simulink model "Dyn_Nonlinear_four"  (R2021a)
(part 6 of 7)

C(2,5) = 0.014*thetad1*cos(theta5)*sin(theta2) - 0.1*thetad5*cos(theta1) - 0.7*thetad4*sin(theta1) - 0.7*thetad5*sin(theta1) - 0.1*thetad4*cos(theta1) + 2.82*thetad4*cos(theta2)*sin(theta2) + 2.82*thetad5*cos(theta2)*sin(theta2) + 2.82*thetad4*cos(theta3)*sin(theta3) + 2.82*thetad5*cos(theta3)*sin(theta3) + 2.82*thetad4*cos(theta4)*sin(theta4) + 2.82*thetad5*cos(theta4)*sin(theta4) - 0.07*thetad1*sin(theta2)*sin(theta5) + 0.2*thetad4*cos(theta1)*cos(theta2)^2 + 0.2*thetad4*cos(theta1)*cos(theta3)^2 + 0.2*thetad5*cos(theta1)*cos(theta2)^2 + 0.2*thetad4*cos(theta1)*cos(theta4)^2 + 0.2*thetad5*cos(theta1)*cos(theta3)^2 + 0.2*thetad5*cos(theta1)*cos(theta4)^2 + 1.4*thetad4*cos(theta2)^2*sin(theta1) + 1.4*thetad4*cos(theta3)^2*sin(theta1) + 1.4*thetad5*cos(theta2)^2*sin(theta1) + 1.4*thetad4*cos(theta4)^2*sin(theta1) + 1.4*thetad5*cos(theta3)^2*sin(theta1) + 1.4*thetad5*cos(theta4)^2*sin(theta1) - 0.4*thetad4*cos(theta1)*cos(theta2)^2*cos(theta3)^2 - 0.4*thetad4*cos(theta1)*cos(theta2)^2*cos(theta4)^2 - 0.4*thetad5*cos(theta1)*cos(theta2)^2*cos(theta3)^2 - 0.4*thetad4*cos(theta1)*cos(theta3)^2*cos(theta4)^2 - 0.4*thetad5*cos(theta1)*cos(theta2)^2*cos(theta4)^2 - 0.4*thetad5*cos(theta1)*cos(theta3)^2*cos(theta4)^2 - 2.8*thetad4*cos(theta2)^2*cos(theta3)^2*sin(theta1) - 2.8*thetad4*cos(theta2)^2*cos(theta4)^2*sin(theta1) - 2.8*thetad5*cos(theta2)^2*cos(theta3)^2*sin(theta1) - 2.8*thetad4*cos(theta3)^2*cos(theta4)^2*sin(theta1) - 2.8*thetad5*cos(theta2)^2*cos(theta4)^2*sin(theta1) - 2.8*thetad5*cos(theta3)^2*cos(theta4)^2*sin(theta1) + 0.22*thetad1*cos(theta2)*cos(theta3)*cos(theta4) + 0.22*thetad2*cos(theta2)*cos(theta3)*cos(theta4) + 0.22*thetad3*cos(theta2)*cos(theta3)*cos(theta4) + 0.0728*thetad1*cos(theta2)*cos(theta3)*sin(theta4) + 0.0728*thetad1*cos(theta2)*cos(theta4)*sin(theta3) + 0.0728*thetad1*cos(theta3)*cos(theta4)*sin(theta2) + 0.014*thetad1*cos(theta2)*cos(theta5)*sin(theta3) + 0.014*thetad1*cos(theta3)*cos(theta5)*sin(theta2) - 0.22*thetad1*cos(theta2)*sin(theta3)*sin(theta4) - 0.22*thetad1*cos(theta3)*sin(theta2)*sin(theta4) - 0.22*thetad1*cos(theta4)*sin(theta2)*sin(theta3) - 0.07*thetad1*cos(theta2)*sin(theta3)*sin(theta5) - 0.07*thetad1*cos(theta3)*sin(theta2)*sin(theta5) - 0.22*thetad2*cos(theta2)*sin(theta3)*sin(theta4) - 0.22*thetad2*cos(theta3)*sin(theta2)*sin(theta4) - 0.22*thetad2*cos(theta4)*sin(theta2)*sin(theta3) - 0.22*thetad3*cos(theta2)*sin(theta3)*sin(theta4) - 0.22*thetad3*cos(theta3)*sin(theta2)*sin(theta4) - 0.22*thetad3*cos(theta4)*sin(theta2)*sin(theta3) - 0.0728*thetad1*sin(theta2)*sin(theta3)*sin(theta4) - 3.14*thetad4*cos(theta1)^2*cos(theta2)*sin(theta2) - 3.14*thetad5*cos(theta1)^2*cos(theta2)*sin(theta2) - 5.64*thetad4*cos(theta2)*cos(theta3)^2*sin(theta2) - 3.14*thetad4*cos(theta1)^2*cos(theta3)*sin(theta3) - 5.64*thetad4*cos(theta2)*cos(theta4)^2*sin(theta2) - 5.64*thetad4*cos(theta2)^2*cos(theta3)*sin(theta3) - 5.64*thetad5*cos(theta2)*cos(theta3)^2*sin(theta2) - 3.14*thetad5*cos(theta1)^2*cos(theta3)*sin(theta3) - 3.14*thetad4*cos(theta1)^2*cos(theta4)*sin(theta4) - 5.64*thetad5*cos(theta2)*cos(theta4)^2*sin(theta2) - 5.64*thetad5*cos(theta2)^2*cos(theta3)*sin(theta3) - 5.64*thetad4*cos(theta3)*cos(theta4)^2*sin(theta3) - 5.64*thetad4*cos(theta2)^2*cos(theta4)*sin(theta4) - 3.14*thetad5*cos(theta1)^2*cos(theta4)*sin(theta4) - 5.64*thetad4*cos(theta3)^2*cos(theta4)*sin(theta4) - 5.64*thetad5*cos(theta3)*cos(theta4)^2*sin(theta3) - 5.64*thetad5*cos(theta2)^2*cos(theta4)*sin(theta4) - 5.64*thetad5*cos(theta3)^2*cos(theta4)*sin(theta4) + 6.28*thetad4*cos(theta1)^2*cos(theta2)*cos(theta3)^2*sin(theta2) + 6.28*thetad4*cos(theta1)^2*cos(theta2)*cos(theta4)^2*sin(theta2) + 6.28*thetad4*cos(theta1)^2*cos(theta2)^2*cos(theta3)*sin(theta3) + 6.28*thetad5*cos(theta1)^2*cos(theta2)*cos(theta3)^2*sin(theta2) + 6.28*thetad5*cos(theta1)^2*cos(theta2)*cos(theta4)^2*sin(theta2) + 6.28*thetad5*cos(theta1)^2*cos(theta2)^2*cos(theta3)*sin(theta3) + 11.28*thetad4*cos(theta2)*cos(theta3)^2*cos(theta4)^2*sin(theta2) + 6.28*thetad4*cos(theta1)^2*cos(theta3)*cos(theta4)^2*sin(theta3) + 6.28*thetad4*cos(theta1)^2*cos(theta2)^2*cos(theta4)*sin(theta4) + 6.28*thetad4*cos(theta1)^2*cos(theta3)^2*cos(theta4)*sin(theta4) + 11.28*thetad4*cos(theta2)^2*cos(theta3)*cos(theta4)^2*sin(theta3) + 11.28*thetad5*cos(theta2)*cos(theta3)^2*cos(theta4)^2*sin(theta2) + 6.28*thetad5*cos(theta1)^2*cos(theta3)*cos(theta4)^2*sin(theta3) + 6.28*thetad5*cos(theta1)^2*cos(theta2)^2*cos(theta4)*sin(theta4) + 11.28*thetad4*cos(theta2)^2*cos(theta3)^2*cos(theta4)*sin(theta4) + 6.28*thetad5*cos(theta1)^2*cos(theta3)^2*cos(theta4)*sin(theta4) + 11.28*thetad5*cos(theta2)^2*cos(theta3)*cos(theta4)^2*sin(theta3) + 11.28*thetad5*cos(theta2)^2*cos(theta3)^2*cos(theta4)*sin(theta4) + 0.0098*thetad1*cos(theta2)*cos(theta3)*cos(theta4)*cos(theta5) - 0.35*thetad1*cos(theta1)*cos(theta2)*cos(theta3)*sin(theta4) - 0.35*thetad1*cos(theta1)*cos(theta2)*cos(theta4)*sin(theta3) - 0.35*thetad1*cos(theta1)*cos(theta3)*cos(theta4)*sin(theta2) - 0.35*thetad2*cos(theta1)*cos(theta2)*cos(theta3)*sin(theta4) - 0.35*thetad2*cos(theta1)*cos(theta2)*cos(theta4)*sin(theta3) - 0.35*thetad2*cos(theta1)*cos(theta3)*cos(theta4)*sin(theta2) - 0.35*thetad3*cos(theta1)*cos(theta2)*cos(theta3)*sin(theta4) - 0.35*thetad3*cos(theta1)*cos(theta2)*cos(theta4)*sin(theta3) - 0.35*thetad3*cos(theta1)*cos(theta3)*cos(theta4)*sin(theta2) - 0.049*thetad1*cos(theta2)*cos(theta3)*cos(theta4)*sin(theta5) + 0.8*thetad4*cos(theta1)*cos(theta2)^2*cos(theta3)^2*cos(theta4)^2 + 0.8*thetad5*cos(theta1)*cos(theta2)^2*cos(theta3)^2*cos(theta4)^2 - 0.88*thetad4*cos(theta1)*cos(theta2)*sin(theta1)*sin(theta2) + 0.05*thetad1*cos(theta2)*cos(theta3)*sin(theta1)*sin(theta4) + 0.05*thetad1*cos(theta2)*cos(theta4)*sin(theta1)*sin(theta3) + 0.05*thetad1*cos(theta3)*cos(theta4)*sin(theta1)*sin(theta2) - 0.88*thetad5*cos(theta1)*cos(theta2)*sin(theta1)*sin(theta2) + 0.05*thetad2*cos(theta2)*cos(theta3)*sin(theta1)*sin(theta4) + 0.05*thetad2*cos(theta2)*cos(theta4)*sin(theta1)*sin(theta3) + 0.05*thetad2*cos(theta3)*cos(theta4)*sin(theta1)*sin(theta2) - 0.88*thetad4*cos(theta1)*cos(theta3)*sin(theta1)*sin(theta3) + 0.05*thetad3*cos(theta2)*cos(theta3)*sin(theta1)*sin(theta4) + 0.05*thetad3*cos(theta2)*cos(theta4)*sin(theta1)*sin(theta3) + 0.05*thetad3*cos(theta3)*cos(theta4)*sin(theta1)*sin(theta2) - 0.88*thetad5*cos(theta1)*cos(theta3)*sin(theta1)*sin(theta3) - 0.88*thetad4*cos(theta1)*cos(theta4)*sin(theta1)*sin(theta4) - 0.0098*thetad1*cos(theta2)*cos(theta5)*sin(theta3)*sin(theta4) - 0.0098*thetad1*cos(theta3)*cos(theta5)*sin(theta2)*sin(theta4) - 0.0098*thetad1*cos(theta4)*cos(theta5)*sin(theta2)*sin(theta3) - 0.88*thetad5*cos(theta1)*cos(theta4)*sin(theta1)*sin(theta4) + 5.6*thetad4*cos(theta2)^2*cos(theta3)^2*cos(theta4)^2*sin(theta1) + 5.6*thetad5*cos(theta2)^2*cos(theta3)^2*cos(theta4)^2*sin(theta1) + 0.35*thetad1*cos(theta1)*sin(theta2)*sin(theta3)*sin(theta4) + 0.35*thetad2*cos(theta1)*sin(theta2)*sin(theta3)*sin(theta4) + 0.35*thetad3*cos(theta1)*sin(theta2)*sin(theta3)*sin(theta4) + 0.049*thetad1*cos(theta2)*sin(theta3)*sin(theta4)*sin(theta5) + 0.049*thetad1*cos(theta3)*sin(theta2)*sin(theta4)*sin(theta5) + 0.049*thetad1*cos(theta4)*sin(theta2)*sin(theta3)*sin(theta5) - 0.05*thetad1*sin(theta1)*sin(theta2)*sin(theta3)*sin(theta4) - 0.05*thetad2*sin(theta1)*sin(theta2)*sin(theta3)*sin(theta4) - 0.05*thetad3*sin(theta1)*sin(theta2)*sin(theta3)*sin(theta4) - 0.44*thetad1*cos(theta1)^2*cos(theta2)*cos(theta3)*cos(theta4) - 0.44*thetad2*cos(theta1)^2*cos(theta2)*cos(theta3)*cos(theta4) - 0.44*thetad3*cos(theta1)^2*cos(theta2)*cos(theta3)*cos(theta4) + 0.44*thetad1*cos(theta1)^2*cos(theta2)*sin(theta3)*sin(theta4) + 0.44*thetad1*cos(theta1)^2*cos(theta3)*sin(theta2)*sin(theta4) + 0.44*thetad1*cos(theta1)^2*cos(theta4)*sin(theta2)*sin(theta3) + 0.44*thetad2*cos(theta1)^2*cos(theta2)*sin(theta3)*sin(theta4) + 0.44*thetad2*cos(theta1)^2*cos(theta3)*sin(theta2)*sin(theta4) + 0.44*thetad2*cos(theta1)^2*cos(theta4)*sin(theta2)*sin(theta3) + 0.44*thetad3*cos(theta1)^2*cos(theta2)*sin(theta3)*sin(theta4) + 0.44*thetad3*cos(theta1)^2*cos(theta3)*sin(theta2)*sin(theta4) + 0.44*thetad3*cos(theta1)^2*cos(theta4)*sin(theta2)*sin(theta3) + 1.57*thetad1*cos(theta1)*cos(theta2)*cos(theta3)*cos(theta4)*sin(theta1) + 1.57*thetad2*cos(theta1)*cos(theta2)*cos(theta3)*cos(theta4)*sin(theta1) + 1.57*thetad3*cos(theta1)*cos(theta2)*cos(theta3)*cos(theta4)*sin(theta1) + 0.4*thetad4*cos(theta1)*cos(theta2)*cos(theta3)*sin(theta2)*sin(theta3) + 0.4*thetad5*cos(theta1)*cos(theta2)*cos(theta3)*sin(theta2)*sin(theta3) + 0.4*thetad4*cos(theta1)*cos(theta2)*cos(theta4)*sin(theta2)*sin(theta4) + 0.4*thetad5*cos(theta1)*cos(theta2)*cos(theta4)*sin(theta2)*sin(theta4) + 0.4*thetad4*cos(theta1)*cos(theta3)*cos(theta4)*sin(theta3)*sin(theta4) + 0.4*thetad5*cos(theta1)*cos(theta3)*cos(theta4)*sin(theta3)*sin(theta4) - 12.56*thetad4*cos(theta1)^2*cos(theta2)*cos(theta3)^2*cos(theta4)^2*sin(theta2) - 12.56*thetad4*cos(theta1)^2*cos(theta2)^2*cos(theta3)*cos(theta4)^2*sin(theta3) - 12.56*thetad5*cos(theta1)^2*cos(theta2)*cos(theta3)^2*cos(theta4)^2*sin(theta2) - 12.56*thetad4*cos(theta1)^2*cos(theta2)^2*cos(theta3)^2*cos(theta4)*sin(theta4) - 12.56*thetad5*cos(theta1)^2*cos(theta2)^2*cos(theta3)*cos(theta4)^2*sin(theta3) - 12.56*thetad5*cos(theta1)^2*cos(theta2)^2*cos(theta3)^2*cos(theta4)*sin(theta4) - 1.57*thetad1*cos(theta1)*cos(theta2)*sin(theta1)*sin(theta3)*sin(theta4) - 1.57*thetad1*cos(theta1)*cos(theta3)*sin(theta1)*sin(theta2)*sin(theta4) - 1.57*thetad1*cos(theta1)*cos(theta4)*sin(theta1)*sin(theta2)*sin(theta3) - 1.57*thetad2*cos(theta1)*cos(theta2)*sin(theta1)*sin(theta3)*sin(theta4) - 1.57*thetad2*cos(theta1)*cos(theta3)*sin(theta1)*sin(theta2)*sin(theta4) - 1.57*thetad2*cos(theta1)*cos(theta4)*sin(theta1)*sin(theta2)*sin(theta3) - 1.57*thetad3*cos(theta1)*cos(theta2)*sin(theta1)*sin(theta3)*sin(theta4) - 1.57*thetad3*cos(theta1)*cos(theta3)*sin(theta1)*sin(theta2)*sin(theta4) - 1.57*thetad3*cos(theta1)*cos(theta4)*sin(theta1)*sin(theta2)*sin(theta3) + 2.8*thetad4*cos(theta2)*cos(theta3)*sin(theta1)*sin(theta2)*sin(theta3) + 2.8*thetad5*cos(theta2)*cos(theta3)*sin(theta1)*sin(theta2)*sin(theta3) + 2.8*thetad4*cos(theta2)*cos(theta4)*sin(theta1)*sin(theta2)*sin(theta4) + 2.8*thetad5*cos(theta2)*cos(theta4)*sin(theta1)*sin(theta2)*sin(theta4) + 2.8*thetad4*cos(theta3)*cos(theta4)*sin(theta1)*sin(theta3)*sin(theta4) + 2.8*thetad5*cos(theta3)*cos(theta4)*sin(theta1)*sin(theta3)*sin(theta4) + 1.76*thetad4*cos(theta1)*cos(theta2)*cos(theta3)^2*sin(theta1)*sin(theta2) + 1.76*thetad4*cos(theta1)*cos(theta2)*cos(theta4)^2*sin(theta1)*sin(theta2) + 1.76*thetad4*cos(theta1)*cos(theta2)^2*cos(theta3)*sin(theta1)*sin(theta3) + 1.76*thetad5*cos(theta1)*cos(theta2)*cos(theta3)^2*sin(theta1)*sin(theta2) + 1.76*thetad5*cos(theta1)*cos(theta2)*cos(theta4)^2*sin(theta1)*sin(theta2) + 1.76*thetad5*cos(theta1)*cos(theta2)^2*cos(theta3)*sin(theta1)*sin(theta3) + 1.76*thetad4*cos(theta1)*cos(theta3)*cos(theta4)^2*sin(theta1)*sin(theta3) + 1.76*thetad4*cos(theta1)*cos(theta2)^2*cos(theta4)*sin(theta1)*sin(theta4) + 1.76*thetad4*cos(theta1)*cos(theta3)^2*cos(theta4)*sin(theta1)*sin(theta4) + 1.76*thetad5*cos(theta1)*cos(theta3)*cos(theta4)^2*sin(theta1)*sin(theta3) + 1.76*thetad5*cos(theta1)*cos(theta2)^2*cos(theta4)*sin(theta1)*sin(theta4) + 1.76*thetad5*cos(theta1)*cos(theta3)^2*cos(theta4)*sin(theta1)*sin(theta4) - 11.28*thetad4*cos(theta2)*cos(theta3)*cos(theta4)*sin(theta2)*sin(theta3)*sin(theta4) - 11.28*thetad5*cos(theta2)*cos(theta3)*cos(theta4)*sin(theta2)*sin(theta3)*sin(theta4) - 0.8*thetad4*cos(theta1)*cos(theta2)*cos(theta3)*cos(theta4)^2*sin(theta2)*sin(theta3) - 0.8*thetad4*cos(theta1)*cos(theta2)*cos(theta3)^2*cos(theta4)*sin(theta2)*sin(theta4) - 0.8*thetad5*cos(theta1)*cos(theta2)*cos(theta3)*cos(theta4)^2*sin(theta2)*sin(theta3) - 0.8*thetad4*cos(theta1)*cos(theta2)^2*cos(theta3)*cos(theta4)*sin(theta3)*sin(theta4) - 0.8*thetad5*cos(theta1)*cos(theta2)*cos(theta3)^2*cos(theta4)*sin(theta2)*sin(theta4) - 0.8*thetad5*cos(theta1)*cos(theta2)^2*cos(theta3)*cos(theta4)*sin(theta3)*sin(theta4) - 5.6*thetad4*cos(theta2)*cos(theta3)*cos(theta4)^2*sin(theta1)*sin(theta2)*sin(theta3) - 5.6*thetad4*cos(theta2)*cos(theta3)^2*cos(theta4)*sin(theta1)*sin(theta2)*sin(theta4) - 5.6*thetad5*cos(theta2)*cos(theta3)*cos(theta4)^2*sin(theta1)*sin(theta2)*sin(theta3) - 5.6*thetad4*cos(theta2)^2*cos(theta3)*cos(theta4)*sin(theta1)*sin(theta3)*sin(theta4) - 5.6*thetad5*cos(theta2)*cos(theta3)^2*cos(theta4)*sin(theta1)*sin(theta2)*sin(theta4) - 5.6*thetad5*cos(theta2)^2*cos(theta3)*cos(theta4)*sin(theta1)*sin(theta3)*sin(theta4) - 3.52*thetad4*cos(theta1)*cos(theta2)*cos(theta3)^2*cos(theta4)^2*sin(theta1)*sin(theta2) - 3.52*thetad4*cos(theta1)*cos(theta2)^2*cos(theta3)*cos(theta4)^2*sin(theta1)*sin(theta3) - 3.52*thetad5*cos(theta1)*cos(theta2)*cos(theta3)^2*cos(theta4)^2*sin(theta1)*sin(theta2) - 3.52*thetad4*cos(theta1)*cos(theta2)^2*cos(theta3)^2*cos(theta4)*sin(theta1)*sin(theta4) - 3.52*thetad5*cos(theta1)*cos(theta2)^2*cos(theta3)*cos(theta4)^2*sin(theta1)*sin(theta3) - 3.52*thetad5*cos(theta1)*cos(theta2)^2*cos(theta3)^2*cos(theta4)*sin(theta1)*sin(theta4) + 12.56*thetad4*cos(theta1)^2*cos(theta2)*cos(theta3)*cos(theta4)*sin(theta2)*sin(theta3)*sin(theta4) + 12.56*thetad5*cos(theta1)^2*cos(theta2)*cos(theta3)*cos(theta4)*sin(theta2)*sin(theta3)*sin(theta4) + 3.52*thetad4*cos(theta1)*cos(theta2)*cos(theta3)*cos(theta4)*sin(theta1)*sin(theta2)*sin(theta3)*sin(theta4) + 3.52*thetad5*cos(theta1)*cos(theta2)*cos(theta3)*cos(theta4)*sin(theta1)*sin(theta2)*sin(theta3)*sin(theta4) ;
C(3,1) = 0.367108*thetad1 - 0.734216*thetad1*cos(theta2)^2 - 0.734216*thetad1*cos(theta3)^2 + 0.206584*thetad1*cos(theta4)^2 + 0.4018*thetad1*cos(theta4) - 0.0196*thetad1*cos(theta5) + 0.1666*thetad1*sin(theta4) + 0.098*thetad1*sin(theta5) + 1.468432*thetad1*cos(theta2)^2*cos(theta3)^2 - 0.413168*thetad1*cos(theta2)^2*cos(theta4)^2 - 0.413168*thetad1*cos(theta3)^2*cos(theta4)^2 - 0.4875*thetad2*cos(theta2)*cos(theta3) - 0.4875*thetad3*cos(theta2)*cos(theta3) - 0.435656*thetad1*cos(theta2)*sin(theta2) - 0.435656*thetad1*cos(theta3)*sin(theta3) - 0.150528*thetad2*cos(theta2)*sin(theta3) - 0.150528*thetad2*cos(theta3)*sin(theta2) - 0.150528*thetad3*cos(theta2)*sin(theta3) - 0.150528*thetad3*cos(theta3)*sin(theta2) - 0.060312*thetad1*cos(theta4)*sin(theta4) + 0.028*thetad1*cos(theta5)*sin(theta4) + 0.4875*thetad2*sin(theta2)*sin(theta3) + 0.4875*thetad3*sin(theta2)*sin(theta3) - 0.14*thetad1*sin(theta4)*sin(theta5) + 0.3136*thetad1*cos(theta2)^2*cos(theta3) - 0.8036*thetad1*cos(theta2)^2*cos(theta4) + 0.0392*thetad1*cos(theta2)^2*cos(theta5) - 0.8036*thetad1*cos(theta3)^2*cos(theta4) + 0.0392*thetad1*cos(theta3)^2*cos(theta5) + 0.0392*thetad1*cos(theta4)^2*cos(theta5) + 0.87*thetad1*cos(theta2)^2*sin(theta3) - 0.3332*thetad1*cos(theta2)^2*sin(theta4) - 0.196*thetad1*cos(theta2)^2*sin(theta5) - 0.3332*thetad1*cos(theta3)^2*sin(theta4) - 0.196*thetad1*cos(theta3)^2*sin(theta5) - 0.196*thetad1*cos(theta4)^2*sin(theta5) + 1.6072*thetad1*cos(theta2)^2*cos(theta3)^2*cos(theta4) - 0.0784*thetad1*cos(theta2)^2*cos(theta3)^2*cos(theta5) - 0.0784*thetad1*cos(theta2)^2*cos(theta4)^2*cos(theta5) - 0.0784*thetad1*cos(theta3)^2*cos(theta4)^2*cos(theta5) + 0.6664*thetad1*cos(theta2)^2*cos(theta3)^2*sin(theta4) + 0.392*thetad1*cos(theta2)^2*cos(theta3)^2*sin(theta5) + 0.392*thetad1*cos(theta2)^2*cos(theta4)^2*sin(theta5) + 0.392*thetad1*cos(theta3)^2*cos(theta4)^2*sin(theta5) - 0.190918*thetad2*cos(theta2)*cos(theta3)*cos(theta4) - 0.07*thetad2*cos(theta2)*cos(theta3)*cos(theta5) - 0.190918*thetad3*cos(theta2)*cos(theta3)*cos(theta4) - 0.07*thetad3*cos(theta2)*cos(theta3)*cos(theta5) + 0.249082*thetad4*cos(theta2)*cos(theta3)*cos(theta4) + 0.22*thetad5*cos(theta2)*cos(theta3)*cos(theta4) + 0.87*thetad1*cos(theta2)*cos(theta3)*sin(theta2) - 0.3332*thetad1*cos(theta2)*cos(theta4)*sin(theta2) - 0.3332*thetad1*cos(theta3)*cos(theta4)*sin(theta3) + 0.373674*thetad2*cos(theta2)*cos(theta3)*sin(theta4) + 0.373674*thetad2*cos(theta2)*cos(theta4)*sin(theta3) + 0.373674*thetad2*cos(theta3)*cos(theta4)*sin(theta2) - 0.014*thetad2*cos(theta2)*cos(theta3)*sin(theta5) + 0.373674*thetad3*cos(theta2)*cos(theta3)*sin(theta4) + 0.373674*thetad3*cos(theta2)*cos(theta4)*sin(theta3) + 0.373674*thetad3*cos(theta3)*cos(theta4)*sin(theta2) - 0.014*thetad3*cos(theta2)*cos(theta3)*sin(theta5) + 0.373674*thetad4*cos(theta2)*cos(theta3)*sin(theta4) + 0.373674*thetad4*cos(theta2)*cos(theta4)*sin(theta3) + 0.373674*thetad4*cos(theta3)*cos(theta4)*sin(theta2) + 0.0728*thetad5*cos(theta2)*cos(theta3)*sin(theta4) + 0.0728*thetad5*cos(theta2)*cos(theta4)*sin(theta3) + 0.0728*thetad5*cos(theta3)*cos(theta4)*sin(theta2) + 0.014*thetad5*cos(theta2)*cos(theta5)*sin(theta3) + 0.014*thetad5*cos(theta3)*cos(theta5)*sin(theta2) + 0.826336*thetad1*cos(theta2)^2*cos(theta3)^2*cos(theta4)^2 - 0.3136*thetad1*cos(theta2)*sin(theta2)*sin(theta3) + 0.8036*thetad1*cos(theta2)*sin(theta2)*sin(theta4) + 0.8036*thetad1*cos(theta3)*sin(theta3)*sin(theta4) + 0.190918*thetad2*cos(theta2)*sin(theta3)*sin(theta4) + 0.190918*thetad2*cos(theta3)*sin(theta2)*sin(theta4) + 0.190918*thetad2*cos(theta4)*sin(theta2)*sin(theta3) + 0.07*thetad2*cos(theta5)*sin(theta2)*sin(theta3) + 0.190918*thetad3*cos(theta2)*sin(theta3)*sin(theta4) + 0.190918*thetad3*cos(theta3)*sin(theta2)*sin(theta4) + 0.190918*thetad3*cos(theta4)*sin(theta2)*sin(theta3) + 0.07*thetad3*cos(theta5)*sin(theta2)*sin(theta3) - 0.249082*thetad4*cos(theta2)*sin(theta3)*sin(theta4) - 0.249082*thetad4*cos(theta3)*sin(theta2)*sin(theta4) - 0.249082*thetad4*cos(theta4)*sin(theta2)*sin(theta3) - 0.22*thetad5*cos(theta2)*sin(theta3)*sin(theta4) - 0.22*thetad5*cos(theta3)*sin(theta2)*sin(theta4) - 0.22*thetad5*cos(theta4)*sin(theta2)*sin(theta3) - 0.07*thetad5*cos(theta2)*sin(theta3)*sin(theta5) - 0.07*thetad5*cos(theta3)*sin(theta2)*sin(theta5) - 0.373674*thetad2*sin(theta2)*sin(theta3)*sin(theta4) + 0.014*thetad2*sin(theta2)*sin(theta3)*sin(theta5) - 0.373674*thetad3*sin(theta2)*sin(theta3)*sin(theta4) + 0.014*thetad3*sin(theta2)*sin(theta3)*sin(theta5) - 0.373674*thetad4*sin(theta2)*sin(theta3)*sin(theta4) - 0.0728*thetad5*sin(theta2)*sin(theta3)*sin(theta4) + 0.4018*thetad1*cos(theta2)^2*cos(theta3)*cos(theta4) + 0.871312*thetad1*cos(theta2)*cos(theta3)^2*sin(theta2) + 0.120624*thetad1*cos(theta2)*cos(theta4)^2*sin(theta2) + 0.871312*thetad1*cos(theta2)^2*cos(theta3)*sin(theta3) - 0.1344*thetad1*cos(theta2)*cos(theta5)^2*sin(theta2) + 0.1666*thetad1*cos(theta2)^2*cos(theta3)*sin(theta4) + 0.1666*thetad1*cos(theta2)^2*cos(theta4)*sin(theta3) + 0.120624*thetad1*cos(theta3)*cos(theta4)^2*sin(theta3) + 0.120624*thetad1*cos(theta2)^2*cos(theta4)*sin(theta4) - 0.1344*thetad1*cos(theta3)*cos(theta5)^2*sin(theta3) - 0.056*thetad1*cos(theta2)^2*cos(theta5)*sin(theta4) + 0.120624*thetad1*cos(theta3)^2*cos(theta4)*sin(theta4) - 0.056*thetad1*cos(theta3)^2*cos(theta5)*sin(theta4) - 0.1344*thetad1*cos(theta4)*cos(theta5)^2*sin(theta4) - 0.4018*thetad1*cos(theta2)^2*sin(theta3)*sin(theta4) + 0.28*thetad1*cos(theta2)^2*sin(theta4)*sin(theta5) + 0.28*thetad1*cos(theta3)^2*sin(theta4)*sin(theta5) - 0.241248*thetad1*cos(theta2)*cos(theta3)^2*cos(theta4)^2*sin(theta2) + 0.2688*thetad1*cos(theta2)*cos(theta3)^2*cos(theta5)^2*sin(theta2) - 0.241248*thetad1*cos(theta2)^2*cos(theta3)*cos(theta4)^2*sin(theta3) + 0.2688*thetad1*cos(theta2)*cos(theta4)^2*cos(theta5)^2*sin(theta2) + 0.2688*thetad1*cos(theta2)^2*cos(theta3)*cos(theta5)^2*sin(theta3) - 0.241248*thetad1*cos(theta2)^2*cos(theta3)^2*cos(theta4)*sin(theta4) + 0.112*thetad1*cos(theta2)^2*cos(theta3)^2*cos(theta5)*sin(theta4) + 0.2688*thetad1*cos(theta3)*cos(theta4)^2*cos(theta5)^2*sin(theta3) + 0.2688*thetad1*cos(theta2)^2*cos(theta4)*cos(theta5)^2*sin(theta4) + 0.2688*thetad1*cos(theta3)^2*cos(theta4)*cos(theta5)^2*sin(theta4) - 0.56*thetad1*cos(theta2)^2*cos(theta3)^2*sin(theta4)*sin(theta5) + 0.0098*thetad5*cos(theta2)*cos(theta3)*cos(theta4)*cos(theta5) + 0.1666*thetad1*cos(theta2)*cos(theta3)*cos(theta4)*sin(theta2) - 0.056*thetad1*cos(theta2)*cos(theta4)*cos(theta5)*sin(theta2) - 0.7*thetad4*cos(theta1)*cos(theta2)*cos(theta3)*sin(theta4) - 0.7*thetad4*cos(theta1)*cos(theta2)*cos(theta4)*sin(theta3) - 0.7*thetad4*cos(theta1)*cos(theta3)*cos(theta4)*sin(theta2) - 0.35*thetad5*cos(theta1)*cos(theta2)*cos(theta3)*sin(theta4) - 0.35*thetad5*cos(theta1)*cos(theta2)*cos(theta4)*sin(theta3) - 0.35*thetad5*cos(theta1)*cos(theta3)*cos(theta4)*sin(theta2) - 0.056*thetad1*cos(theta3)*cos(theta4)*cos(theta5)*sin(theta3) + 0.049*thetad2*cos(theta2)*cos(theta3)*cos(theta5)*sin(theta4) + 0.049*thetad2*cos(theta2)*cos(theta4)*cos(theta5)*sin(theta3) + 0.049*thetad2*cos(theta3)*cos(theta4)*cos(theta5)*sin(theta2) + 0.049*thetad3*cos(theta2)*cos(theta3)*cos(theta5)*sin(theta4) + 0.049*thetad3*cos(theta2)*cos(theta4)*cos(theta5)*sin(theta3) + 0.049*thetad3*cos(theta3)*cos(theta4)*cos(theta5)*sin(theta2) + 0.049*thetad4*cos(theta2)*cos(theta3)*cos(theta5)*sin(theta4) + 0.049*thetad4*cos(theta2)*cos(theta4)*cos(theta5)*sin(theta3) + 0.049*thetad4*cos(theta3)*cos(theta4)*cos(theta5)*sin(theta2) - 0.049*thetad5*cos(theta2)*cos(theta3)*cos(theta4)*sin(theta5) + 0.1568*thetad1*cos(theta2)^2*cos(theta3)^2*cos(theta4)^2*cos(theta5) - 1.468432*thetad1*cos(theta2)*cos(theta3)*sin(theta2)*sin(theta3) - 0.4018*thetad1*cos(theta2)*cos(theta3)*sin(theta2)*sin(theta4) - 0.4018*thetad1*cos(theta2)*cos(theta4)*sin(theta2)*sin(theta3) + 0.413168*thetad1*cos(theta2)*cos(theta4)*sin(theta2)*sin(theta4) + 0.28*thetad1*cos(theta2)*cos(theta4)*sin(theta2)*sin(theta5) + 0.1*thetad4*cos(theta2)*cos(theta3)*sin(theta1)*sin(theta4) + 0.1*thetad4*cos(theta2)*cos(theta4)*sin(theta1)*sin(theta3) + 0.1*thetad4*cos(theta3)*cos(theta4)*sin(theta1)*sin(theta2) - 0.056*thetad1*cos(theta2)*cos(theta5)*sin(theta2)*sin(theta5) + 0.413168*thetad1*cos(theta3)*cos(theta4)*sin(theta3)*sin(theta4) + 0.05*thetad5*cos(theta2)*cos(theta3)*sin(theta1)*sin(theta4) + 0.05*thetad5*cos(theta2)*cos(theta4)*sin(theta1)*sin(theta3) + 0.05*thetad5*cos(theta3)*cos(theta4)*sin(theta1)*sin(theta2) + 0.28*thetad1*cos(theta3)*cos(theta4)*sin(theta3)*sin(theta5) + 0.0098*thetad2*cos(theta2)*cos(theta3)*sin(theta4)*sin(theta5) + 0.0098*thetad2*cos(theta2)*cos(theta4)*sin(theta3)*sin(theta5) + 0.0098*thetad2*cos(theta3)*cos(theta4)*sin(theta2)*sin(theta5) - 0.056*thetad1*cos(theta3)*cos(theta5)*sin(theta3)*sin(theta5) + 0.0098*thetad3*cos(theta2)*cos(theta3)*sin(theta4)*sin(theta5) + 0.0098*thetad3*cos(theta2)*cos(theta4)*sin(theta3)*sin(theta5) + 0.0098*thetad3*cos(theta3)*cos(theta4)*sin(theta2)*sin(theta5) + 0.0098*thetad4*cos(theta2)*cos(theta3)*sin(theta4)*sin(theta5) + 0.0098*thetad4*cos(theta2)*cos(theta4)*sin(theta3)*sin(theta5) + 0.0098*thetad4*cos(theta3)*cos(theta4)*sin(theta2)*sin(theta5) - 0.056*thetad1*cos(theta4)*cos(theta5)*sin(theta4)*sin(theta5) - 0.0098*thetad5*cos(theta2)*cos(theta5)*sin(theta3)*sin(theta4) - 0.0098*thetad5*cos(theta3)*cos(theta5)*sin(theta2)*sin(theta4) - 0.0098*thetad5*cos(theta4)*cos(theta5)*sin(theta2)*sin(theta3) - 0.784*thetad1*cos(theta2)^2*cos(theta3)^2*cos(theta4)^2*sin(theta5) - 0.1666*thetad1*cos(theta2)*sin(theta2)*sin(theta3)*sin(theta4) + 0.7*thetad4*cos(theta1)*sin(theta2)*sin(theta3)*sin(theta4) + 0.35*thetad5*cos(theta1)*sin(theta2)*sin(theta3)*sin(theta4) - 0.049*thetad2*cos(theta5)*sin(theta2)*sin(theta3)*sin(theta4) - 0.049*thetad3*cos(theta5)*sin(theta2)*sin(theta3)*sin(theta4) - 0.049*thetad4*cos(theta5)*sin(theta2)*sin(theta3)*sin(theta4) + 0.049*thetad5*cos(theta2)*sin(theta3)*sin(theta4)*sin(theta5) + 0.049*thetad5*cos(theta3)*sin(theta2)*sin(theta4)*sin(theta5) + 0.049*thetad5*cos(theta4)*sin(theta2)*sin(theta3)*sin(theta5) - 0.1*thetad4*sin(theta1)*sin(theta2)*sin(theta3)*sin(theta4) - 0.05*thetad5*sin(theta1)*sin(theta2)*sin(theta3)*sin(theta4) - 0.0098*thetad2*sin(theta2)*sin(theta3)*sin(theta4)*sin(theta5) - 0.0098*thetad3*sin(theta2)*sin(theta3)*sin(theta4)*sin(theta5) - 0.0098*thetad4*sin(theta2)*sin(theta3)*sin(theta4)*sin(theta5) - 0.88*thetad4*cos(theta1)^2*cos(theta2)*cos(theta3)*cos(theta4) - 0.44*thetad5*cos(theta1)^2*cos(theta2)*cos(theta3)*cos(theta4) - 0.028*thetad2*cos(theta2)*cos(theta3)*cos(theta4)*cos(theta5)^2 - 0.028*thetad3*cos(theta2)*cos(theta3)*cos(theta4)*cos(theta5)^2 - 0.028*thetad4*cos(theta2)*cos(theta3)*cos(theta4)*cos(theta5)^2 + 0.6664*thetad1*cos(theta2)*cos(theta3)^2*cos(theta4)*sin(theta2) + 0.6664*thetad1*cos(theta2)^2*cos(theta3)*cos(theta4)*sin(theta3) + 0.028*thetad1*cos(theta2)^2*cos(theta3)*cos(theta5)*sin(theta4) + 0.028*thetad1*cos(theta2)^2*cos(theta4)*cos(theta5)*sin(theta3) - 1.6072*thetad1*cos(theta2)*cos(theta3)^2*sin(theta2)*sin(theta4) - 1.6072*thetad1*cos(theta2)^2*cos(theta3)*sin(theta3)*sin(theta4) + 0.88*thetad4*cos(theta1)^2*cos(theta2)*sin(theta3)*sin(theta4) + 0.88*thetad4*cos(theta1)^2*cos(theta3)*sin(theta2)*sin(theta4) + 0.88*thetad4*cos(theta1)^2*cos(theta4)*sin(theta2)*sin(theta3) - 0.14*thetad1*cos(theta2)^2*cos(theta3)*sin(theta4)*sin(theta5) - 0.14*thetad1*cos(theta2)^2*cos(theta4)*sin(theta3)*sin(theta5) + 0.44*thetad5*cos(theta1)^2*cos(theta2)*sin(theta3)*sin(theta4) + 0.44*thetad5*cos(theta1)^2*cos(theta3)*sin(theta2)*sin(theta4) + 0.44*thetad5*cos(theta1)^2*cos(theta4)*sin(theta2)*sin(theta3) + 0.028*thetad2*cos(theta2)*cos(theta5)^2*sin(theta3)*sin(theta4) + 0.028*thetad2*cos(theta3)*cos(theta5)^2*sin(theta2)*sin(theta4) + 0.028*thetad2*cos(theta4)*cos(theta5)^2*sin(theta2)*sin(theta3) + 0.028*thetad3*cos(theta2)*cos(theta5)^2*sin(theta3)*sin(theta4) + 0.028*thetad3*cos(theta3)*cos(theta5)^2*sin(theta2)*sin(theta4) + 0.028*thetad3*cos(theta4)*cos(theta5)^2*sin(theta2)*sin(theta3) + 0.028*thetad4*cos(theta2)*cos(theta5)^2*sin(theta3)*sin(theta4) + 0.028*thetad4*cos(theta3)*cos(theta5)^2*sin(theta2)*sin(theta4) + 0.028*thetad4*cos(theta4)*cos(theta5)^2*sin(theta2)*sin(theta3) + 3.14*thetad4*cos(theta1)*cos(theta2)*cos(theta3)*cos(theta4)*sin(theta1) + 1.57*thetad5*cos(theta1)*cos(theta2)*cos(theta3)*cos(theta4)*sin(theta1) + 0.028*thetad1*cos(theta2)*cos(theta3)*cos(theta4)*cos(theta5)*sin(theta2) + 0.0672*thetad2*cos(theta2)*cos(theta3)*cos(theta4)*cos(theta5)*sin(theta5) + 0.0672*thetad3*cos(theta2)*cos(theta3)*cos(theta4)*cos(theta5)*sin(theta5) + 0.0672*thetad4*cos(theta2)*cos(theta3)*cos(theta4)*cos(theta5)*sin(theta5) - 1.6072*thetad1*cos(theta2)*cos(theta3)*cos(theta4)*sin(theta2)*sin(theta3) + 0.0784*thetad1*cos(theta2)*cos(theta3)*cos(theta5)*sin(theta2)*sin(theta3) - 0.14*thetad1*cos(theta2)*cos(theta3)*cos(theta4)*sin(theta2)*sin(theta5) + 0.0784*thetad1*cos(theta2)*cos(theta4)*cos(theta5)*sin(theta2)*sin(theta4) + 0.0784*thetad1*cos(theta3)*cos(theta4)*cos(theta5)*sin(theta3)*sin(theta4) - 0.5376*thetad1*cos(theta2)*cos(theta3)^2*cos(theta4)^2*cos(theta5)^2*sin(theta2) - 0.5376*thetad1*cos(theta2)^2*cos(theta3)*cos(theta4)^2*cos(theta5)^2*sin(theta3) - 0.5376*thetad1*cos(theta2)^2*cos(theta3)^2*cos(theta4)*cos(theta5)^2*sin(theta4) - 0.6664*thetad1*cos(theta2)*cos(theta3)*sin(theta2)*sin(theta3)*sin(theta4) - 3.14*thetad4*cos(theta1)*cos(theta2)*sin(theta1)*sin(theta3)*sin(theta4) - 3.14*thetad4*cos(theta1)*cos(theta3)*sin(theta1)*sin(theta2)*sin(theta4) - 3.14*thetad4*cos(theta1)*cos(theta4)*sin(theta1)*sin(theta2)*sin(theta3) - 0.392*thetad1*cos(theta2)*cos(theta3)*sin(theta2)*sin(theta3)*sin(theta5) - 1.57*thetad5*cos(theta1)*cos(theta2)*sin(theta1)*sin(theta3)*sin(theta4) - 1.57*thetad5*cos(theta1)*cos(theta3)*sin(theta1)*sin(theta2)*sin(theta4) - 1.57*thetad5*cos(theta1)*cos(theta4)*sin(theta1)*sin(theta2)*sin(theta3) - 0.028*thetad1*cos(theta2)*cos(theta5)*sin(theta2)*sin(theta3)*sin(theta4) - 0.392*thetad1*cos(theta2)*cos(theta4)*sin(theta2)*sin(theta4)*sin(theta5) - 0.392*thetad1*cos(theta3)*cos(theta4)*sin(theta3)*sin(theta4)*sin(theta5) - 0.0672*thetad2*cos(theta2)*cos(theta5)*sin(theta3)*sin(theta4)*sin(theta5) - 0.0672*thetad2*cos(theta3)*cos(theta5)*sin(theta2)*sin(theta4)*sin(theta5) - 0.0672*thetad2*cos(theta4)*cos(theta5)*sin(theta2)*sin(theta3)*sin(theta5) - 0.0672*thetad3*cos(theta2)*cos(theta5)*sin(theta3)*sin(theta4)*sin(theta5) - 0.0672*thetad3*cos(theta3)*cos(theta5)*sin(theta2)*sin(theta4)*sin(theta5) - 0.0672*thetad3*cos(theta4)*cos(theta5)*sin(theta2)*sin(theta3)*sin(theta5) - 0.0672*thetad4*cos(theta2)*cos(theta5)*sin(theta3)*sin(theta4)*sin(theta5) - 0.0672*thetad4*cos(theta3)*cos(theta5)*sin(theta2)*sin(theta4)*sin(theta5) - 0.0672*thetad4*cos(theta4)*cos(theta5)*sin(theta2)*sin(theta3)*sin(theta5) + 0.14*thetad1*cos(theta2)*sin(theta2)*sin(theta3)*sin(theta4)*sin(theta5) + 0.112*thetad1*cos(theta2)*cos(theta3)^2*cos(theta4)*cos(theta5)*sin(theta2) + 0.112*thetad1*cos(theta2)^2*cos(theta3)*cos(theta4)*cos(theta5)*sin(theta3) - 0.826336*thetad1*cos(theta2)*cos(theta3)*cos(theta4)^2*sin(theta2)*sin(theta3) - 0.826336*thetad1*cos(theta2)*cos(theta3)^2*cos(theta4)*sin(theta2)*sin(theta4) - 0.56*thetad1*cos(theta2)*cos(theta3)^2*cos(theta4)*sin(theta2)*sin(theta5) - 0.826336*thetad1*cos(theta2)^2*cos(theta3)*cos(theta4)*sin(theta3)*sin(theta4) + 0.112*thetad1*cos(theta2)*cos(theta3)^2*cos(theta5)*sin(theta2)*sin(theta5) - 0.56*thetad1*cos(theta2)^2*cos(theta3)*cos(theta4)*sin(theta3)*sin(theta5) + 0.112*thetad1*cos(theta2)*cos(theta4)^2*cos(theta5)*sin(theta2)*sin(theta5) + 0.112*thetad1*cos(theta2)^2*cos(theta3)*cos(theta5)*sin(theta3)*sin(theta5) + 0.112*thetad1*cos(theta3)*cos(theta4)^2*cos(theta5)*sin(theta3)*sin(theta5) + 0.112*thetad1*cos(theta2)^2*cos(theta4)*cos(theta5)*sin(theta4)*sin(theta5) + 0.112*thetad1*cos(theta3)^2*cos(theta4)*cos(theta5)*sin(theta4)*sin(theta5) + 0.241248*thetad1*cos(theta2)*cos(theta3)*cos(theta4)*sin(theta2)*sin(theta3)*sin(theta4) - 0.112*thetad1*cos(theta2)*cos(theta3)*cos(theta5)*sin(theta2)*sin(theta3)*sin(theta4) + 0.56*thetad1*cos(theta2)*cos(theta3)*sin(theta2)*sin(theta3)*sin(theta4)*sin(theta5) - 0.1568*thetad1*cos(theta2)*cos(theta3)*cos(theta4)^2*cos(theta5)*sin(theta2)*sin(theta3) - 0.1568*thetad1*cos(theta2)*cos(theta3)^2*cos(theta4)*cos(theta5)*sin(theta2)*sin(theta4) - 0.1568*thetad1*cos(theta2)^2*cos(theta3)*cos(theta4)*cos(theta5)*sin(theta3)*sin(theta4) + 0.784*thetad1*cos(theta2)*cos(theta3)*cos(theta4)^2*sin(theta2)*sin(theta3)*sin(theta5) + 0.784*thetad1*cos(theta2)*cos(theta3)^2*cos(theta4)*sin(theta2)*sin(theta4)*sin(theta5) + 0.784*thetad1*cos(theta2)^2*cos(theta3)*cos(theta4)*sin(theta3)*sin(theta4)*sin(theta5) - 0.224*thetad1*cos(theta2)*cos(theta3)^2*cos(theta4)^2*cos(theta5)*sin(theta2)*sin(theta5) - 0.224*thetad1*cos(theta2)^2*cos(theta3)*cos(theta4)^2*cos(theta5)*sin(theta3)*sin(theta5) - 0.224*thetad1*cos(theta2)^2*cos(theta3)^2*cos(theta4)*cos(theta5)*sin(theta4)*sin(theta5) + 0.5376*thetad1*cos(theta2)*cos(theta3)*cos(theta4)*cos(theta5)^2*sin(theta2)*sin(theta3)*sin(theta4) + 0.224*thetad1*cos(theta2)*cos(theta3)*cos(theta4)*cos(theta5)*sin(theta2)*sin(theta3)*sin(theta4)*sin(theta5) ;
C(3,2) = 0.3136*thetad2*cos(theta3) + 0.1568*thetad3*cos(theta3) + 0.87*thetad2*sin(theta3) + 0.435*thetad3*sin(theta3) - 0.4875*thetad1*cos(theta2)*cos(theta3) + 0.4018*thetad2*cos(theta3)*cos(theta4) + 0.2009*thetad3*cos(theta3)*cos(theta4) + 0.2009*thetad4*cos(theta3)*cos(theta4) - 0.150528*thetad1*cos(theta2)*sin(theta3) - 0.150528*thetad1*cos(theta3)*sin(theta2) + 0.1666*thetad2*cos(theta3)*sin(theta4) + 0.1666*thetad2*cos(theta4)*sin(theta3) + 0.0833*thetad3*cos(theta3)*sin(theta4) + 0.0833*thetad3*cos(theta4)*sin(theta3) + 0.0833*thetad4*cos(theta3)*sin(theta4) + 0.0833*thetad4*cos(theta4)*sin(theta3) + 0.4875*thetad1*sin(theta2)*sin(theta3) - 0.4018*thetad2*sin(theta3)*sin(theta4) - 0.2009*thetad3*sin(theta3)*sin(theta4) - 0.2009*thetad4*sin(theta3)*sin(theta4) - 0.190918*thetad1*cos(theta2)*cos(theta3)*cos(theta4) - 0.07*thetad1*cos(theta2)*cos(theta3)*cos(theta5) + 0.44*thetad4*cos(theta2)*cos(theta3)*cos(theta4) + 0.22*thetad5*cos(theta2)*cos(theta3)*cos(theta4) + 0.07*thetad5*cos(theta3)*cos(theta4)*cos(theta5) + 0.373674*thetad1*cos(theta2)*cos(theta3)*sin(theta4) + 0.373674*thetad1*cos(theta2)*cos(theta4)*sin(theta3) + 0.373674*thetad1*cos(theta3)*cos(theta4)*sin(theta2) - 0.014*thetad1*cos(theta2)*cos(theta3)*sin(theta5) + 0.028*thetad2*cos(theta3)*cos(theta5)*sin(theta4) + 0.028*thetad2*cos(theta4)*cos(theta5)*sin(theta3) + 0.014*thetad3*cos(theta3)*cos(theta5)*sin(theta4) + 0.014*thetad3*cos(theta4)*cos(theta5)*sin(theta3) + 0.014*thetad4*cos(theta3)*cos(theta5)*sin(theta4) + 0.014*thetad4*cos(theta4)*cos(theta5)*sin(theta3) + 0.014*thetad5*cos(theta3)*cos(theta4)*sin(theta5) + 0.190918*thetad1*cos(theta2)*sin(theta3)*sin(theta4) + 0.190918*thetad1*cos(theta3)*sin(theta2)*sin(theta4) + 0.190918*thetad1*cos(theta4)*sin(theta2)*sin(theta3) + 0.07*thetad1*cos(theta5)*sin(theta2)*sin(theta3) - 0.44*thetad4*cos(theta2)*sin(theta3)*sin(theta4) - 0.44*thetad4*cos(theta3)*sin(theta2)*sin(theta4) - 0.44*thetad4*cos(theta4)*sin(theta2)*sin(theta3) - 0.14*thetad2*cos(theta3)*sin(theta4)*sin(theta5) - 0.14*thetad2*cos(theta4)*sin(theta3)*sin(theta5) - 0.22*thetad5*cos(theta2)*sin(theta3)*sin(theta4) - 0.22*thetad5*cos(theta3)*sin(theta2)*sin(theta4) - 0.22*thetad5*cos(theta4)*sin(theta2)*sin(theta3) - 0.07*thetad3*cos(theta3)*sin(theta4)*sin(theta5) - 0.07*thetad3*cos(theta4)*sin(theta3)*sin(theta5) - 0.07*thetad4*cos(theta3)*sin(theta4)*sin(theta5) - 0.07*thetad4*cos(theta4)*sin(theta3)*sin(theta5) - 0.07*thetad5*cos(theta5)*sin(theta3)*sin(theta4) - 0.373674*thetad1*sin(theta2)*sin(theta3)*sin(theta4) + 0.014*thetad1*sin(theta2)*sin(theta3)*sin(theta5) - 0.014*thetad5*sin(theta3)*sin(theta4)*sin(theta5) - 0.7*thetad4*cos(theta1)*cos(theta2)*cos(theta3)*sin(theta4) - 0.7*thetad4*cos(theta1)*cos(theta2)*cos(theta4)*sin(theta3) - 0.7*thetad4*cos(theta1)*cos(theta3)*cos(theta4)*sin(theta2) + 0.049*thetad1*cos(theta2)*cos(theta3)*cos(theta5)*sin(theta4) + 0.049*thetad1*cos(theta2)*cos(theta4)*cos(theta5)*sin(theta3) + 0.049*thetad1*cos(theta3)*cos(theta4)*cos(theta5)*sin(theta2) - 0.35*thetad5*cos(theta1)*cos(theta2)*cos(theta3)*sin(theta4) - 0.35*thetad5*cos(theta1)*cos(theta2)*cos(theta4)*sin(theta3) - 0.35*thetad5*cos(theta1)*cos(theta3)*cos(theta4)*sin(theta2) + 0.1*thetad4*cos(theta2)*cos(theta3)*sin(theta1)*sin(theta4) + 0.1*thetad4*cos(theta2)*cos(theta4)*sin(theta1)*sin(theta3) + 0.1*thetad4*cos(theta3)*cos(theta4)*sin(theta1)*sin(theta2) + 0.0098*thetad1*cos(theta2)*cos(theta3)*sin(theta4)*sin(theta5) + 0.0098*thetad1*cos(theta2)*cos(theta4)*sin(theta3)*sin(theta5) + 0.0098*thetad1*cos(theta3)*cos(theta4)*sin(theta2)*sin(theta5) + 0.05*thetad5*cos(theta2)*cos(theta3)*sin(theta1)*sin(theta4) + 0.05*thetad5*cos(theta2)*cos(theta4)*sin(theta1)*sin(theta3) + 0.05*thetad5*cos(theta3)*cos(theta4)*sin(theta1)*sin(theta2) + 0.7*thetad4*cos(theta1)*sin(theta2)*sin(theta3)*sin(theta4) - 0.049*thetad1*cos(theta5)*sin(theta2)*sin(theta3)*sin(theta4) + 0.35*thetad5*cos(theta1)*sin(theta2)*sin(theta3)*sin(theta4) - 0.1*thetad4*sin(theta1)*sin(theta2)*sin(theta3)*sin(theta4) - 0.0098*thetad1*sin(theta2)*sin(theta3)*sin(theta4)*sin(theta5) - 0.05*thetad5*sin(theta1)*sin(theta2)*sin(theta3)*sin(theta4) - 0.88*thetad4*cos(theta1)^2*cos(theta2)*cos(theta3)*cos(theta4) - 0.028*thetad1*cos(theta2)*cos(theta3)*cos(theta4)*cos(theta5)^2 - 0.44*thetad5*cos(theta1)^2*cos(theta2)*cos(theta3)*cos(theta4) + 0.88*thetad4*cos(theta1)^2*cos(theta2)*sin(theta3)*sin(theta4) + 0.88*thetad4*cos(theta1)^2*cos(theta3)*sin(theta2)*sin(theta4) + 0.88*thetad4*cos(theta1)^2*cos(theta4)*sin(theta2)*sin(theta3) + 0.028*thetad1*cos(theta2)*cos(theta5)^2*sin(theta3)*sin(theta4) + 0.028*thetad1*cos(theta3)*cos(theta5)^2*sin(theta2)*sin(theta4) + 0.028*thetad1*cos(theta4)*cos(theta5)^2*sin(theta2)*sin(theta3) + 0.44*thetad5*cos(theta1)^2*cos(theta2)*sin(theta3)*sin(theta4) + 0.44*thetad5*cos(theta1)^2*cos(theta3)*sin(theta2)*sin(theta4) + 0.44*thetad5*cos(theta1)^2*cos(theta4)*sin(theta2)*sin(theta3) + 3.14*thetad4*cos(theta1)*cos(theta2)*cos(theta3)*cos(theta4)*sin(theta1) + 1.57*thetad5*cos(theta1)*cos(theta2)*cos(theta3)*cos(theta4)*sin(theta1) + 0.0672*thetad1*cos(theta2)*cos(theta3)*cos(theta4)*cos(theta5)*sin(theta5) - 3.14*thetad4*cos(theta1)*cos(theta2)*sin(theta1)*sin(theta3)*sin(theta4) - 3.14*thetad4*cos(theta1)*cos(theta3)*sin(theta1)*sin(theta2)*sin(theta4) - 3.14*thetad4*cos(theta1)*cos(theta4)*sin(theta1)*sin(theta2)*sin(theta3) - 1.57*thetad5*cos(theta1)*cos(theta2)*sin(theta1)*sin(theta3)*sin(theta4) - 1.57*thetad5*cos(theta1)*cos(theta3)*sin(theta1)*sin(theta2)*sin(theta4) - 1.57*thetad5*cos(theta1)*cos(theta4)*sin(theta1)*sin(theta2)*sin(theta3) - 0.0672*thetad1*cos(theta2)*cos(theta5)*sin(theta3)*sin(theta4)*sin(theta5) - 0.0672*thetad1*cos(theta3)*cos(theta5)*sin(theta2)*sin(theta4)*sin(theta5) - 0.0672*thetad1*cos(theta4)*cos(theta5)*sin(theta2)*sin(theta3)*sin(theta5) ;
C(3,3) = 0.1568*thetad2*cos(theta3) + 0.435*thetad2*sin(theta3) - 0.4875*thetad1*cos(theta2)*cos(theta3) + 0.2009*thetad2*cos(theta3)*cos(theta4) - 0.150528*thetad1*cos(theta2)*sin(theta3) - 0.150528*thetad1*cos(theta3)*sin(theta2) + 0.0833*thetad2*cos(theta3)*sin(theta4) + 0.0833*thetad2*cos(theta4)*sin(theta3) + 0.4875*thetad1*sin(theta2)*sin(theta3) - 0.2009*thetad2*sin(theta3)*sin(theta4) - 0.190918*thetad1*cos(theta2)*cos(theta3)*cos(theta4) - 0.07*thetad1*cos(theta2)*cos(theta3)*cos(theta5) + 0.44*thetad4*cos(theta2)*cos(theta3)*cos(theta4) + 0.22*thetad5*cos(theta2)*cos(theta3)*cos(theta4) + 0.373674*thetad1*cos(theta2)*cos(theta3)*sin(theta4) + 0.373674*thetad1*cos(theta2)*cos(theta4)*sin(theta3) + 0.373674*thetad1*cos(theta3)*cos(theta4)*sin(theta2) - 0.014*thetad1*cos(theta2)*cos(theta3)*sin(theta5) + 0.014*thetad2*cos(theta3)*cos(theta5)*sin(theta4) + 0.014*thetad2*cos(theta4)*cos(theta5)*sin(theta3) + 0.190918*thetad1*cos(theta2)*sin(theta3)*sin(theta4) + 0.190918*thetad1*cos(theta3)*sin(theta2)*sin(theta4) + 0.190918*thetad1*cos(theta4)*sin(theta2)*sin(theta3) + 0.07*thetad1*cos(theta5)*sin(theta2)*sin(theta3) - 0.44*thetad4*cos(theta2)*sin(theta3)*sin(theta4) - 0.44*thetad4*cos(theta3)*sin(theta2)*sin(theta4) - 0.44*thetad4*cos(theta4)*sin(theta2)*sin(theta3) - 0.07*thetad2*cos(theta3)*sin(theta4)*sin(theta5) - 0.07*thetad2*cos(theta4)*sin(theta3)*sin(theta5) - 0.22*thetad5*cos(theta2)*sin(theta3)*sin(theta4) - 0.22*thetad5*cos(theta3)*sin(theta2)*sin(theta4) - 0.22*thetad5*cos(theta4)*sin(theta2)*sin(theta3) - 0.373674*thetad1*sin(theta2)*sin(theta3)*sin(theta4) + 0.014*thetad1*sin(theta2)*sin(theta3)*sin(theta5) - 0.7*thetad4*cos(theta1)*cos(theta2)*cos(theta3)*sin(theta4) - 0.7*thetad4*cos(theta1)*cos(theta2)*cos(theta4)*sin(theta3) - 0.7*thetad4*cos(theta1)*cos(theta3)*cos(theta4)*sin(theta2) + 0.049*thetad1*cos(theta2)*cos(theta3)*cos(theta5)*sin(theta4) + 0.049*thetad1*cos(theta2)*cos(theta4)*cos(theta5)*sin(theta3) + 0.049*thetad1*cos(theta3)*cos(theta4)*cos(theta5)*sin(theta2) - 0.35*thetad5*cos(theta1)*cos(theta2)*cos(theta3)*sin(theta4) - 0.35*thetad5*cos(theta1)*cos(theta2)*cos(theta4)*sin(theta3) - 0.35*thetad5*cos(theta1)*cos(theta3)*cos(theta4)*sin(theta2) + 0.1*thetad4*cos(theta2)*cos(theta3)*sin(theta1)*sin(theta4) + 0.1*thetad4*cos(theta2)*cos(theta4)*sin(theta1)*sin(theta3) + 0.1*thetad4*cos(theta3)*cos(theta4)*sin(theta1)*sin(theta2) + 0.0098*thetad1*cos(theta2)*cos(theta3)*sin(theta4)*sin(theta5) + 0.0098*thetad1*cos(theta2)*cos(theta4)*sin(theta3)*sin(theta5) + 0.0098*thetad1*cos(theta3)*cos(theta4)*sin(theta2)*sin(theta5) + 0.05*thetad5*cos(theta2)*cos(theta3)*sin(theta1)*sin(theta4) + 0.05*thetad5*cos(theta2)*cos(theta4)*sin(theta1)*sin(theta3) + 0.05*thetad5*cos(theta3)*cos(theta4)*sin(theta1)*sin(theta2) + 0.7*thetad4*cos(theta1)*sin(theta2)*sin(theta3)*sin(theta4) - 0.049*thetad1*cos(theta5)*sin(theta2)*sin(theta3)*sin(theta4) + 0.35*thetad5*cos(theta1)*sin(theta2)*sin(theta3)*sin(theta4) - 0.1*thetad4*sin(theta1)*sin(theta2)*sin(theta3)*sin(theta4) - 0.0098*thetad1*sin(theta2)*sin(theta3)*sin(theta4)*sin(theta5) - 0.05*thetad5*sin(theta1)*sin(theta2)*sin(theta3)*sin(theta4) - 0.88*thetad4*cos(theta1)^2*cos(theta2)*cos(theta3)*cos(theta4) - 0.028*thetad1*cos(theta2)*cos(theta3)*cos(theta4)*cos(theta5)^2 - 0.44*thetad5*cos(theta1)^2*cos(theta2)*cos(theta3)*cos(theta4) + 0.88*thetad4*cos(theta1)^2*cos(theta2)*sin(theta3)*sin(theta4) + 0.88*thetad4*cos(theta1)^2*cos(theta3)*sin(theta2)*sin(theta4) + 0.88*thetad4*cos(theta1)^2*cos(theta4)*sin(theta2)*sin(theta3) + 0.028*thetad1*cos(theta2)*cos(theta5)^2*sin(theta3)*sin(theta4) + 0.028*thetad1*cos(theta3)*cos(theta5)^2*sin(theta2)*sin(theta4) + 0.028*thetad1*cos(theta4)*cos(theta5)^2*sin(theta2)*sin(theta3) + 0.44*thetad5*cos(theta1)^2*cos(theta2)*sin(theta3)*sin(theta4) + 0.44*thetad5*cos(theta1)^2*cos(theta3)*sin(theta2)*sin(theta4) + 0.44*thetad5*cos(theta1)^2*cos(theta4)*sin(theta2)*sin(theta3) + 3.14*thetad4*cos(theta1)*cos(theta2)*cos(theta3)*cos(theta4)*sin(theta1) + 1.57*thetad5*cos(theta1)*cos(theta2)*cos(theta3)*cos(theta4)*sin(theta1) + 0.0672*thetad1*cos(theta2)*cos(theta3)*cos(theta4)*cos(theta5)*sin(theta5) - 3.14*thetad4*cos(theta1)*cos(theta2)*sin(theta1)*sin(theta3)*sin(theta4) - 3.14*thetad4*cos(theta1)*cos(theta3)*sin(theta1)*sin(theta2)*sin(theta4) - 3.14*thetad4*cos(theta1)*cos(theta4)*sin(theta1)*sin(theta2)*sin(theta3) - 1.57*thetad5*cos(theta1)*cos(theta2)*sin(theta1)*sin(theta3)*sin(theta4) - 1.57*thetad5*cos(theta1)*cos(theta3)*sin(theta1)*sin(theta2)*sin(theta4) - 1.57*thetad5*cos(theta1)*cos(theta4)*sin(theta1)*sin(theta2)*sin(theta3) - 0.0672*thetad1*cos(theta2)*cos(theta5)*sin(theta3)*sin(theta4)*sin(theta5) - 0.0672*thetad1*cos(theta3)*cos(theta5)*sin(theta2)*sin(theta4)*sin(theta5) - 0.0672*thetad1*cos(theta4)*cos(theta5)*sin(theta2)*sin(theta3)*sin(theta5) ;
C(3,4) = 0.2009*thetad2*cos(theta3)*cos(theta4) - 0.1*thetad5*cos(theta1) - 1.4*thetad4*sin(theta1) - 0.7*thetad5*sin(theta1) - 0.2*thetad4*cos(theta1) + 5.64*thetad4*cos(theta2)*sin(theta2) + 0.0833*thetad2*cos(theta3)*sin(theta4) + 0.0833*thetad2*cos(theta4)*sin(theta3) + 2.82*thetad5*cos(theta2)*sin(theta2) + 5.64*thetad4*cos(theta3)*sin(theta3) + 2.82*thetad5*cos(theta3)*sin(theta3) + 5.64*thetad4*cos(theta4)*sin(theta4) + 2.82*thetad5*cos(theta4)*sin(theta4) - 0.2009*thetad2*sin(theta3)*sin(theta4) + 0.4*thetad4*cos(theta1)*cos(theta2)^2 + 0.4*thetad4*cos(theta1)*cos(theta3)^2 + 0.2*thetad5*cos(theta1)*cos(theta2)^2 + 0.4*thetad4*cos(theta1)*cos(theta4)^2 + 0.2*thetad5*cos(theta1)*cos(theta3)^2 + 0.2*thetad5*cos(theta1)*cos(theta4)^2 + 2.8*thetad4*cos(theta2)^2*sin(theta1) + 2.8*thetad4*cos(theta3)^2*sin(theta1) + 1.4*thetad5*cos(theta2)^2*sin(theta1) + 2.8*thetad4*cos(theta4)^2*sin(theta1) + 1.4*thetad5*cos(theta3)^2*sin(theta1) + 1.4*thetad5*cos(theta4)^2*sin(theta1) - 0.8*thetad4*cos(theta1)*cos(theta2)^2*cos(theta3)^2 - 0.8*thetad4*cos(theta1)*cos(theta2)^2*cos(theta4)^2 - 0.4*thetad5*cos(theta1)*cos(theta2)^2*cos(theta3)^2 - 0.8*thetad4*cos(theta1)*cos(theta3)^2*cos(theta4)^2 - 0.4*thetad5*cos(theta1)*cos(theta2)^2*cos(theta4)^2 - 0.4*thetad5*cos(theta1)*cos(theta3)^2*cos(theta4)^2 - 5.6*thetad4*cos(theta2)^2*cos(theta3)^2*sin(theta1) - 5.6*thetad4*cos(theta2)^2*cos(theta4)^2*sin(theta1) - 2.8*thetad5*cos(theta2)^2*cos(theta3)^2*sin(theta1) - 5.6*thetad4*cos(theta3)^2*cos(theta4)^2*sin(theta1) - 2.8*thetad5*cos(theta2)^2*cos(theta4)^2*sin(theta1) - 2.8*thetad5*cos(theta3)^2*cos(theta4)^2*sin(theta1) + 0.249082*thetad1*cos(theta2)*cos(theta3)*cos(theta4) + 0.44*thetad2*cos(theta2)*cos(theta3)*cos(theta4) + 0.44*thetad3*cos(theta2)*cos(theta3)*cos(theta4) + 0.373674*thetad1*cos(theta2)*cos(theta3)*sin(theta4) + 0.373674*thetad1*cos(theta2)*cos(theta4)*sin(theta3) + 0.373674*thetad1*cos(theta3)*cos(theta4)*sin(theta2) + 0.014*thetad2*cos(theta3)*cos(theta5)*sin(theta4) + 0.014*thetad2*cos(theta4)*cos(theta5)*sin(theta3) - 0.249082*thetad1*cos(theta2)*sin(theta3)*sin(theta4) - 0.249082*thetad1*cos(theta3)*sin(theta2)*sin(theta4) - 0.249082*thetad1*cos(theta4)*sin(theta2)*sin(theta3) - 0.44*thetad2*cos(theta2)*sin(theta3)*sin(theta4) - 0.44*thetad2*cos(theta3)*sin(theta2)*sin(theta4) - 0.44*thetad2*cos(theta4)*sin(theta2)*sin(theta3) - 0.44*thetad3*cos(theta2)*sin(theta3)*sin(theta4) - 0.44*thetad3*cos(theta3)*sin(theta2)*sin(theta4) - 0.44*thetad3*cos(theta4)*sin(theta2)*sin(theta3) - 0.07*thetad2*cos(theta3)*sin(theta4)*sin(theta5) - 0.07*thetad2*cos(theta4)*sin(theta3)*sin(theta5) - 0.373674*thetad1*sin(theta2)*sin(theta3)*sin(theta4) - 6.28*thetad4*cos(theta1)^2*cos(theta2)*sin(theta2) - 3.14*thetad5*cos(theta1)^2*cos(theta2)*sin(theta2) - 11.28*thetad4*cos(theta2)*cos(theta3)^2*sin(theta2) - 6.28*thetad4*cos(theta1)^2*cos(theta3)*sin(theta3) - 11.28*thetad4*cos(theta2)*cos(theta4)^2*sin(theta2) - 11.28*thetad4*cos(theta2)^2*cos(theta3)*sin(theta3) - 5.64*thetad5*cos(theta2)*cos(theta3)^2*sin(theta2) - 3.14*thetad5*cos(theta1)^2*cos(theta3)*sin(theta3) - 6.28*thetad4*cos(theta1)^2*cos(theta4)*sin(theta4) - 5.64*thetad5*cos(theta2)*cos(theta4)^2*sin(theta2) - 5.64*thetad5*cos(theta2)^2*cos(theta3)*sin(theta3) - 11.28*thetad4*cos(theta3)*cos(theta4)^2*sin(theta3) - 11.28*thetad4*cos(theta2)^2*cos(theta4)*sin(theta4) - 3.14*thetad5*cos(theta1)^2*cos(theta4)*sin(theta4) - 11.28*thetad4*cos(theta3)^2*cos(theta4)*sin(theta4) - 5.64*thetad5*cos(theta3)*cos(theta4)^2*sin(theta3) - 5.64*thetad5*cos(theta2)^2*cos(theta4)*sin(theta4) - 5.64*thetad5*cos(theta3)^2*cos(theta4)*sin(theta4) + 12.56*thetad4*cos(theta1)^2*cos(theta2)*cos(theta3)^2*sin(theta2) + 12.56*thetad4*cos(theta1)^2*cos(theta2)*cos(theta4)^2*sin(theta2) + 12.56*thetad4*cos(theta1)^2*cos(theta2)^2*cos(theta3)*sin(theta3) + 6.28*thetad5*cos(theta1)^2*cos(theta2)*cos(theta3)^2*sin(theta2) + 6.28*thetad5*cos(theta1)^2*cos(theta2)*cos(theta4)^2*sin(theta2) + 6.28*thetad5*cos(theta1)^2*cos(theta2)^2*cos(theta3)*sin(theta3) + 22.56*thetad4*cos(theta2)*cos(theta3)^2*cos(theta4)^2*sin(theta2) + 12.56*thetad4*cos(theta1)^2*cos(theta3)*cos(theta4)^2*sin(theta3) + 12.56*thetad4*cos(theta1)^2*cos(theta2)^2*cos(theta4)*sin(theta4) + 12.56*thetad4*cos(theta1)^2*cos(theta3)^2*cos(theta4)*sin(theta4) + 22.56*thetad4*cos(theta2)^2*cos(theta3)*cos(theta4)^2*sin(theta3) + 11.28*thetad5*cos(theta2)*cos(theta3)^2*cos(theta4)^2*sin(theta2) + 6.28*thetad5*cos(theta1)^2*cos(theta3)*cos(theta4)^2*sin(theta3) + 6.28*thetad5*cos(theta1)^2*cos(theta2)^2*cos(theta4)*sin(theta4) + 22.56*thetad4*cos(theta2)^2*cos(theta3)^2*cos(theta4)*sin(theta4) + 6.28*thetad5*cos(theta1)^2*cos(theta3)^2*cos(theta4)*sin(theta4) + 11.28*thetad5*cos(theta2)^2*cos(theta3)*cos(theta4)^2*sin(theta3) + 11.28*thetad5*cos(theta2)^2*cos(theta3)^2*cos(theta4)*sin(theta4) - 0.7*thetad1*cos(theta1)*cos(theta2)*cos(theta3)*sin(theta4) - 0.7*thetad1*cos(theta1)*cos(theta2)*cos(theta4)*sin(theta3) - 0.7*thetad1*cos(theta1)*cos(theta3)*cos(theta4)*sin(theta2) - 0.7*thetad2*cos(theta1)*cos(theta2)*cos(theta3)*sin(theta4) - 0.7*thetad2*cos(theta1)*cos(theta2)*cos(theta4)*sin(theta3) - 0.7*thetad2*cos(theta1)*cos(theta3)*cos(theta4)*sin(theta2) - 0.7*thetad3*cos(theta1)*cos(theta2)*cos(theta3)*sin(theta4) - 0.7*thetad3*cos(theta1)*cos(theta2)*cos(theta4)*sin(theta3) - 0.7*thetad3*cos(theta1)*cos(theta3)*cos(theta4)*sin(theta2) + 0.049*thetad1*cos(theta2)*cos(theta3)*cos(theta5)*sin(theta4) + 0.049*thetad1*cos(theta2)*cos(theta4)*cos(theta5)*sin(theta3) + 0.049*thetad1*cos(theta3)*cos(theta4)*cos(theta5)*sin(theta2) + 1.6*thetad4*cos(theta1)*cos(theta2)^2*cos(theta3)^2*cos(theta4)^2 + 0.8*thetad5*cos(theta1)*cos(theta2)^2*cos(theta3)^2*cos(theta4)^2 - 1.76*thetad4*cos(theta1)*cos(theta2)*sin(theta1)*sin(theta2) + 0.1*thetad1*cos(theta2)*cos(theta3)*sin(theta1)*sin(theta4) + 0.1*thetad1*cos(theta2)*cos(theta4)*sin(theta1)*sin(theta3) + 0.1*thetad1*cos(theta3)*cos(theta4)*sin(theta1)*sin(theta2) - 0.88*thetad5*cos(theta1)*cos(theta2)*sin(theta1)*sin(theta2) + 0.1*thetad2*cos(theta2)*cos(theta3)*sin(theta1)*sin(theta4) + 0.1*thetad2*cos(theta2)*cos(theta4)*sin(theta1)*sin(theta3) + 0.1*thetad2*cos(theta3)*cos(theta4)*sin(theta1)*sin(theta2) - 1.76*thetad4*cos(theta1)*cos(theta3)*sin(theta1)*sin(theta3) + 0.1*thetad3*cos(theta2)*cos(theta3)*sin(theta1)*sin(theta4) + 0.1*thetad3*cos(theta2)*cos(theta4)*sin(theta1)*sin(theta3) + 0.1*thetad3*cos(theta3)*cos(theta4)*sin(theta1)*sin(theta2) - 0.88*thetad5*cos(theta1)*cos(theta3)*sin(theta1)*sin(theta3) - 1.76*thetad4*cos(theta1)*cos(theta4)*sin(theta1)*sin(theta4) + 0.0098*thetad1*cos(theta2)*cos(theta3)*sin(theta4)*sin(theta5) + 0.0098*thetad1*cos(theta2)*cos(theta4)*sin(theta3)*sin(theta5) + 0.0098*thetad1*cos(theta3)*cos(theta4)*sin(theta2)*sin(theta5) - 0.88*thetad5*cos(theta1)*cos(theta4)*sin(theta1)*sin(theta4) + 11.2*thetad4*cos(theta2)^2*cos(theta3)^2*cos(theta4)^2*sin(theta1) + 5.6*thetad5*cos(theta2)^2*cos(theta3)^2*cos(theta4)^2*sin(theta1) + 0.7*thetad1*cos(theta1)*sin(theta2)*sin(theta3)*sin(theta4) + 0.7*thetad2*cos(theta1)*sin(theta2)*sin(theta3)*sin(theta4) + 0.7*thetad3*cos(theta1)*sin(theta2)*sin(theta3)*sin(theta4) - 0.049*thetad1*cos(theta5)*sin(theta2)*sin(theta3)*sin(theta4) - 0.1*thetad1*sin(theta1)*sin(theta2)*sin(theta3)*sin(theta4) - 0.1*thetad2*sin(theta1)*sin(theta2)*sin(theta3)*sin(theta4) - 0.1*thetad3*sin(theta1)*sin(theta2)*sin(theta3)*sin(theta4) - 0.0098*thetad1*sin(theta2)*sin(theta3)*sin(theta4)*sin(theta5) - 0.88*thetad1*cos(theta1)^2*cos(theta2)*cos(theta3)*cos(theta4) - 0.88*thetad2*cos(theta1)^2*cos(theta2)*cos(theta3)*cos(theta4) - 0.88*thetad3*cos(theta1)^2*cos(theta2)*cos(theta3)*cos(theta4) - 0.028*thetad1*cos(theta2)*cos(theta3)*cos(theta4)*cos(theta5)^2 + 0.88*thetad1*cos(theta1)^2*cos(theta2)*sin(theta3)*sin(theta4) + 0.88*thetad1*cos(theta1)^2*cos(theta3)*sin(theta2)*sin(theta4) + 0.88*thetad1*cos(theta1)^2*cos(theta4)*sin(theta2)*sin(theta3) + 0.88*thetad2*cos(theta1)^2*cos(theta2)*sin(theta3)*sin(theta4) + 0.88*thetad2*cos(theta1)^2*cos(theta3)*sin(theta2)*sin(theta4) + 0.88*thetad2*cos(theta1)^2*cos(theta4)*sin(theta2)*sin(theta3) + 0.88*thetad3*cos(theta1)^2*cos(theta2)*sin(theta3)*sin(theta4) + 0.88*thetad3*cos(theta1)^2*cos(theta3)*sin(theta2)*sin(theta4) + 0.88*thetad3*cos(theta1)^2*cos(theta4)*sin(theta2)*sin(theta3) + 0.028*thetad1*cos(theta2)*cos(theta5)^2*sin(theta3)*sin(theta4) + 0.028*thetad1*cos(theta3)*cos(theta5)^2*sin(theta2)*sin(theta4) + 0.028*thetad1*cos(theta4)*cos(theta5)^2*sin(theta2)*sin(theta3) + 3.14*thetad1*cos(theta1)*cos(theta2)*cos(theta3)*cos(theta4)*sin(theta1) + 3.14*thetad2*cos(theta1)*cos(theta2)*cos(theta3)*cos(theta4)*sin(theta1) + 3.14*thetad3*cos(theta1)*cos(theta2)*cos(theta3)*cos(theta4)*sin(theta1) + 0.0672*thetad1*cos(theta2)*cos(theta3)*cos(theta4)*cos(theta5)*sin(theta5) + 0.8*thetad4*cos(theta1)*cos(theta2)*cos(theta3)*sin(theta2)*sin(theta3) + 0.4*thetad5*cos(theta1)*cos(theta2)*cos(theta3)*sin(theta2)*sin(theta3) + 0.8*thetad4*cos(theta1)*cos(theta2)*cos(theta4)*sin(theta2)*sin(theta4) + 0.4*thetad5*cos(theta1)*cos(theta2)*cos(theta4)*sin(theta2)*sin(theta4) + 0.8*thetad4*cos(theta1)*cos(theta3)*cos(theta4)*sin(theta3)*sin(theta4) + 0.4*thetad5*cos(theta1)*cos(theta3)*cos(theta4)*sin(theta3)*sin(theta4) - 25.12*thetad4*cos(theta1)^2*cos(theta2)*cos(theta3)^2*cos(theta4)^2*sin(theta2) - 25.12*thetad4*cos(theta1)^2*cos(theta2)^2*cos(theta3)*cos(theta4)^2*sin(theta3) - 12.56*thetad5*cos(theta1)^2*cos(theta2)*cos(theta3)^2*cos(theta4)^2*sin(theta2) - 25.12*thetad4*cos(theta1)^2*cos(theta2)^2*cos(theta3)^2*cos(theta4)*sin(theta4) - 12.56*thetad5*cos(theta1)^2*cos(theta2)^2*cos(theta3)*cos(theta4)^2*sin(theta3) - 12.56*thetad5*cos(theta1)^2*cos(theta2)^2*cos(theta3)^2*cos(theta4)*sin(theta4) - 3.14*thetad1*cos(theta1)*cos(theta2)*sin(theta1)*sin(theta3)*sin(theta4) - 3.14*thetad1*cos(theta1)*cos(theta3)*sin(theta1)*sin(theta2)*sin(theta4) - 3.14*thetad1*cos(theta1)*cos(theta4)*sin(theta1)*sin(theta2)*sin(theta3) - 3.14*thetad2*cos(theta1)*cos(theta2)*sin(theta1)*sin(theta3)*sin(theta4) - 3.14*thetad2*cos(theta1)*cos(theta3)*sin(theta1)*sin(theta2)*sin(theta4) - 3.14*thetad2*cos(theta1)*cos(theta4)*sin(theta1)*sin(theta2)*sin(theta3) - 3.14*thetad3*cos(theta1)*cos(theta2)*sin(theta1)*sin(theta3)*sin(theta4) - 3.14*thetad3*cos(theta1)*cos(theta3)*sin(theta1)*sin(theta2)*sin(theta4) - 3.14*thetad3*cos(theta1)*cos(theta4)*sin(theta1)*sin(theta2)*sin(theta3) + 5.6*thetad4*cos(theta2)*cos(theta3)*sin(theta1)*sin(theta2)*sin(theta3) + 2.8*thetad5*cos(theta2)*cos(theta3)*sin(theta1)*sin(theta2)*sin(theta3) + 5.6*thetad4*cos(theta2)*cos(theta4)*sin(theta1)*sin(theta2)*sin(theta4) + 2.8*thetad5*cos(theta2)*cos(theta4)*sin(theta1)*sin(theta2)*sin(theta4) + 5.6*thetad4*cos(theta3)*cos(theta4)*sin(theta1)*sin(theta3)*sin(theta4) - 0.0672*thetad1*cos(theta2)*cos(theta5)*sin(theta3)*sin(theta4)*sin(theta5) - 0.0672*thetad1*cos(theta3)*cos(theta5)*sin(theta2)*sin(theta4)*sin(theta5) - 0.0672*thetad1*cos(theta4)*cos(theta5)*sin(theta2)*sin(theta3)*sin(theta5) + 2.8*thetad5*cos(theta3)*cos(theta4)*sin(theta1)*sin(theta3)*sin(theta4) + 3.52*thetad4*cos(theta1)*cos(theta2)*cos(theta3)^2*sin(theta1)*sin(theta2) + 3.52*thetad4*cos(theta1)*cos(theta2)*cos(theta4)^2*sin(theta1)*sin(theta2) + 3.52*thetad4*cos(theta1)*cos(theta2)^2*cos(theta3)*sin(theta1)*sin(theta3) + 1.76*thetad5*cos(theta1)*cos(theta2)*cos(theta3)^2*sin(theta1)*sin(theta2) + 1.76*thetad5*cos(theta1)*cos(theta2)*cos(theta4)^2*sin(theta1)*sin(theta2) + 1.76*thetad5*cos(theta1)*cos(theta2)^2*cos(theta3)*sin(theta1)*sin(theta3) + 3.52*thetad4*cos(theta1)*cos(theta3)*cos(theta4)^2*sin(theta1)*sin(theta3) + 3.52*thetad4*cos(theta1)*cos(theta2)^2*cos(theta4)*sin(theta1)*sin(theta4) + 3.52*thetad4*cos(theta1)*cos(theta3)^2*cos(theta4)*sin(theta1)*sin(theta4) + 1.76*thetad5*cos(theta1)*cos(theta3)*cos(theta4)^2*sin(theta1)*sin(theta3) + 1.76*thetad5*cos(theta1)*cos(theta2)^2*cos(theta4)*sin(theta1)*sin(theta4) + 1.76*thetad5*cos(theta1)*cos(theta3)^2*cos(theta4)*sin(theta1)*sin(theta4) - 22.56*thetad4*cos(theta2)*cos(theta3)*cos(theta4)*sin(theta2)*sin(theta3)*sin(theta4) - 11.28*thetad5*cos(theta2)*cos(theta3)*cos(theta4)*sin(theta2)*sin(theta3)*sin(theta4) - 1.6*thetad4*cos(theta1)*cos(theta2)*cos(theta3)*cos(theta4)^2*sin(theta2)*sin(theta3) - 1.6*thetad4*cos(theta1)*cos(theta2)*cos(theta3)^2*cos(theta4)*sin(theta2)*sin(theta4) - 0.8*thetad5*cos(theta1)*cos(theta2)*cos(theta3)*cos(theta4)^2*sin(theta2)*sin(theta3) - 1.6*thetad4*cos(theta1)*cos(theta2)^2*cos(theta3)*cos(theta4)*sin(theta3)*sin(theta4) - 0.8*thetad5*cos(theta1)*cos(theta2)*cos(theta3)^2*cos(theta4)*sin(theta2)*sin(theta4) - 0.8*thetad5*cos(theta1)*cos(theta2)^2*cos(theta3)*cos(theta4)*sin(theta3)*sin(theta4) - 11.2*thetad4*cos(theta2)*cos(theta3)*cos(theta4)^2*sin(theta1)*sin(theta2)*sin(theta3) - 11.2*thetad4*cos(theta2)*cos(theta3)^2*cos(theta4)*sin(theta1)*sin(theta2)*sin(theta4) - 5.6*thetad5*cos(theta2)*cos(theta3)*cos(theta4)^2*sin(theta1)*sin(theta2)*sin(theta3) - 11.2*thetad4*cos(theta2)^2*cos(theta3)*cos(theta4)*sin(theta1)*sin(theta3)*sin(theta4) - 5.6*thetad5*cos(theta2)*cos(theta3)^2*cos(theta4)*sin(theta1)*sin(theta2)*sin(theta4) - 5.6*thetad5*cos(theta2)^2*cos(theta3)*cos(theta4)*sin(theta1)*sin(theta3)*sin(theta4) - 7.04*thetad4*cos(theta1)*cos(theta2)*cos(theta3)^2*cos(theta4)^2*sin(theta1)*sin(theta2) - 7.04*thetad4*cos(theta1)*cos(theta2)^2*cos(theta3)*cos(theta4)^2*sin(theta1)*sin(theta3) - 3.52*thetad5*cos(theta1)*cos(theta2)*cos(theta3)^2*cos(theta4)^2*sin(theta1)*sin(theta2) - 7.04*thetad4*cos(theta1)*cos(theta2)^2*cos(theta3)^2*cos(theta4)*sin(theta1)*sin(theta4) - 3.52*thetad5*cos(theta1)*cos(theta2)^2*cos(theta3)*cos(theta4)^2*sin(theta1)*sin(theta3) - 3.52*thetad5*cos(theta1)*cos(theta2)^2*cos(theta3)^2*cos(theta4)*sin(theta1)*sin(theta4) + 25.12*thetad4*cos(theta1)^2*cos(theta2)*cos(theta3)*cos(theta4)*sin(theta2)*sin(theta3)*sin(theta4) + 12.56*thetad5*cos(theta1)^2*cos(theta2)*cos(theta3)*cos(theta4)*sin(theta2)*sin(theta3)*sin(theta4) + 7.04*thetad4*cos(theta1)*cos(theta2)*cos(theta3)*cos(theta4)*sin(theta1)*sin(theta2)*sin(theta3)*sin(theta4) + 3.52*thetad5*cos(theta1)*cos(theta2)*cos(theta3)*cos(theta4)*sin(theta1)*sin(theta2)*sin(theta3)*sin(theta4) ;
C(3,5) = 2.82*thetad4*cos(theta2)*sin(theta2) - 0.1*thetad5*cos(theta1) - 0.7*thetad4*sin(theta1) - 0.7*thetad5*sin(theta1) - 0.1*thetad4*cos(theta1) + 2.82*thetad5*cos(theta2)*sin(theta2) + 2.82*thetad4*cos(theta3)*sin(theta3) + 2.82*thetad5*cos(theta3)*sin(theta3) + 2.82*thetad4*cos(theta4)*sin(theta4) + 2.82*thetad5*cos(theta4)*sin(theta4) + 0.2*thetad4*cos(theta1)*cos(theta2)^2 + 0.2*thetad4*cos(theta1)*cos(theta3)^2 + 0.2*thetad5*cos(theta1)*cos(theta2)^2 + 0.2*thetad4*cos(theta1)*cos(theta4)^2 + 0.2*thetad5*cos(theta1)*cos(theta3)^2 + 0.2*thetad5*cos(theta1)*cos(theta4)^2 + 1.4*thetad4*cos(theta2)^2*sin(theta1) + 1.4*thetad4*cos(theta3)^2*sin(theta1) + 1.4*thetad5*cos(theta2)^2*sin(theta1) + 1.4*thetad4*cos(theta4)^2*sin(theta1) + 1.4*thetad5*cos(theta3)^2*sin(theta1) + 1.4*thetad5*cos(theta4)^2*sin(theta1) - 0.4*thetad4*cos(theta1)*cos(theta2)^2*cos(theta3)^2 - 0.4*thetad4*cos(theta1)*cos(theta2)^2*cos(theta4)^2 - 0.4*thetad5*cos(theta1)*cos(theta2)^2*cos(theta3)^2 - 0.4*thetad4*cos(theta1)*cos(theta3)^2*cos(theta4)^2 - 0.4*thetad5*cos(theta1)*cos(theta2)^2*cos(theta4)^2 - 0.4*thetad5*cos(theta1)*cos(theta3)^2*cos(theta4)^2 - 2.8*thetad4*cos(theta2)^2*cos(theta3)^2*sin(theta1) - 2.8*thetad4*cos(theta2)^2*cos(theta4)^2*sin(theta1) - 2.8*thetad5*cos(theta2)^2*cos(theta3)^2*sin(theta1) - 2.8*thetad4*cos(theta3)^2*cos(theta4)^2*sin(theta1) - 2.8*thetad5*cos(theta2)^2*cos(theta4)^2*sin(theta1) - 2.8*thetad5*cos(theta3)^2*cos(theta4)^2*sin(theta1) + 0.22*thetad1*cos(theta2)*cos(theta3)*cos(theta4) + 0.22*thetad2*cos(theta2)*cos(theta3)*cos(theta4) + 0.22*thetad3*cos(theta2)*cos(theta3)*cos(theta4) + 0.07*thetad2*cos(theta3)*cos(theta4)*cos(theta5) + 0.0728*thetad1*cos(theta2)*cos(theta3)*sin(theta4) + 0.0728*thetad1*cos(theta2)*cos(theta4)*sin(theta3) + 0.0728*thetad1*cos(theta3)*cos(theta4)*sin(theta2) + 0.014*thetad1*cos(theta2)*cos(theta5)*sin(theta3) + 0.014*thetad1*cos(theta3)*cos(theta5)*sin(theta2) + 0.014*thetad2*cos(theta3)*cos(theta4)*sin(theta5) - 0.22*thetad1*cos(theta2)*sin(theta3)*sin(theta4) - 0.22*thetad1*cos(theta3)*sin(theta2)*sin(theta4) - 0.22*thetad1*cos(theta4)*sin(theta2)*sin(theta3) - 0.07*thetad1*cos(theta2)*sin(theta3)*sin(theta5) - 0.07*thetad1*cos(theta3)*sin(theta2)*sin(theta5) - 0.22*thetad2*cos(theta2)*sin(theta3)*sin(theta4) - 0.22*thetad2*cos(theta3)*sin(theta2)*sin(theta4) - 0.22*thetad2*cos(theta4)*sin(theta2)*sin(theta3) - 0.22*thetad3*cos(theta2)*sin(theta3)*sin(theta4) - 0.22*thetad3*cos(theta3)*sin(theta2)*sin(theta4) - 0.22*thetad3*cos(theta4)*sin(theta2)*sin(theta3) - 0.07*thetad2*cos(theta5)*sin(theta3)*sin(theta4) - 0.0728*thetad1*sin(theta2)*sin(theta3)*sin(theta4) - 0.014*thetad2*sin(theta3)*sin(theta4)*sin(theta5) - 3.14*thetad4*cos(theta1)^2*cos(theta2)*sin(theta2) - 3.14*thetad5*cos(theta1)^2*cos(theta2)*sin(theta2) - 5.64*thetad4*cos(theta2)*cos(theta3)^2*sin(theta2) - 3.14*thetad4*cos(theta1)^2*cos(theta3)*sin(theta3) - 5.64*thetad4*cos(theta2)*cos(theta4)^2*sin(theta2) - 5.64*thetad4*cos(theta2)^2*cos(theta3)*sin(theta3) - 5.64*thetad5*cos(theta2)*cos(theta3)^2*sin(theta2) - 3.14*thetad5*cos(theta1)^2*cos(theta3)*sin(theta3) - 3.14*thetad4*cos(theta1)^2*cos(theta4)*sin(theta4) - 5.64*thetad5*cos(theta2)*cos(theta4)^2*sin(theta2) - 5.64*thetad5*cos(theta2)^2*cos(theta3)*sin(theta3) - 5.64*thetad4*cos(theta3)*cos(theta4)^2*sin(theta3) - 5.64*thetad4*cos(theta2)^2*cos(theta4)*sin(theta4) - 3.14*thetad5*cos(theta1)^2*cos(theta4)*sin(theta4) - 5.64*thetad4*cos(theta3)^2*cos(theta4)*sin(theta4) - 5.64*thetad5*cos(theta3)*cos(theta4)^2*sin(theta3) - 5.64*thetad5*cos(theta2)^2*cos(theta4)*sin(theta4) - 5.64*thetad5*cos(theta3)^2*cos(theta4)*sin(theta4) + 6.28*thetad4*cos(theta1)^2*cos(theta2)*cos(theta3)^2*sin(theta2) + 6.28*thetad4*cos(theta1)^2*cos(theta2)*cos(theta4)^2*sin(theta2) + 6.28*thetad4*cos(theta1)^2*cos(theta2)^2*cos(theta3)*sin(theta3) + 6.28*thetad5*cos(theta1)^2*cos(theta2)*cos(theta3)^2*sin(theta2) + 6.28*thetad5*cos(theta1)^2*cos(theta2)*cos(theta4)^2*sin(theta2) + 6.28*thetad5*cos(theta1)^2*cos(theta2)^2*cos(theta3)*sin(theta3) + 11.28*thetad4*cos(theta2)*cos(theta3)^2*cos(theta4)^2*sin(theta2) + 6.28*thetad4*cos(theta1)^2*cos(theta3)*cos(theta4)^2*sin(theta3) + 6.28*thetad4*cos(theta1)^2*cos(theta2)^2*cos(theta4)*sin(theta4) + 6.28*thetad4*cos(theta1)^2*cos(theta3)^2*cos(theta4)*sin(theta4) + 11.28*thetad4*cos(theta2)^2*cos(theta3)*cos(theta4)^2*sin(theta3) + 11.28*thetad5*cos(theta2)*cos(theta3)^2*cos(theta4)^2*sin(theta2) + 6.28*thetad5*cos(theta1)^2*cos(theta3)*cos(theta4)^2*sin(theta3) + 6.28*thetad5*cos(theta1)^2*cos(theta2)^2*cos(theta4)*sin(theta4) + 11.28*thetad4*cos(theta2)^2*cos(theta3)^2*cos(theta4)*sin(theta4) + 6.28*thetad5*cos(theta1)^2*cos(theta3)^2*cos(theta4)*sin(theta4) + 11.28*thetad5*cos(theta2)^2*cos(theta3)*cos(theta4)^2*sin(theta3) + 11.28*thetad5*cos(theta2)^2*cos(theta3)^2*cos(theta4)*sin(theta4) + 0.0098*thetad1*cos(theta2)*cos(theta3)*cos(theta4)*cos(theta5) - 0.35*thetad1*cos(theta1)*cos(theta2)*cos(theta3)*sin(theta4) - 0.35*thetad1*cos(theta1)*cos(theta2)*cos(theta4)*sin(theta3) - 0.35*thetad1*cos(theta1)*cos(theta3)*cos(theta4)*sin(theta2) - 0.35*thetad2*cos(theta1)*cos(theta2)*cos(theta3)*sin(theta4) - 0.35*thetad2*cos(theta1)*cos(theta2)*cos(theta4)*sin(theta3) - 0.35*thetad2*cos(theta1)*cos(theta3)*cos(theta4)*sin(theta2) - 0.35*thetad3*cos(theta1)*cos(theta2)*cos(theta3)*sin(theta4) - 0.35*thetad3*cos(theta1)*cos(theta2)*cos(theta4)*sin(theta3) - 0.35*thetad3*cos(theta1)*cos(theta3)*cos(theta4)*sin(theta2) - 0.049*thetad1*cos(theta2)*cos(theta3)*cos(theta4)*sin(theta5) + 0.8*thetad4*cos(theta1)*cos(theta2)^2*cos(theta3)^2*cos(theta4)^2 + 0.8*thetad5*cos(theta1)*cos(theta2)^2*cos(theta3)^2*cos(theta4)^2 - 0.88*thetad4*cos(theta1)*cos(theta2)*sin(theta1)*sin(theta2) + 0.05*thetad1*cos(theta2)*cos(theta3)*sin(theta1)*sin(theta4) + 0.05*thetad1*cos(theta2)*cos(theta4)*sin(theta1)*sin(theta3) + 0.05*thetad1*cos(theta3)*cos(theta4)*sin(theta1)*sin(theta2) - 0.88*thetad5*cos(theta1)*cos(theta2)*sin(theta1)*sin(theta2) + 0.05*thetad2*cos(theta2)*cos(theta3)*sin(theta1)*sin(theta4) + 0.05*thetad2*cos(theta2)*cos(theta4)*sin(theta1)*sin(theta3) + 0.05*thetad2*cos(theta3)*cos(theta4)*sin(theta1)*sin(theta2) - 0.88*thetad4*cos(theta1)*cos(theta3)*sin(theta1)*sin(theta3) + 0.05*thetad3*cos(theta2)*cos(theta3)*sin(theta1)*sin(theta4) + 0.05*thetad3*cos(theta2)*cos(theta4)*sin(theta1)*sin(theta3) + 0.05*thetad3*cos(theta3)*cos(theta4)*sin(theta1)*sin(theta2) - 0.88*thetad5*cos(theta1)*cos(theta3)*sin(theta1)*sin(theta3) - 0.88*thetad4*cos(theta1)*cos(theta4)*sin(theta1)*sin(theta4) - 0.0098*thetad1*cos(theta2)*cos(theta5)*sin(theta3)*sin(theta4) - 0.0098*thetad1*cos(theta3)*cos(theta5)*sin(theta2)*sin(theta4) - 0.0098*thetad1*cos(theta4)*cos(theta5)*sin(theta2)*sin(theta3) - 0.88*thetad5*cos(theta1)*cos(theta4)*sin(theta1)*sin(theta4) + 5.6*thetad4*cos(theta2)^2*cos(theta3)^2*cos(theta4)^2*sin(theta1) + 5.6*thetad5*cos(theta2)^2*cos(theta3)^2*cos(theta4)^2*sin(theta1) + 0.35*thetad1*cos(theta1)*sin(theta2)*sin(theta3)*sin(theta4) + 0.35*thetad2*cos(theta1)*sin(theta2)*sin(theta3)*sin(theta4) + 0.35*thetad3*cos(theta1)*sin(theta2)*sin(theta3)*sin(theta4) + 0.049*thetad1*cos(theta2)*sin(theta3)*sin(theta4)*sin(theta5) + 0.049*thetad1*cos(theta3)*sin(theta2)*sin(theta4)*sin(theta5) + 0.049*thetad1*cos(theta4)*sin(theta2)*sin(theta3)*sin(theta5) - 0.05*thetad1*sin(theta1)*sin(theta2)*sin(theta3)*sin(theta4) - 0.05*thetad2*sin(theta1)*sin(theta2)*sin(theta3)*sin(theta4) - 0.05*thetad3*sin(theta1)*sin(theta2)*sin(theta3)*sin(theta4) - 0.44*thetad1*cos(theta1)^2*cos(theta2)*cos(theta3)*cos(theta4) - 0.44*thetad2*cos(theta1)^2*cos(theta2)*cos(theta3)*cos(theta4) - 0.44*thetad3*cos(theta1)^2*cos(theta2)*cos(theta3)*cos(theta4) + 0.44*thetad1*cos(theta1)^2*cos(theta2)*sin(theta3)*sin(theta4) + 0.44*thetad1*cos(theta1)^2*cos(theta3)*sin(theta2)*sin(theta4) + 0.44*thetad1*cos(theta1)^2*cos(theta4)*sin(theta2)*sin(theta3) + 0.44*thetad2*cos(theta1)^2*cos(theta2)*sin(theta3)*sin(theta4) + 0.44*thetad2*cos(theta1)^2*cos(theta3)*sin(theta2)*sin(theta4) + 0.44*thetad2*cos(theta1)^2*cos(theta4)*sin(theta2)*sin(theta3) + 0.44*thetad3*cos(theta1)^2*cos(theta2)*sin(theta3)*sin(theta4) + 0.44*thetad3*cos(theta1)^2*cos(theta3)*sin(theta2)*sin(theta4) + 0.44*thetad3*cos(theta1)^2*cos(theta4)*sin(theta2)*sin(theta3) + 1.57*thetad1*cos(theta1)*cos(theta2)*cos(theta3)*cos(theta4)*sin(theta1) + 1.57*thetad2*cos(theta1)*cos(theta2)*cos(theta3)*cos(theta4)*sin(theta1) + 1.57*thetad3*cos(theta1)*cos(theta2)*cos(theta3)*cos(theta4)*sin(theta1) + 0.4*thetad4*cos(theta1)*cos(theta2)*cos(theta3)*sin(theta2)*sin(theta3) + 0.4*thetad5*cos(theta1)*cos(theta2)*cos(theta3)*sin(theta2)*sin(theta3) + 0.4*thetad4*cos(theta1)*cos(theta2)*cos(theta4)*sin(theta2)*sin(theta4) + 0.4*thetad5*cos(theta1)*cos(theta2)*cos(theta4)*sin(theta2)*sin(theta4) + 0.4*thetad4*cos(theta1)*cos(theta3)*cos(theta4)*sin(theta3)*sin(theta4) + 0.4*thetad5*cos(theta1)*cos(theta3)*cos(theta4)*sin(theta3)*sin(theta4) - 12.56*thetad4*cos(theta1)^2*cos(theta2)*cos(theta3)^2*cos(theta4)^2*sin(theta2) - 12.56*thetad4*cos(theta1)^2*cos(theta2)^2*cos(theta3)*cos(theta4)^2*sin(theta3) - 12.56*thetad5*cos(theta1)^2*cos(theta2)*cos(theta3)^2*cos(theta4)^2*sin(theta2) - 12.56*thetad4*cos(theta1)^2*cos(theta2)^2*cos(theta3)^2*cos(theta4)*sin(theta4) - 12.56*thetad5*cos(theta1)^2*cos(theta2)^2*cos(theta3)*cos(theta4)^2*sin(theta3) - 12.56*thetad5*cos(theta1)^2*cos(theta2)^2*cos(theta3)^2*cos(theta4)*sin(theta4) - 1.57*thetad1*cos(theta1)*cos(theta2)*sin(theta1)*sin(theta3)*sin(theta4) - 1.57*thetad1*cos(theta1)*cos(theta3)*sin(theta1)*sin(theta2)*sin(theta4) - 1.57*thetad1*cos(theta1)*cos(theta4)*sin(theta1)*sin(theta2)*sin(theta3) - 1.57*thetad2*cos(theta1)*cos(theta2)*sin(theta1)*sin(theta3)*sin(theta4) - 1.57*thetad2*cos(theta1)*cos(theta3)*sin(theta1)*sin(theta2)*sin(theta4) - 1.57*thetad2*cos(theta1)*cos(theta4)*sin(theta1)*sin(theta2)*sin(theta3) - 1.57*thetad3*cos(theta1)*cos(theta2)*sin(theta1)*sin(theta3)*sin(theta4) - 1.57*thetad3*cos(theta1)*cos(theta3)*sin(theta1)*sin(theta2)*sin(theta4) - 1.57*thetad3*cos(theta1)*cos(theta4)*sin(theta1)*sin(theta2)*sin(theta3) + 2.8*thetad4*cos(theta2)*cos(theta3)*sin(theta1)*sin(theta2)*sin(theta3) + 2.8*thetad5*cos(theta2)*cos(theta3)*sin(theta1)*sin(theta2)*sin(theta3) + 2.8*thetad4*cos(theta2)*cos(theta4)*sin(theta1)*sin(theta2)*sin(theta4) + 2.8*thetad5*cos(theta2)*cos(theta4)*sin(theta1)*sin(theta2)*sin(theta4) + 2.8*thetad4*cos(theta3)*cos(theta4)*sin(theta1)*sin(theta3)*sin(theta4) + 2.8*thetad5*cos(theta3)*cos(theta4)*sin(theta1)*sin(theta3)*sin(theta4) + 1.76*thetad4*cos(theta1)*cos(theta2)*cos(theta3)^2*sin(theta1)*sin(theta2) + 1.76*thetad4*cos(theta1)*cos(theta2)*cos(theta4)^2*sin(theta1)*sin(theta2) + 1.76*thetad4*cos(theta1)*cos(theta2)^2*cos(theta3)*sin(theta1)*sin(theta3) + 1.76*thetad5*cos(theta1)*cos(theta2)*cos(theta3)^2*sin(theta1)*sin(theta2) + 1.76*thetad5*cos(theta1)*cos(theta2)*cos(theta4)^2*sin(theta1)*sin(theta2) + 1.76*thetad5*cos(theta1)*cos(theta2)^2*cos(theta3)*sin(theta1)*sin(theta3) + 1.76*thetad4*cos(theta1)*cos(theta3)*cos(theta4)^2*sin(theta1)*sin(theta3) + 1.76*thetad4*cos(theta1)*cos(theta2)^2*cos(theta4)*sin(theta1)*sin(theta4) + 1.76*thetad4*cos(theta1)*cos(theta3)^2*cos(theta4)*sin(theta1)*sin(theta4) + 1.76*thetad5*cos(theta1)*cos(theta3)*cos(theta4)^2*sin(theta1)*sin(theta3) + 1.76*thetad5*cos(theta1)*cos(theta2)^2*cos(theta4)*sin(theta1)*sin(theta4) + 1.76*thetad5*cos(theta1)*cos(theta3)^2*cos(theta4)*sin(theta1)*sin(theta4) - 11.28*thetad4*cos(theta2)*cos(theta3)*cos(theta4)*sin(theta2)*sin(theta3)*sin(theta4) - 11.28*thetad5*cos(theta2)*cos(theta3)*cos(theta4)*sin(theta2)*sin(theta3)*sin(theta4) - 0.8*thetad4*cos(theta1)*cos(theta2)*cos(theta3)*cos(theta4)^2*sin(theta2)*sin(theta3) - 0.8*thetad4*cos(theta1)*cos(theta2)*cos(theta3)^2*cos(theta4)*sin(theta2)*sin(theta4) - 0.8*thetad5*cos(theta1)*cos(theta2)*cos(theta3)*cos(theta4)^2*sin(theta2)*sin(theta3) - 0.8*thetad4*cos(theta1)*cos(theta2)^2*cos(theta3)*cos(theta4)*sin(theta3)*sin(theta4) - 0.8*thetad5*cos(theta1)*cos(theta2)*cos(theta3)^2*cos(theta4)*sin(theta2)*sin(theta4) - 0.8*thetad5*cos(theta1)*cos(theta2)^2*cos(theta3)*cos(theta4)*sin(theta3)*sin(theta4) - 5.6*thetad4*cos(theta2)*cos(theta3)*cos(theta4)^2*sin(theta1)*sin(theta2)*sin(theta3) - 5.6*thetad4*cos(theta2)*cos(theta3)^2*cos(theta4)*sin(theta1)*sin(theta2)*sin(theta4) - 5.6*thetad5*cos(theta2)*cos(theta3)*cos(theta4)^2*sin(theta1)*sin(theta2)*sin(theta3) - 5.6*thetad4*cos(theta2)^2*cos(theta3)*cos(theta4)*sin(theta1)*sin(theta3)*sin(theta4) - 5.6*thetad5*cos(theta2)*cos(theta3)^2*cos(theta4)*sin(theta1)*sin(theta2)*sin(theta4) - 5.6*thetad5*cos(theta2)^2*cos(theta3)*cos(theta4)*sin(theta1)*sin(theta3)*sin(theta4) - 3.52*thetad4*cos(theta1)*cos(theta2)*cos(theta3)^2*cos(theta4)^2*sin(theta1)*sin(theta2) - 3.52*thetad4*cos(theta1)*cos(theta2)^2*cos(theta3)*cos(theta4)^2*sin(theta1)*sin(theta3) - 3.52*thetad5*cos(theta1)*cos(theta2)*cos(theta3)^2*cos(theta4)^2*sin(theta1)*sin(theta2) - 3.52*thetad4*cos(theta1)*cos(theta2)^2*cos(theta3)^2*cos(theta4)*sin(theta1)*sin(theta4) - 3.52*thetad5*cos(theta1)*cos(theta2)^2*cos(theta3)*cos(theta4)^2*sin(theta1)*sin(theta3) - 3.52*thetad5*cos(theta1)*cos(theta2)^2*cos(theta3)^2*cos(theta4)*sin(theta1)*sin(theta4) + 12.56*thetad4*cos(theta1)^2*cos(theta2)*cos(theta3)*cos(theta4)*sin(theta2)*sin(theta3)*sin(theta4) + 12.56*thetad5*cos(theta1)^2*cos(theta2)*cos(theta3)*cos(theta4)*sin(theta2)*sin(theta3)*sin(theta4) + 3.52*thetad4*cos(theta1)*cos(theta2)*cos(theta3)*cos(theta4)*sin(theta1)*sin(theta2)*sin(theta3)*sin(theta4) + 3.52*thetad5*cos(theta1)*cos(theta2)*cos(theta3)*cos(theta4)*sin(theta1)*sin(theta2)*sin(theta3)*sin(theta4) ;
C(4,1) = 0.206584*thetad1*cos(theta2)^2 - 0.103292*thetad1 + 0.206584*thetad1*cos(theta3)^2 + 0.206584*thetad1*cos(theta4)^2 + 0.4018*thetad1*cos(theta4) - 0.0196*thetad1*cos(theta5) + 0.1666*thetad1*sin(theta4) + 0.098*thetad1*sin(theta5) - 0.413168*thetad1*cos(theta2)^2*cos(theta3)^2 - 0.413168*thetad1*cos(theta2)^2*cos(theta4)^2 - 0.413168*thetad1*cos(theta3)^2*cos(theta4)^2 - 0.060312*thetad1*cos(theta2)*sin(theta2) - 0.060312*thetad1*cos(theta3)*sin(theta3) - 0.060312*thetad1*cos(theta4)*sin(theta4) + 0.028*thetad1*cos(theta5)*sin(theta4) - 0.14*thetad1*sin(theta4)*sin(theta5) - 0.4018*thetad1*cos(theta2)^2*cos(theta4) + 0.0392*thetad1*cos(theta2)^2*cos(theta5) - 0.4018*thetad1*cos(theta3)^2*cos(theta4) + 0.0392*thetad1*cos(theta3)^2*cos(theta5) + 0.0392*thetad1*cos(theta4)^2*cos(theta5) - 0.1666*thetad1*cos(theta2)^2*sin(theta4) - 0.196*thetad1*cos(theta2)^2*sin(theta5) - 0.1666*thetad1*cos(theta3)^2*sin(theta4) - 0.196*thetad1*cos(theta3)^2*sin(theta5) - 0.196*thetad1*cos(theta4)^2*sin(theta5) + 0.8036*thetad1*cos(theta2)^2*cos(theta3)^2*cos(theta4) - 0.0784*thetad1*cos(theta2)^2*cos(theta3)^2*cos(theta5) - 0.0784*thetad1*cos(theta2)^2*cos(theta4)^2*cos(theta5) - 0.0784*thetad1*cos(theta3)^2*cos(theta4)^2*cos(theta5) + 0.3332*thetad1*cos(theta2)^2*cos(theta3)^2*sin(theta4) + 0.392*thetad1*cos(theta2)^2*cos(theta3)^2*sin(theta5) + 0.392*thetad1*cos(theta2)^2*cos(theta4)^2*sin(theta5) + 0.392*thetad1*cos(theta3)^2*cos(theta4)^2*sin(theta5) - 0.190918*thetad2*cos(theta2)*cos(theta3)*cos(theta4) - 0.190918*thetad3*cos(theta2)*cos(theta3)*cos(theta4) + 0.249082*thetad4*cos(theta2)*cos(theta3)*cos(theta4) + 0.22*thetad5*cos(theta2)*cos(theta3)*cos(theta4) - 0.1666*thetad1*cos(theta2)*cos(theta4)*sin(theta2) - 0.1666*thetad1*cos(theta3)*cos(theta4)*sin(theta3) + 0.373674*thetad2*cos(theta2)*cos(theta3)*sin(theta4) + 0.373674*thetad2*cos(theta2)*cos(theta4)*sin(theta3) + 0.373674*thetad2*cos(theta3)*cos(theta4)*sin(theta2) + 0.373674*thetad3*cos(theta2)*cos(theta3)*sin(theta4) + 0.373674*thetad3*cos(theta2)*cos(theta4)*sin(theta3) + 0.373674*thetad3*cos(theta3)*cos(theta4)*sin(theta2) + 0.373674*thetad4*cos(theta2)*cos(theta3)*sin(theta4) + 0.373674*thetad4*cos(theta2)*cos(theta4)*sin(theta3) + 0.373674*thetad4*cos(theta3)*cos(theta4)*sin(theta2) + 0.0728*thetad5*cos(theta2)*cos(theta3)*sin(theta4) + 0.0728*thetad5*cos(theta2)*cos(theta4)*sin(theta3) + 0.0728*thetad5*cos(theta3)*cos(theta4)*sin(theta2) + 0.826336*thetad1*cos(theta2)^2*cos(theta3)^2*cos(theta4)^2 + 0.4018*thetad1*cos(theta2)*sin(theta2)*sin(theta4) + 0.4018*thetad1*cos(theta3)*sin(theta3)*sin(theta4) + 0.190918*thetad2*cos(theta2)*sin(theta3)*sin(theta4) + 0.190918*thetad2*cos(theta3)*sin(theta2)*sin(theta4) + 0.190918*thetad2*cos(theta4)*sin(theta2)*sin(theta3) + 0.190918*thetad3*cos(theta2)*sin(theta3)*sin(theta4) + 0.190918*thetad3*cos(theta3)*sin(theta2)*sin(theta4) + 0.190918*thetad3*cos(theta4)*sin(theta2)*sin(theta3) - 0.249082*thetad4*cos(theta2)*sin(theta3)*sin(theta4) - 0.249082*thetad4*cos(theta3)*sin(theta2)*sin(theta4) - 0.249082*thetad4*cos(theta4)*sin(theta2)*sin(theta3) - 0.22*thetad5*cos(theta2)*sin(theta3)*sin(theta4) - 0.22*thetad5*cos(theta3)*sin(theta2)*sin(theta4) - 0.22*thetad5*cos(theta4)*sin(theta2)*sin(theta3) - 0.373674*thetad2*sin(theta2)*sin(theta3)*sin(theta4) - 0.373674*thetad3*sin(theta2)*sin(theta3)*sin(theta4) - 0.373674*thetad4*sin(theta2)*sin(theta3)*sin(theta4) - 0.0728*thetad5*sin(theta2)*sin(theta3)*sin(theta4) + 0.4018*thetad1*cos(theta2)^2*cos(theta3)*cos(theta4) + 0.120624*thetad1*cos(theta2)*cos(theta3)^2*sin(theta2) + 0.120624*thetad1*cos(theta2)*cos(theta4)^2*sin(theta2) + 0.120624*thetad1*cos(theta2)^2*cos(theta3)*sin(theta3) - 0.1344*thetad1*cos(theta2)*cos(theta5)^2*sin(theta2) + 0.1666*thetad1*cos(theta2)^2*cos(theta3)*sin(theta4) + 0.1666*thetad1*cos(theta2)^2*cos(theta4)*sin(theta3) + 0.120624*thetad1*cos(theta3)*cos(theta4)^2*sin(theta3) + 0.120624*thetad1*cos(theta2)^2*cos(theta4)*sin(theta4) - 0.1344*thetad1*cos(theta3)*cos(theta5)^2*sin(theta3) - 0.028*thetad1*cos(theta2)^2*cos(theta5)*sin(theta4) + 0.120624*thetad1*cos(theta3)^2*cos(theta4)*sin(theta4) - 0.028*thetad1*cos(theta3)^2*cos(theta5)*sin(theta4) - 0.1344*thetad1*cos(theta4)*cos(theta5)^2*sin(theta4) - 0.4018*thetad1*cos(theta2)^2*sin(theta3)*sin(theta4) + 0.14*thetad1*cos(theta2)^2*sin(theta4)*sin(theta5) + 0.14*thetad1*cos(theta3)^2*sin(theta4)*sin(theta5) - 0.241248*thetad1*cos(theta2)*cos(theta3)^2*cos(theta4)^2*sin(theta2) + 0.2688*thetad1*cos(theta2)*cos(theta3)^2*cos(theta5)^2*sin(theta2) - 0.241248*thetad1*cos(theta2)^2*cos(theta3)*cos(theta4)^2*sin(theta3) + 0.2688*thetad1*cos(theta2)*cos(theta4)^2*cos(theta5)^2*sin(theta2) + 0.2688*thetad1*cos(theta2)^2*cos(theta3)*cos(theta5)^2*sin(theta3) - 0.241248*thetad1*cos(theta2)^2*cos(theta3)^2*cos(theta4)*sin(theta4) + 0.056*thetad1*cos(theta2)^2*cos(theta3)^2*cos(theta5)*sin(theta4) + 0.2688*thetad1*cos(theta3)*cos(theta4)^2*cos(theta5)^2*sin(theta3) + 0.2688*thetad1*cos(theta2)^2*cos(theta4)*cos(theta5)^2*sin(theta4) + 0.2688*thetad1*cos(theta3)^2*cos(theta4)*cos(theta5)^2*sin(theta4) - 0.28*thetad1*cos(theta2)^2*cos(theta3)^2*sin(theta4)*sin(theta5) + 0.0098*thetad5*cos(theta2)*cos(theta3)*cos(theta4)*cos(theta5) + 0.1666*thetad1*cos(theta2)*cos(theta3)*cos(theta4)*sin(theta2) - 0.028*thetad1*cos(theta2)*cos(theta4)*cos(theta5)*sin(theta2) - 0.7*thetad4*cos(theta1)*cos(theta2)*cos(theta3)*sin(theta4) - 0.7*thetad4*cos(theta1)*cos(theta2)*cos(theta4)*sin(theta3) - 0.7*thetad4*cos(theta1)*cos(theta3)*cos(theta4)*sin(theta2) - 0.35*thetad5*cos(theta1)*cos(theta2)*cos(theta3)*sin(theta4) - 0.35*thetad5*cos(theta1)*cos(theta2)*cos(theta4)*sin(theta3) - 0.35*thetad5*cos(theta1)*cos(theta3)*cos(theta4)*sin(theta2) - 0.028*thetad1*cos(theta3)*cos(theta4)*cos(theta5)*sin(theta3) + 0.049*thetad2*cos(theta2)*cos(theta3)*cos(theta5)*sin(theta4) + 0.049*thetad2*cos(theta2)*cos(theta4)*cos(theta5)*sin(theta3) + 0.049*thetad2*cos(theta3)*cos(theta4)*cos(theta5)*sin(theta2) + 0.049*thetad3*cos(theta2)*cos(theta3)*cos(theta5)*sin(theta4) + 0.049*thetad3*cos(theta2)*cos(theta4)*cos(theta5)*sin(theta3) + 0.049*thetad3*cos(theta3)*cos(theta4)*cos(theta5)*sin(theta2) + 0.049*thetad4*cos(theta2)*cos(theta3)*cos(theta5)*sin(theta4) + 0.049*thetad4*cos(theta2)*cos(theta4)*cos(theta5)*sin(theta3) + 0.049*thetad4*cos(theta3)*cos(theta4)*cos(theta5)*sin(theta2) - 0.049*thetad5*cos(theta2)*cos(theta3)*cos(theta4)*sin(theta5) + 0.1568*thetad1*cos(theta2)^2*cos(theta3)^2*cos(theta4)^2*cos(theta5) + 0.413168*thetad1*cos(theta2)*cos(theta3)*sin(theta2)*sin(theta3) - 0.4018*thetad1*cos(theta2)*cos(theta3)*sin(theta2)*sin(theta4) - 0.4018*thetad1*cos(theta2)*cos(theta4)*sin(theta2)*sin(theta3) + 0.413168*thetad1*cos(theta2)*cos(theta4)*sin(theta2)*sin(theta4) + 0.14*thetad1*cos(theta2)*cos(theta4)*sin(theta2)*sin(theta5) + 0.1*thetad4*cos(theta2)*cos(theta3)*sin(theta1)*sin(theta4) + 0.1*thetad4*cos(theta2)*cos(theta4)*sin(theta1)*sin(theta3) + 0.1*thetad4*cos(theta3)*cos(theta4)*sin(theta1)*sin(theta2) - 0.056*thetad1*cos(theta2)*cos(theta5)*sin(theta2)*sin(theta5) + 0.413168*thetad1*cos(theta3)*cos(theta4)*sin(theta3)*sin(theta4) + 0.05*thetad5*cos(theta2)*cos(theta3)*sin(theta1)*sin(theta4) + 0.05*thetad5*cos(theta2)*cos(theta4)*sin(theta1)*sin(theta3) + 0.05*thetad5*cos(theta3)*cos(theta4)*sin(theta1)*sin(theta2) + 0.14*thetad1*cos(theta3)*cos(theta4)*sin(theta3)*sin(theta5) + 0.0098*thetad2*cos(theta2)*cos(theta3)*sin(theta4)*sin(theta5) + 0.0098*thetad2*cos(theta2)*cos(theta4)*sin(theta3)*sin(theta5) + 0.0098*thetad2*cos(theta3)*cos(theta4)*sin(theta2)*sin(theta5) - 0.056*thetad1*cos(theta3)*cos(theta5)*sin(theta3)*sin(theta5) + 0.0098*thetad3*cos(theta2)*cos(theta3)*sin(theta4)*sin(theta5) + 0.0098*thetad3*cos(theta2)*cos(theta4)*sin(theta3)*sin(theta5) + 0.0098*thetad3*cos(theta3)*cos(theta4)*sin(theta2)*sin(theta5) + 0.0098*thetad4*cos(theta2)*cos(theta3)*sin(theta4)*sin(theta5) + 0.0098*thetad4*cos(theta2)*cos(theta4)*sin(theta3)*sin(theta5) + 0.0098*thetad4*cos(theta3)*cos(theta4)*sin(theta2)*sin(theta5) - 0.056*thetad1*cos(theta4)*cos(theta5)*sin(theta4)*sin(theta5) - 0.0098*thetad5*cos(theta2)*cos(theta5)*sin(theta3)*sin(theta4) - 0.0098*thetad5*cos(theta3)*cos(theta5)*sin(theta2)*sin(theta4) - 0.0098*thetad5*cos(theta4)*cos(theta5)*sin(theta2)*sin(theta3) - 0.784*thetad1*cos(theta2)^2*cos(theta3)^2*cos(theta4)^2*sin(theta5) - 0.1666*thetad1*cos(theta2)*sin(theta2)*sin(theta3)*sin(theta4) + 0.7*thetad4*cos(theta1)*sin(theta2)*sin(theta3)*sin(theta4) + 0.35*thetad5*cos(theta1)*sin(theta2)*sin(theta3)*sin(theta4) - 0.049*thetad2*cos(theta5)*sin(theta2)*sin(theta3)*sin(theta4) - 0.049*thetad3*cos(theta5)*sin(theta2)*sin(theta3)*sin(theta4) - 0.049*thetad4*cos(theta5)*sin(theta2)*sin(theta3)*sin(theta4) + 0.049*thetad5*cos(theta2)*sin(theta3)*sin(theta4)*sin(theta5) + 0.049*thetad5*cos(theta3)*sin(theta2)*sin(theta4)*sin(theta5) + 0.049*thetad5*cos(theta4)*sin(theta2)*sin(theta3)*sin(theta5) - 0.1*thetad4*sin(theta1)*sin(theta2)*sin(theta3)*sin(theta4) - 0.05*thetad5*sin(theta1)*sin(theta2)*sin(theta3)*sin(theta4) - 0.0098*thetad2*sin(theta2)*sin(theta3)*sin(theta4)*sin(theta5) - 0.0098*thetad3*sin(theta2)*sin(theta3)*sin(theta4)*sin(theta5) - 0.0098*thetad4*sin(theta2)*sin(theta3)*sin(theta4)*sin(theta5) - 0.88*thetad4*cos(theta1)^2*cos(theta2)*cos(theta3)*cos(theta4) - 0.44*thetad5*cos(theta1)^2*cos(theta2)*cos(theta3)*cos(theta4) - 0.028*thetad2*cos(theta2)*cos(theta3)*cos(theta4)*cos(theta5)^2 - 0.028*thetad3*cos(theta2)*cos(theta3)*cos(theta4)*cos(theta5)^2 - 0.028*thetad4*cos(theta2)*cos(theta3)*cos(theta4)*cos(theta5)^2 + 0.3332*thetad1*cos(theta2)*cos(theta3)^2*cos(theta4)*sin(theta2) + 0.3332*thetad1*cos(theta2)^2*cos(theta3)*cos(theta4)*sin(theta3) + 0.028*thetad1*cos(theta2)^2*cos(theta3)*cos(theta5)*sin(theta4) + 0.028*thetad1*cos(theta2)^2*cos(theta4)*cos(theta5)*sin(theta3) - 0.8036*thetad1*cos(theta2)*cos(theta3)^2*sin(theta2)*sin(theta4) - 0.8036*thetad1*cos(theta2)^2*cos(theta3)*sin(theta3)*sin(theta4) + 0.88*thetad4*cos(theta1)^2*cos(theta2)*sin(theta3)*sin(theta4) + 0.88*thetad4*cos(theta1)^2*cos(theta3)*sin(theta2)*sin(theta4) + 0.88*thetad4*cos(theta1)^2*cos(theta4)*sin(theta2)*sin(theta3) - 0.14*thetad1*cos(theta2)^2*cos(theta3)*sin(theta4)*sin(theta5) - 0.14*thetad1*cos(theta2)^2*cos(theta4)*sin(theta3)*sin(theta5) + 0.44*thetad5*cos(theta1)^2*cos(theta2)*sin(theta3)*sin(theta4) + 0.44*thetad5*cos(theta1)^2*cos(theta3)*sin(theta2)*sin(theta4) + 0.44*thetad5*cos(theta1)^2*cos(theta4)*sin(theta2)*sin(theta3) + 0.028*thetad2*cos(theta2)*cos(theta5)^2*sin(theta3)*sin(theta4) + 0.028*thetad2*cos(theta3)*cos(theta5)^2*sin(theta2)*sin(theta4) + 0.028*thetad2*cos(theta4)*cos(theta5)^2*sin(theta2)*sin(theta3) + 0.028*thetad3*cos(theta2)*cos(theta5)^2*sin(theta3)*sin(theta4) + 0.028*thetad3*cos(theta3)*cos(theta5)^2*sin(theta2)*sin(theta4) + 0.028*thetad3*cos(theta4)*cos(theta5)^2*sin(theta2)*sin(theta3) + 0.028*thetad4*cos(theta2)*cos(theta5)^2*sin(theta3)*sin(theta4) + 0.028*thetad4*cos(theta3)*cos(theta5)^2*sin(theta2)*sin(theta4) + 0.028*thetad4*cos(theta4)*cos(theta5)^2*sin(theta2)*sin(theta3) + 3.14*thetad4*cos(theta1)*cos(theta2)*cos(theta3)*cos(theta4)*sin(theta1) + 1.57*thetad5*cos(theta1)*cos(theta2)*cos(theta3)*cos(theta4)*sin(theta1) + 0.028*thetad1*cos(theta2)*cos(theta3)*cos(theta4)*cos(theta5)*sin(theta2) + 0.0672*thetad2*cos(theta2)*cos(theta3)*cos(theta4)*cos(theta5)*sin(theta5) + 0.0672*thetad3*cos(theta2)*cos(theta3)*cos(theta4)*cos(theta5)*sin(theta5) + 0.0672*thetad4*cos(theta2)*cos(theta3)*cos(theta4)*cos(theta5)*sin(theta5) - 0.8036*thetad1*cos(theta2)*cos(theta3)*cos(theta4)*sin(theta2)*sin(theta3) + 0.0784*thetad1*cos(theta2)*cos(theta3)*cos(theta5)*sin(theta2)*sin(theta3) - 0.14*thetad1*cos(theta2)*cos(theta3)*cos(theta4)*sin(theta2)*sin(theta5) + 0.0784*thetad1*cos(theta2)*cos(theta4)*cos(theta5)*sin(theta2)*sin(theta4) + 0.0784*thetad1*cos(theta3)*cos(theta4)*cos(theta5)*sin(theta3)*sin(theta4) - 0.5376*thetad1*cos(theta2)*cos(theta3)^2*cos(theta4)^2*cos(theta5)^2*sin(theta2) - 0.5376*thetad1*cos(theta2)^2*cos(theta3)*cos(theta4)^2*cos(theta5)^2*sin(theta3) - 0.5376*thetad1*cos(theta2)^2*cos(theta3)^2*cos(theta4)*cos(theta5)^2*sin(theta4) - 0.3332*thetad1*cos(theta2)*cos(theta3)*sin(theta2)*sin(theta3)*sin(theta4) - 3.14*thetad4*cos(theta1)*cos(theta2)*sin(theta1)*sin(theta3)*sin(theta4) - 3.14*thetad4*cos(theta1)*cos(theta3)*sin(theta1)*sin(theta2)*sin(theta4) - 3.14*thetad4*cos(theta1)*cos(theta4)*sin(theta1)*sin(theta2)*sin(theta3) - 0.392*thetad1*cos(theta2)*cos(theta3)*sin(theta2)*sin(theta3)*sin(theta5) - 1.57*thetad5*cos(theta1)*cos(theta2)*sin(theta1)*sin(theta3)*sin(theta4) - 1.57*thetad5*cos(theta1)*cos(theta3)*sin(theta1)*sin(theta2)*sin(theta4) - 1.57*thetad5*cos(theta1)*cos(theta4)*sin(theta1)*sin(theta2)*sin(theta3) - 0.028*thetad1*cos(theta2)*cos(theta5)*sin(theta2)*sin(theta3)*sin(theta4) - 0.392*thetad1*cos(theta2)*cos(theta4)*sin(theta2)*sin(theta4)*sin(theta5) - 0.392*thetad1*cos(theta3)*cos(theta4)*sin(theta3)*sin(theta4)*sin(theta5) - 0.0672*thetad2*cos(theta2)*cos(theta5)*sin(theta3)*sin(theta4)*sin(theta5) - 0.0672*thetad2*cos(theta3)*cos(theta5)*sin(theta2)*sin(theta4)*sin(theta5) - 0.0672*thetad2*cos(theta4)*cos(theta5)*sin(theta2)*sin(theta3)*sin(theta5) - 0.0672*thetad3*cos(theta2)*cos(theta5)*sin(theta3)*sin(theta4)*sin(theta5) - 0.0672*thetad3*cos(theta3)*cos(theta5)*sin(theta2)*sin(theta4)*sin(theta5) - 0.0672*thetad3*cos(theta4)*cos(theta5)*sin(theta2)*sin(theta3)*sin(theta5) - 0.0672*thetad4*cos(theta2)*cos(theta5)*sin(theta3)*sin(theta4)*sin(theta5) - 0.0672*thetad4*cos(theta3)*cos(theta5)*sin(theta2)*sin(theta4)*sin(theta5) - 0.0672*thetad4*cos(theta4)*cos(theta5)*sin(theta2)*sin(theta3)*sin(theta5) + 0.14*thetad1*cos(theta2)*sin(theta2)*sin(theta3)*sin(theta4)*sin(theta5) + 0.056*thetad1*cos(theta2)*cos(theta3)^2*cos(theta4)*cos(theta5)*sin(theta2) + 0.056*thetad1*cos(theta2)^2*cos(theta3)*cos(theta4)*cos(theta5)*sin(theta3) - 0.826336*thetad1*cos(theta2)*cos(theta3)*cos(theta4)^2*sin(theta2)*sin(theta3) - 0.826336*thetad1*cos(theta2)*cos(theta3)^2*cos(theta4)*sin(theta2)*sin(theta4) - 0.28*thetad1*cos(theta2)*cos(theta3)^2*cos(theta4)*sin(theta2)*sin(theta5) - 0.826336*thetad1*cos(theta2)^2*cos(theta3)*cos(theta4)*sin(theta3)*sin(theta4) + 0.112*thetad1*cos(theta2)*cos(theta3)^2*cos(theta5)*sin(theta2)*sin(theta5) - 0.28*thetad1*cos(theta2)^2*cos(theta3)*cos(theta4)*sin(theta3)*sin(theta5) + 0.112*thetad1*cos(theta2)*cos(theta4)^2*cos(theta5)*sin(theta2)*sin(theta5) + 0.112*thetad1*cos(theta2)^2*cos(theta3)*cos(theta5)*sin(theta3)*sin(theta5) + 0.112*thetad1*cos(theta3)*cos(theta4)^2*cos(theta5)*sin(theta3)*sin(theta5) + 0.112*thetad1*cos(theta2)^2*cos(theta4)*cos(theta5)*sin(theta4)*sin(theta5) + 0.112*thetad1*cos(theta3)^2*cos(theta4)*cos(theta5)*sin(theta4)*sin(theta5) + 0.241248*thetad1*cos(theta2)*cos(theta3)*cos(theta4)*sin(theta2)*sin(theta3)*sin(theta4) - 0.056*thetad1*cos(theta2)*cos(theta3)*cos(theta5)*sin(theta2)*sin(theta3)*sin(theta4) + 0.28*thetad1*cos(theta2)*cos(theta3)*sin(theta2)*sin(theta3)*sin(theta4)*sin(theta5) - 0.1568*thetad1*cos(theta2)*cos(theta3)*cos(theta4)^2*cos(theta5)*sin(theta2)*sin(theta3) - 0.1568*thetad1*cos(theta2)*cos(theta3)^2*cos(theta4)*cos(theta5)*sin(theta2)*sin(theta4) - 0.1568*thetad1*cos(theta2)^2*cos(theta3)*cos(theta4)*cos(theta5)*sin(theta3)*sin(theta4) + 0.784*thetad1*cos(theta2)*cos(theta3)*cos(theta4)^2*sin(theta2)*sin(theta3)*sin(theta5) + 0.784*thetad1*cos(theta2)*cos(theta3)^2*cos(theta4)*sin(theta2)*sin(theta4)*sin(theta5) + 0.784*thetad1*cos(theta2)^2*cos(theta3)*cos(theta4)*sin(theta3)*sin(theta4)*sin(theta5) - 0.224*thetad1*cos(theta2)*cos(theta3)^2*cos(theta4)^2*cos(theta5)*sin(theta2)*sin(theta5) - 0.224*thetad1*cos(theta2)^2*cos(theta3)*cos(theta4)^2*cos(theta5)*sin(theta3)*sin(theta5) - 0.224*thetad1*cos(theta2)^2*cos(theta3)^2*cos(theta4)*cos(theta5)*sin(theta4)*sin(theta5) + 0.5376*thetad1*cos(theta2)*cos(theta3)*cos(theta4)*cos(theta5)^2*sin(theta2)*sin(theta3)*sin(theta4) + 0.224*thetad1*cos(theta2)*cos(theta3)*cos(theta4)*cos(theta5)*sin(theta2)*sin(theta3)*sin(theta4)*sin(theta5) ;
C(4,2) = 0.4018*thetad2*cos(theta4) + 0.4018*thetad3*cos(theta4) + 0.2009*thetad4*cos(theta4) + 0.1666*thetad2*sin(theta4) + 0.1666*thetad3*sin(theta4) + 0.0833*thetad4*sin(theta4) + 0.4018*thetad2*cos(theta3)*cos(theta4) + 0.2009*thetad3*cos(theta3)*cos(theta4) + 0.2009*thetad4*cos(theta3)*cos(theta4) + 0.07*thetad5*cos(theta4)*cos(theta5) + 0.1666*thetad2*cos(theta3)*sin(theta4) + 0.1666*thetad2*cos(theta4)*sin(theta3) + 0.0833*thetad3*cos(theta3)*sin(theta4) + 0.0833*thetad3*cos(theta4)*sin(theta3) + 0.028*thetad2*cos(theta5)*sin(theta4) + 0.0833*thetad4*cos(theta3)*sin(theta4) + 0.0833*thetad4*cos(theta4)*sin(theta3) + 0.028*thetad3*cos(theta5)*sin(theta4) + 0.014*thetad4*cos(theta5)*sin(theta4) + 0.014*thetad5*cos(theta4)*sin(theta5) - 0.4018*thetad2*sin(theta3)*sin(theta4) - 0.2009*thetad3*sin(theta3)*sin(theta4) - 0.14*thetad2*sin(theta4)*sin(theta5) - 0.2009*thetad4*sin(theta3)*sin(theta4) - 0.14*thetad3*sin(theta4)*sin(theta5) - 0.07*thetad4*sin(theta4)*sin(theta5) - 0.190918*thetad1*cos(theta2)*cos(theta3)*cos(theta4) + 0.44*thetad4*cos(theta2)*cos(theta3)*cos(theta4) + 0.22*thetad5*cos(theta2)*cos(theta3)*cos(theta4) + 0.07*thetad5*cos(theta3)*cos(theta4)*cos(theta5) + 0.373674*thetad1*cos(theta2)*cos(theta3)*sin(theta4) + 0.373674*thetad1*cos(theta2)*cos(theta4)*sin(theta3) + 0.373674*thetad1*cos(theta3)*cos(theta4)*sin(theta2) + 0.028*thetad2*cos(theta3)*cos(theta5)*sin(theta4) + 0.028*thetad2*cos(theta4)*cos(theta5)*sin(theta3) + 0.014*thetad3*cos(theta3)*cos(theta5)*sin(theta4) + 0.014*thetad3*cos(theta4)*cos(theta5)*sin(theta3) + 0.014*thetad4*cos(theta3)*cos(theta5)*sin(theta4) + 0.014*thetad4*cos(theta4)*cos(theta5)*sin(theta3) + 0.014*thetad5*cos(theta3)*cos(theta4)*sin(theta5) + 0.190918*thetad1*cos(theta2)*sin(theta3)*sin(theta4) + 0.190918*thetad1*cos(theta3)*sin(theta2)*sin(theta4) + 0.190918*thetad1*cos(theta4)*sin(theta2)*sin(theta3) - 0.44*thetad4*cos(theta2)*sin(theta3)*sin(theta4) - 0.44*thetad4*cos(theta3)*sin(theta2)*sin(theta4) - 0.44*thetad4*cos(theta4)*sin(theta2)*sin(theta3) - 0.14*thetad2*cos(theta3)*sin(theta4)*sin(theta5) - 0.14*thetad2*cos(theta4)*sin(theta3)*sin(theta5) - 0.22*thetad5*cos(theta2)*sin(theta3)*sin(theta4) - 0.22*thetad5*cos(theta3)*sin(theta2)*sin(theta4) - 0.22*thetad5*cos(theta4)*sin(theta2)*sin(theta3) - 0.07*thetad3*cos(theta3)*sin(theta4)*sin(theta5) - 0.07*thetad3*cos(theta4)*sin(theta3)*sin(theta5) - 0.07*thetad4*cos(theta3)*sin(theta4)*sin(theta5) - 0.07*thetad4*cos(theta4)*sin(theta3)*sin(theta5) - 0.07*thetad5*cos(theta5)*sin(theta3)*sin(theta4) - 0.373674*thetad1*sin(theta2)*sin(theta3)*sin(theta4) - 0.014*thetad5*sin(theta3)*sin(theta4)*sin(theta5) - 0.7*thetad4*cos(theta1)*cos(theta2)*cos(theta3)*sin(theta4) - 0.7*thetad4*cos(theta1)*cos(theta2)*cos(theta4)*sin(theta3) - 0.7*thetad4*cos(theta1)*cos(theta3)*cos(theta4)*sin(theta2) + 0.049*thetad1*cos(theta2)*cos(theta3)*cos(theta5)*sin(theta4) + 0.049*thetad1*cos(theta2)*cos(theta4)*cos(theta5)*sin(theta3) + 0.049*thetad1*cos(theta3)*cos(theta4)*cos(theta5)*sin(theta2) - 0.35*thetad5*cos(theta1)*cos(theta2)*cos(theta3)*sin(theta4) - 0.35*thetad5*cos(theta1)*cos(theta2)*cos(theta4)*sin(theta3) - 0.35*thetad5*cos(theta1)*cos(theta3)*cos(theta4)*sin(theta2) + 0.1*thetad4*cos(theta2)*cos(theta3)*sin(theta1)*sin(theta4) + 0.1*thetad4*cos(theta2)*cos(theta4)*sin(theta1)*sin(theta3) + 0.1*thetad4*cos(theta3)*cos(theta4)*sin(theta1)*sin(theta2) + 0.0098*thetad1*cos(theta2)*cos(theta3)*sin(theta4)*sin(theta5) + 0.0098*thetad1*cos(theta2)*cos(theta4)*sin(theta3)*sin(theta5) + 0.0098*thetad1*cos(theta3)*cos(theta4)*sin(theta2)*sin(theta5) + 0.05*thetad5*cos(theta2)*cos(theta3)*sin(theta1)*sin(theta4) + 0.05*thetad5*cos(theta2)*cos(theta4)*sin(theta1)*sin(theta3) + 0.05*thetad5*cos(theta3)*cos(theta4)*sin(theta1)*sin(theta2) + 0.7*thetad4*cos(theta1)*sin(theta2)*sin(theta3)*sin(theta4) - 0.049*thetad1*cos(theta5)*sin(theta2)*sin(theta3)*sin(theta4) + 0.35*thetad5*cos(theta1)*sin(theta2)*sin(theta3)*sin(theta4) - 0.1*thetad4*sin(theta1)*sin(theta2)*sin(theta3)*sin(theta4) - 0.0098*thetad1*sin(theta2)*sin(theta3)*sin(theta4)*sin(theta5) - 0.05*thetad5*sin(theta1)*sin(theta2)*sin(theta3)*sin(theta4) - 0.88*thetad4*cos(theta1)^2*cos(theta2)*cos(theta3)*cos(theta4) - 0.028*thetad1*cos(theta2)*cos(theta3)*cos(theta4)*cos(theta5)^2 - 0.44*thetad5*cos(theta1)^2*cos(theta2)*cos(theta3)*cos(theta4) + 0.88*thetad4*cos(theta1)^2*cos(theta2)*sin(theta3)*sin(theta4) + 0.88*thetad4*cos(theta1)^2*cos(theta3)*sin(theta2)*sin(theta4) + 0.88*thetad4*cos(theta1)^2*cos(theta4)*sin(theta2)*sin(theta3) + 0.028*thetad1*cos(theta2)*cos(theta5)^2*sin(theta3)*sin(theta4) + 0.028*thetad1*cos(theta3)*cos(theta5)^2*sin(theta2)*sin(theta4) + 0.028*thetad1*cos(theta4)*cos(theta5)^2*sin(theta2)*sin(theta3) + 0.44*thetad5*cos(theta1)^2*cos(theta2)*sin(theta3)*sin(theta4) + 0.44*thetad5*cos(theta1)^2*cos(theta3)*sin(theta2)*sin(theta4) + 0.44*thetad5*cos(theta1)^2*cos(theta4)*sin(theta2)*sin(theta3) + 3.14*thetad4*cos(theta1)*cos(theta2)*cos(theta3)*cos(theta4)*sin(theta1) + 1.57*thetad5*cos(theta1)*cos(theta2)*cos(theta3)*cos(theta4)*sin(theta1) + 0.0672*thetad1*cos(theta2)*cos(theta3)*cos(theta4)*cos(theta5)*sin(theta5) - 3.14*thetad4*cos(theta1)*cos(theta2)*sin(theta1)*sin(theta3)*sin(theta4) - 3.14*thetad4*cos(theta1)*cos(theta3)*sin(theta1)*sin(theta2)*sin(theta4) - 3.14*thetad4*cos(theta1)*cos(theta4)*sin(theta1)*sin(theta2)*sin(theta3) - 1.57*thetad5*cos(theta1)*cos(theta2)*sin(theta1)*sin(theta3)*sin(theta4) - 1.57*thetad5*cos(theta1)*cos(theta3)*sin(theta1)*sin(theta2)*sin(theta4) - 1.57*thetad5*cos(theta1)*cos(theta4)*sin(theta1)*sin(theta2)*sin(theta3) - 0.0672*thetad1*cos(theta2)*cos(theta5)*sin(theta3)*sin(theta4)*sin(theta5) - 0.0672*thetad1*cos(theta3)*cos(theta5)*sin(theta2)*sin(theta4)*sin(theta5) - 0.0672*thetad1*cos(theta4)*cos(theta5)*sin(theta2)*sin(theta3)*sin(theta5) ;
C(4,3) = 0.4018*thetad2*cos(theta4) + 0.4018*thetad3*cos(theta4) + 0.2009*thetad4*cos(theta4) + 0.1666*thetad2*sin(theta4) + 0.1666*thetad3*sin(theta4) + 0.0833*thetad4*sin(theta4) + 0.2009*thetad2*cos(theta3)*cos(theta4) + 0.07*thetad5*cos(theta4)*cos(theta5) + 0.0833*thetad2*cos(theta3)*sin(theta4) + 0.0833*thetad2*cos(theta4)*sin(theta3) + 0.028*thetad2*cos(theta5)*sin(theta4) + 0.028*thetad3*cos(theta5)*sin(theta4) + 0.014*thetad4*cos(theta5)*sin(theta4) + 0.014*thetad5*cos(theta4)*sin(theta5) - 0.2009*thetad2*sin(theta3)*sin(theta4) - 0.14*thetad2*sin(theta4)*sin(theta5) - 0.14*thetad3*sin(theta4)*sin(theta5) - 0.07*thetad4*sin(theta4)*sin(theta5) - 0.190918*thetad1*cos(theta2)*cos(theta3)*cos(theta4) + 0.44*thetad4*cos(theta2)*cos(theta3)*cos(theta4) + 0.22*thetad5*cos(theta2)*cos(theta3)*cos(theta4) + 0.373674*thetad1*cos(theta2)*cos(theta3)*sin(theta4) + 0.373674*thetad1*cos(theta2)*cos(theta4)*sin(theta3) + 0.373674*thetad1*cos(theta3)*cos(theta4)*sin(theta2) + 0.014*thetad2*cos(theta3)*cos(theta5)*sin(theta4) + 0.014*thetad2*cos(theta4)*cos(theta5)*sin(theta3) + 0.190918*thetad1*cos(theta2)*sin(theta3)*sin(theta4) + 0.190918*thetad1*cos(theta3)*sin(theta2)*sin(theta4) + 0.190918*thetad1*cos(theta4)*sin(theta2)*sin(theta3) - 0.44*thetad4*cos(theta2)*sin(theta3)*sin(theta4) - 0.44*thetad4*cos(theta3)*sin(theta2)*sin(theta4) - 0.44*thetad4*cos(theta4)*sin(theta2)*sin(theta3) - 0.07*thetad2*cos(theta3)*sin(theta4)*sin(theta5) - 0.07*thetad2*cos(theta4)*sin(theta3)*sin(theta5) - 0.22*thetad5*cos(theta2)*sin(theta3)*sin(theta4) - 0.22*thetad5*cos(theta3)*sin(theta2)*sin(theta4) - 0.22*thetad5*cos(theta4)*sin(theta2)*sin(theta3) - 0.373674*thetad1*sin(theta2)*sin(theta3)*sin(theta4) - 0.7*thetad4*cos(theta1)*cos(theta2)*cos(theta3)*sin(theta4) - 0.7*thetad4*cos(theta1)*cos(theta2)*cos(theta4)*sin(theta3) - 0.7*thetad4*cos(theta1)*cos(theta3)*cos(theta4)*sin(theta2) + 0.049*thetad1*cos(theta2)*cos(theta3)*cos(theta5)*sin(theta4) + 0.049*thetad1*cos(theta2)*cos(theta4)*cos(theta5)*sin(theta3) + 0.049*thetad1*cos(theta3)*cos(theta4)*cos(theta5)*sin(theta2) - 0.35*thetad5*cos(theta1)*cos(theta2)*cos(theta3)*sin(theta4) - 0.35*thetad5*cos(theta1)*cos(theta2)*cos(theta4)*sin(theta3) - 0.35*thetad5*cos(theta1)*cos(theta3)*cos(theta4)*sin(theta2) + 0.1*thetad4*cos(theta2)*cos(theta3)*sin(theta1)*sin(theta4) + 0.1*thetad4*cos(theta2)*cos(theta4)*sin(theta1)*sin(theta3) + 0.1*thetad4*cos(theta3)*cos(theta4)*sin(theta1)*sin(theta2) + 0.0098*thetad1*cos(theta2)*cos(theta3)*sin(theta4)*sin(theta5) + 0.0098*thetad1*cos(theta2)*cos(theta4)*sin(theta3)*sin(theta5) + 0.0098*thetad1*cos(theta3)*cos(theta4)*sin(theta2)*sin(theta5) + 0.05*thetad5*cos(theta2)*cos(theta3)*sin(theta1)*sin(theta4) + 0.05*thetad5*cos(theta2)*cos(theta4)*sin(theta1)*sin(theta3) + 0.05*thetad5*cos(theta3)*cos(theta4)*sin(theta1)*sin(theta2) + 0.7*thetad4*cos(theta1)*sin(theta2)*sin(theta3)*sin(theta4) - 0.049*thetad1*cos(theta5)*sin(theta2)*sin(theta3)*sin(theta4) + 0.35*thetad5*cos(theta1)*sin(theta2)*sin(theta3)*sin(theta4) - 0.1*thetad4*sin(theta1)*sin(theta2)*sin(theta3)*sin(theta4) - 0.0098*thetad1*sin(theta2)*sin(theta3)*sin(theta4)*sin(theta5) - 0.05*thetad5*sin(theta1)*sin(theta2)*sin(theta3)*sin(theta4) - 0.88*thetad4*cos(theta1)^2*cos(theta2)*cos(theta3)*cos(theta4) - 0.028*thetad1*cos(theta2)*cos(theta3)*cos(theta4)*cos(theta5)^2 - 0.44*thetad5*cos(theta1)^2*cos(theta2)*cos(theta3)*cos(theta4) + 0.88*thetad4*cos(theta1)^2*cos(theta2)*sin(theta3)*sin(theta4) + 0.88*thetad4*cos(theta1)^2*cos(theta3)*sin(theta2)*sin(theta4) + 0.88*thetad4*cos(theta1)^2*cos(theta4)*sin(theta2)*sin(theta3) + 0.028*thetad1*cos(theta2)*cos(theta5)^2*sin(theta3)*sin(theta4) + 0.028*thetad1*cos(theta3)*cos(theta5)^2*sin(theta2)*sin(theta4) + 0.028*thetad1*cos(theta4)*cos(theta5)^2*sin(theta2)*sin(theta3) + 0.44*thetad5*cos(theta1)^2*cos(theta2)*sin(theta3)*sin(theta4) + 0.44*thetad5*cos(theta1)^2*cos(theta3)*sin(theta2)*sin(theta4) + 0.44*thetad5*cos(theta1)^2*cos(theta4)*sin(theta2)*sin(theta3) + 3.14*thetad4*cos(theta1)*cos(theta2)*cos(theta3)*cos(theta4)*sin(theta1) + 1.57*thetad5*cos(theta1)*cos(theta2)*cos(theta3)*cos(theta4)*sin(theta1) + 0.0672*thetad1*cos(theta2)*cos(theta3)*cos(theta4)*cos(theta5)*sin(theta5) - 3.14*thetad4*cos(theta1)*cos(theta2)*sin(theta1)*sin(theta3)*sin(theta4) - 3.14*thetad4*cos(theta1)*cos(theta3)*sin(theta1)*sin(theta2)*sin(theta4) - 3.14*thetad4*cos(theta1)*cos(theta4)*sin(theta1)*sin(theta2)*sin(theta3) - 1.57*thetad5*cos(theta1)*cos(theta2)*sin(theta1)*sin(theta3)*sin(theta4) - 1.57*thetad5*cos(theta1)*cos(theta3)*sin(theta1)*sin(theta2)*sin(theta4) - 1.57*thetad5*cos(theta1)*cos(theta4)*sin(theta1)*sin(theta2)*sin(theta3) - 0.0672*thetad1*cos(theta2)*cos(theta5)*sin(theta3)*sin(theta4)*sin(theta5) - 0.0672*thetad1*cos(theta3)*cos(theta5)*sin(theta2)*sin(theta4)*sin(theta5) - 0.0672*thetad1*cos(theta4)*cos(theta5)*sin(theta2)*sin(theta3)*sin(theta5) ;
C(4,4) = 0.2009*thetad2*cos(theta4) - 0.2*thetad4*cos(theta1) - 0.1*thetad5*cos(theta1) + 0.2009*thetad3*cos(theta4) - 1.4*thetad4*sin(theta1) + 0.0833*thetad2*sin(theta4) - 0.7*thetad5*sin(theta1) + 0.0833*thetad3*sin(theta4) + 0.2009*thetad2*cos(theta3)*cos(theta4) + 5.64*thetad4*cos(theta2)*sin(theta2) + 0.0833*thetad2*cos(theta3)*sin(theta4) + 0.0833*thetad2*cos(theta4)*sin(theta3) + 2.82*thetad5*cos(theta2)*sin(theta2) + 5.64*thetad4*cos(theta3)*sin(theta3) + 0.014*thetad2*cos(theta5)*sin(theta4) + 2.82*thetad5*cos(theta3)*sin(theta3) + 0.014*thetad3*cos(theta5)*sin(theta4) + 5.64*thetad4*cos(theta4)*sin(theta4) + 2.82*thetad5*cos(theta4)*sin(theta4) - 0.2009*thetad2*sin(theta3)*sin(theta4) - 0.07*thetad2*sin(theta4)*sin(theta5) - 0.07*thetad3*sin(theta4)*sin(theta5) + 0.4*thetad4*cos(theta1)*cos(theta2)^2 + 0.4*thetad4*cos(theta1)*cos(theta3)^2 + 0.2*thetad5*cos(theta1)*cos(theta2)^2 + 0.4*thetad4*cos(theta1)*cos(theta4)^2 + 0.2*thetad5*cos(theta1)*cos(theta3)^2 + 0.2*thetad5*cos(theta1)*cos(theta4)^2 + 2.8*thetad4*cos(theta2)^2*sin(theta1) + 2.8*thetad4*cos(theta3)^2*sin(theta1) + 1.4*thetad5*cos(theta2)^2*sin(theta1) + 2.8*thetad4*cos(theta4)^2*sin(theta1) + 1.4*thetad5*cos(theta3)^2*sin(theta1) + 1.4*thetad5*cos(theta4)^2*sin(theta1) - 0.8*thetad4*cos(theta1)*cos(theta2)^2*cos(theta3)^2 - 0.8*thetad4*cos(theta1)*cos(theta2)^2*cos(theta4)^2 - 0.4*thetad5*cos(theta1)*cos(theta2)^2*cos(theta3)^2 - 0.8*thetad4*cos(theta1)*cos(theta3)^2*cos(theta4)^2 - 0.4*thetad5*cos(theta1)*cos(theta2)^2*cos(theta4)^2 - 0.4*thetad5*cos(theta1)*cos(theta3)^2*cos(theta4)^2 - 5.6*thetad4*cos(theta2)^2*cos(theta3)^2*sin(theta1) - 5.6*thetad4*cos(theta2)^2*cos(theta4)^2*sin(theta1) - 2.8*thetad5*cos(theta2)^2*cos(theta3)^2*sin(theta1) - 5.6*thetad4*cos(theta3)^2*cos(theta4)^2*sin(theta1) - 2.8*thetad5*cos(theta2)^2*cos(theta4)^2*sin(theta1) - 2.8*thetad5*cos(theta3)^2*cos(theta4)^2*sin(theta1) + 0.249082*thetad1*cos(theta2)*cos(theta3)*cos(theta4) + 0.44*thetad2*cos(theta2)*cos(theta3)*cos(theta4) + 0.44*thetad3*cos(theta2)*cos(theta3)*cos(theta4) + 0.373674*thetad1*cos(theta2)*cos(theta3)*sin(theta4) + 0.373674*thetad1*cos(theta2)*cos(theta4)*sin(theta3) + 0.373674*thetad1*cos(theta3)*cos(theta4)*sin(theta2) + 0.014*thetad2*cos(theta3)*cos(theta5)*sin(theta4) + 0.014*thetad2*cos(theta4)*cos(theta5)*sin(theta3) - 0.249082*thetad1*cos(theta2)*sin(theta3)*sin(theta4) - 0.249082*thetad1*cos(theta3)*sin(theta2)*sin(theta4) - 0.249082*thetad1*cos(theta4)*sin(theta2)*sin(theta3) - 0.44*thetad2*cos(theta2)*sin(theta3)*sin(theta4) - 0.44*thetad2*cos(theta3)*sin(theta2)*sin(theta4) - 0.44*thetad2*cos(theta4)*sin(theta2)*sin(theta3) - 0.44*thetad3*cos(theta2)*sin(theta3)*sin(theta4) - 0.44*thetad3*cos(theta3)*sin(theta2)*sin(theta4) - 0.44*thetad3*cos(theta4)*sin(theta2)*sin(theta3) - 0.07*thetad2*cos(theta3)*sin(theta4)*sin(theta5) - 0.07*thetad2*cos(theta4)*sin(theta3)*sin(theta5) - 0.373674*thetad1*sin(theta2)*sin(theta3)*sin(theta4) - 6.28*thetad4*cos(theta1)^2*cos(theta2)*sin(theta2) - 3.14*thetad5*cos(theta1)^2*cos(theta2)*sin(theta2) - 11.28*thetad4*cos(theta2)*cos(theta3)^2*sin(theta2) - 6.28*thetad4*cos(theta1)^2*cos(theta3)*sin(theta3) - 11.28*thetad4*cos(theta2)*cos(theta4)^2*sin(theta2) - 11.28*thetad4*cos(theta2)^2*cos(theta3)*sin(theta3) - 5.64*thetad5*cos(theta2)*cos(theta3)^2*sin(theta2) - 3.14*thetad5*cos(theta1)^2*cos(theta3)*sin(theta3) - 6.28*thetad4*cos(theta1)^2*cos(theta4)*sin(theta4) - 5.64*thetad5*cos(theta2)*cos(theta4)^2*sin(theta2) - 5.64*thetad5*cos(theta2)^2*cos(theta3)*sin(theta3) - 11.28*thetad4*cos(theta3)*cos(theta4)^2*sin(theta3) - 11.28*thetad4*cos(theta2)^2*cos(theta4)*sin(theta4) - 3.14*thetad5*cos(theta1)^2*cos(theta4)*sin(theta4) - 11.28*thetad4*cos(theta3)^2*cos(theta4)*sin(theta4) - 5.64*thetad5*cos(theta3)*cos(theta4)^2*sin(theta3) - 5.64*thetad5*cos(theta2)^2*cos(theta4)*sin(theta4) - 5.64*thetad5*cos(theta3)^2*cos(theta4)*sin(theta4) + 12.56*thetad4*cos(theta1)^2*cos(theta2)*cos(theta3)^2*sin(theta2) + 12.56*thetad4*cos(theta1)^2*cos(theta2)*cos(theta4)^2*sin(theta2) + 12.56*thetad4*cos(theta1)^2*cos(theta2)^2*cos(theta3)*sin(theta3) + 6.28*thetad5*cos(theta1)^2*cos(theta2)*cos(theta3)^2*sin(theta2) + 6.28*thetad5*cos(theta1)^2*cos(theta2)*cos(theta4)^2*sin(theta2) + 6.28*thetad5*cos(theta1)^2*cos(theta2)^2*cos(theta3)*sin(theta3) + 22.56*thetad4*cos(theta2)*cos(theta3)^2*cos(theta4)^2*sin(theta2) + 12.56*thetad4*cos(theta1)^2*cos(theta3)*cos(theta4)^2*sin(theta3) + 12.56*thetad4*cos(theta1)^2*cos(theta2)^2*cos(theta4)*sin(theta4) + 12.56*thetad4*cos(theta1)^2*cos(theta3)^2*cos(theta4)*sin(theta4) + 22.56*thetad4*cos(theta2)^2*cos(theta3)*cos(theta4)^2*sin(theta3) + 11.28*thetad5*cos(theta2)*cos(theta3)^2*cos(theta4)^2*sin(theta2) + 6.28*thetad5*cos(theta1)^2*cos(theta3)*cos(theta4)^2*sin(theta3) + 6.28*thetad5*cos(theta1)^2*cos(theta2)^2*cos(theta4)*sin(theta4) + 22.56*thetad4*cos(theta2)^2*cos(theta3)^2*cos(theta4)*sin(theta4) + 6.28*thetad5*cos(theta1)^2*cos(theta3)^2*cos(theta4)*sin(theta4) + 11.28*thetad5*cos(theta2)^2*cos(theta3)*cos(theta4)^2*sin(theta3) + 11.28*thetad5*cos(theta2)^2*cos(theta3)^2*cos(theta4)*sin(theta4) - 0.7*thetad1*cos(theta1)*cos(theta2)*cos(theta3)*sin(theta4) - 0.7*thetad1*cos(theta1)*cos(theta2)*cos(theta4)*sin(theta3) - 0.7*thetad1*cos(theta1)*cos(theta3)*cos(theta4)*sin(theta2) - 0.7*thetad2*cos(theta1)*cos(theta2)*cos(theta3)*sin(theta4) - 0.7*thetad2*cos(theta1)*cos(theta2)*cos(theta4)*sin(theta3) - 0.7*thetad2*cos(theta1)*cos(theta3)*cos(theta4)*sin(theta2) - 0.7*thetad3*cos(theta1)*cos(theta2)*cos(theta3)*sin(theta4) - 0.7*thetad3*cos(theta1)*cos(theta2)*cos(theta4)*sin(theta3) - 0.7*thetad3*cos(theta1)*cos(theta3)*cos(theta4)*sin(theta2) + 0.049*thetad1*cos(theta2)*cos(theta3)*cos(theta5)*sin(theta4) + 0.049*thetad1*cos(theta2)*cos(theta4)*cos(theta5)*sin(theta3) + 0.049*thetad1*cos(theta3)*cos(theta4)*cos(theta5)*sin(theta2) + 1.6*thetad4*cos(theta1)*cos(theta2)^2*cos(theta3)^2*cos(theta4)^2 + 0.8*thetad5*cos(theta1)*cos(theta2)^2*cos(theta3)^2*cos(theta4)^2 - 1.76*thetad4*cos(theta1)*cos(theta2)*sin(theta1)*sin(theta2) + 0.1*thetad1*cos(theta2)*cos(theta3)*sin(theta1)*sin(theta4) + 0.1*thetad1*cos(theta2)*cos(theta4)*sin(theta1)*sin(theta3) + 0.1*thetad1*cos(theta3)*cos(theta4)*sin(theta1)*sin(theta2) - 0.88*thetad5*cos(theta1)*cos(theta2)*sin(theta1)*sin(theta2) + 0.1*thetad2*cos(theta2)*cos(theta3)*sin(theta1)*sin(theta4) + 0.1*thetad2*cos(theta2)*cos(theta4)*sin(theta1)*sin(theta3) + 0.1*thetad2*cos(theta3)*cos(theta4)*sin(theta1)*sin(theta2) - 1.76*thetad4*cos(theta1)*cos(theta3)*sin(theta1)*sin(theta3) + 0.1*thetad3*cos(theta2)*cos(theta3)*sin(theta1)*sin(theta4) + 0.1*thetad3*cos(theta2)*cos(theta4)*sin(theta1)*sin(theta3) + 0.1*thetad3*cos(theta3)*cos(theta4)*sin(theta1)*sin(theta2) - 0.88*thetad5*cos(theta1)*cos(theta3)*sin(theta1)*sin(theta3) - 1.76*thetad4*cos(theta1)*cos(theta4)*sin(theta1)*sin(theta4) + 0.0098*thetad1*cos(theta2)*cos(theta3)*sin(theta4)*sin(theta5) + 0.0098*thetad1*cos(theta2)*cos(theta4)*sin(theta3)*sin(theta5) + 0.0098*thetad1*cos(theta3)*cos(theta4)*sin(theta2)*sin(theta5) - 0.88*thetad5*cos(theta1)*cos(theta4)*sin(theta1)*sin(theta4) + 11.2*thetad4*cos(theta2)^2*cos(theta3)^2*cos(theta4)^2*sin(theta1) + 5.6*thetad5*cos(theta2)^2*cos(theta3)^2*cos(theta4)^2*sin(theta1) + 0.7*thetad1*cos(theta1)*sin(theta2)*sin(theta3)*sin(theta4) + 0.7*thetad2*cos(theta1)*sin(theta2)*sin(theta3)*sin(theta4) + 0.7*thetad3*cos(theta1)*sin(theta2)*sin(theta3)*sin(theta4) - 0.049*thetad1*cos(theta5)*sin(theta2)*sin(theta3)*sin(theta4) - 0.1*thetad1*sin(theta1)*sin(theta2)*sin(theta3)*sin(theta4) - 0.1*thetad2*sin(theta1)*sin(theta2)*sin(theta3)*sin(theta4) - 0.1*thetad3*sin(theta1)*sin(theta2)*sin(theta3)*sin(theta4) - 0.0098*thetad1*sin(theta2)*sin(theta3)*sin(theta4)*sin(theta5) - 0.88*thetad1*cos(theta1)^2*cos(theta2)*cos(theta3)*cos(theta4) - 0.88*thetad2*cos(theta1)^2*cos(theta2)*cos(theta3)*cos(theta4) - 0.88*thetad3*cos(theta1)^2*cos(theta2)*cos(theta3)*cos(theta4) - 0.028*thetad1*cos(theta2)*cos(theta3)*cos(theta4)*cos(theta5)^2 + 0.88*thetad1*cos(theta1)^2*cos(theta2)*sin(theta3)*sin(theta4) + 0.88*thetad1*cos(theta1)^2*cos(theta3)*sin(theta2)*sin(theta4) + 0.88*thetad1*cos(theta1)^2*cos(theta4)*sin(theta2)*sin(theta3) + 0.88*thetad2*cos(theta1)^2*cos(theta2)*sin(theta3)*sin(theta4) + 0.88*thetad2*cos(theta1)^2*cos(theta3)*sin(theta2)*sin(theta4) + 0.88*thetad2*cos(theta1)^2*cos(theta4)*sin(theta2)*sin(theta3) + 0.88*thetad3*cos(theta1)^2*cos(theta2)*sin(theta3)*sin(theta4) + 0.88*thetad3*cos(theta1)^2*cos(theta3)*sin(theta2)*sin(theta4) + 0.88*thetad3*cos(theta1)^2*cos(theta4)*sin(theta2)*sin(theta3) + 0.028*thetad1*cos(theta2)*cos(theta5)^2*sin(theta3)*sin(theta4) + 0.028*thetad1*cos(theta3)*cos(theta5)^2*sin(theta2)*sin(theta4) + 0.028*thetad1*cos(theta4)*cos(theta5)^2*sin(theta2)*sin(theta3) + 3.14*thetad1*cos(theta1)*cos(theta2)*cos(theta3)*cos(theta4)*sin(theta1) + 3.14*thetad2*cos(theta1)*cos(theta2)*cos(theta3)*cos(theta4)*sin(theta1) + 3.14*thetad3*cos(theta1)*cos(theta2)*cos(theta3)*cos(theta4)*sin(theta1) + 0.0672*thetad1*cos(theta2)*cos(theta3)*cos(theta4)*cos(theta5)*sin(theta5) + 0.8*thetad4*cos(theta1)*cos(theta2)*cos(theta3)*sin(theta2)*sin(theta3) + 0.4*thetad5*cos(theta1)*cos(theta2)*cos(theta3)*sin(theta2)*sin(theta3) + 0.8*thetad4*cos(theta1)*cos(theta2)*cos(theta4)*sin(theta2)*sin(theta4) + 0.4*thetad5*cos(theta1)*cos(theta2)*cos(theta4)*sin(theta2)*sin(theta4) + 0.8*thetad4*cos(theta1)*cos(theta3)*cos(theta4)*sin(theta3)*sin(theta4) + 0.4*thetad5*cos(theta1)*cos(theta3)*cos(theta4)*sin(theta3)*sin(theta4) - 25.12*thetad4*cos(theta1)^2*cos(theta2)*cos(theta3)^2*cos(theta4)^2*sin(theta2) - 25.12*thetad4*cos(theta1)^2*cos(theta2)^2*cos(theta3)*cos(theta4)^2*sin(theta3) - 12.56*thetad5*cos(theta1)^2*cos(theta2)*cos(theta3)^2*cos(theta4)^2*sin(theta2) - 25.12*thetad4*cos(theta1)^2*cos(theta2)^2*cos(theta3)^2*cos(theta4)*sin(theta4) - 12.56*thetad5*cos(theta1)^2*cos(theta2)^2*cos(theta3)*cos(theta4)^2*sin(theta3) - 12.56*thetad5*cos(theta1)^2*cos(theta2)^2*cos(theta3)^2*cos(theta4)*sin(theta4) - 3.14*thetad1*cos(theta1)*cos(theta2)*sin(theta1)*sin(theta3)*sin(theta4) - 3.14*thetad1*cos(theta1)*cos(theta3)*sin(theta1)*sin(theta2)*sin(theta4) - 3.14*thetad1*cos(theta1)*cos(theta4)*sin(theta1)*sin(theta2)*sin(theta3) - 3.14*thetad2*cos(theta1)*cos(theta2)*sin(theta1)*sin(theta3)*sin(theta4) - 3.14*thetad2*cos(theta1)*cos(theta3)*sin(theta1)*sin(theta2)*sin(theta4) - 3.14*thetad2*cos(theta1)*cos(theta4)*sin(theta1)*sin(theta2)*sin(theta3) - 3.14*thetad3*cos(theta1)*cos(theta2)*sin(theta1)*sin(theta3)*sin(theta4) - 3.14*thetad3*cos(theta1)*cos(theta3)*sin(theta1)*sin(theta2)*sin(theta4) - 3.14*thetad3*cos(theta1)*cos(theta4)*sin(theta1)*sin(theta2)*sin(theta3) + 5.6*thetad4*cos(theta2)*cos(theta3)*sin(theta1)*sin(theta2)*sin(theta3) + 2.8*thetad5*cos(theta2)*cos(theta3)*sin(theta1)*sin(theta2)*sin(theta3) + 5.6*thetad4*cos(theta2)*cos(theta4)*sin(theta1)*sin(theta2)*sin(theta4) + 2.8*thetad5*cos(theta2)*cos(theta4)*sin(theta1)*sin(theta2)*sin(theta4) + 5.6*thetad4*cos(theta3)*cos(theta4)*sin(theta1)*sin(theta3)*sin(theta4) - 0.0672*thetad1*cos(theta2)*cos(theta5)*sin(theta3)*sin(theta4)*sin(theta5) - 0.0672*thetad1*cos(theta3)*cos(theta5)*sin(theta2)*sin(theta4)*sin(theta5) - 0.0672*thetad1*cos(theta4)*cos(theta5)*sin(theta2)*sin(theta3)*sin(theta5) + 2.8*thetad5*cos(theta3)*cos(theta4)*sin(theta1)*sin(theta3)*sin(theta4) + 3.52*thetad4*cos(theta1)*cos(theta2)*cos(theta3)^2*sin(theta1)*sin(theta2) + 3.52*thetad4*cos(theta1)*cos(theta2)*cos(theta4)^2*sin(theta1)*sin(theta2) + 3.52*thetad4*cos(theta1)*cos(theta2)^2*cos(theta3)*sin(theta1)*sin(theta3) + 1.76*thetad5*cos(theta1)*cos(theta2)*cos(theta3)^2*sin(theta1)*sin(theta2) + 1.76*thetad5*cos(theta1)*cos(theta2)*cos(theta4)^2*sin(theta1)*sin(theta2) + 1.76*thetad5*cos(theta1)*cos(theta2)^2*cos(theta3)*sin(theta1)*sin(theta3) + 3.52*thetad4*cos(theta1)*cos(theta3)*cos(theta4)^2*sin(theta1)*sin(theta3) + 3.52*thetad4*cos(theta1)*cos(theta2)^2*cos(theta4)*sin(theta1)*sin(theta4) + 3.52*thetad4*cos(theta1)*cos(theta3)^2*cos(theta4)*sin(theta1)*sin(theta4) + 1.76*thetad5*cos(theta1)*cos(theta3)*cos(theta4)^2*sin(theta1)*sin(theta3) + 1.76*thetad5*cos(theta1)*cos(theta2)^2*cos(theta4)*sin(theta1)*sin(theta4) + 1.76*thetad5*cos(theta1)*cos(theta3)^2*cos(theta4)*sin(theta1)*sin(theta4) - 22.56*thetad4*cos(theta2)*cos(theta3)*cos(theta4)*sin(theta2)*sin(theta3)*sin(theta4) - 11.28*thetad5*cos(theta2)*cos(theta3)*cos(theta4)*sin(theta2)*sin(theta3)*sin(theta4) - 1.6*thetad4*cos(theta1)*cos(theta2)*cos(theta3)*cos(theta4)^2*sin(theta2)*sin(theta3) - 1.6*thetad4*cos(theta1)*cos(theta2)*cos(theta3)^2*cos(theta4)*sin(theta2)*sin(theta4) - 0.8*thetad5*cos(theta1)*cos(theta2)*cos(theta3)*cos(theta4)^2*sin(theta2)*sin(theta3) - 1.6*thetad4*cos(theta1)*cos(theta2)^2*cos(theta3)*cos(theta4)*sin(theta3)*sin(theta4) - 0.8*thetad5*cos(theta1)*cos(theta2)*cos(theta3)^2*cos(theta4)*sin(theta2)*sin(theta4) - 0.8*thetad5*cos(theta1)*cos(theta2)^2*cos(theta3)*cos(theta4)*sin(theta3)*sin(theta4) - 11.2*thetad4*cos(theta2)*cos(theta3)*cos(theta4)^2*sin(theta1)*sin(theta2)*sin(theta3) - 11.2*thetad4*cos(theta2)*cos(theta3)^2*cos(theta4)*sin(theta1)*sin(theta2)*sin(theta4) - 5.6*thetad5*cos(theta2)*cos(theta3)*cos(theta4)^2*sin(theta1)*sin(theta2)*sin(theta3) - 11.2*thetad4*cos(theta2)^2*cos(theta3)*cos(theta4)*sin(theta1)*sin(theta3)*sin(theta4) - 5.6*thetad5*cos(theta2)*cos(theta3)^2*cos(theta4)*sin(theta1)*sin(theta2)*sin(theta4) - 5.6*thetad5*cos(theta2)^2*cos(theta3)*cos(theta4)*sin(theta1)*sin(theta3)*sin(theta4) - 7.04*thetad4*cos(theta1)*cos(theta2)*cos(theta3)^2*cos(theta4)^2*sin(theta1)*sin(theta2) - 7.04*thetad4*cos(theta1)*cos(theta2)^2*cos(theta3)*cos(theta4)^2*sin(theta1)*sin(theta3) - 3.52*thetad5*cos(theta1)*cos(theta2)*cos(theta3)^2*cos(theta4)^2*sin(theta1)*sin(theta2) - 7.04*thetad4*cos(theta1)*cos(theta2)^2*cos(theta3)^2*cos(theta4)*sin(theta1)*sin(theta4) - 3.52*thetad5*cos(theta1)*cos(theta2)^2*cos(theta3)*cos(theta4)^2*sin(theta1)*sin(theta3) - 3.52*thetad5*cos(theta1)*cos(theta2)^2*cos(theta3)^2*cos(theta4)*sin(theta1)*sin(theta4) + 25.12*thetad4*cos(theta1)^2*cos(theta2)*cos(theta3)*cos(theta4)*sin(theta2)*sin(theta3)*sin(theta4) + 12.56*thetad5*cos(theta1)^2*cos(theta2)*cos(theta3)*cos(theta4)*sin(theta2)*sin(theta3)*sin(theta4) + 7.04*thetad4*cos(theta1)*cos(theta2)*cos(theta3)*cos(theta4)*sin(theta1)*sin(theta2)*sin(theta3)*sin(theta4) + 3.52*thetad5*cos(theta1)*cos(theta2)*cos(theta3)*cos(theta4)*sin(theta1)*sin(theta2)*sin(theta3)*sin(theta4) ;
C(4,5) = 0.07*thetad2*cos(theta4)*cos(theta5) - 0.1*thetad5*cos(theta1) - 0.7*thetad4*sin(theta1) - 0.7*thetad5*sin(theta1) - 0.1*thetad4*cos(theta1) + 0.07*thetad3*cos(theta4)*cos(theta5) + 2.82*thetad4*cos(theta2)*sin(theta2) + 2.82*thetad5*cos(theta2)*sin(theta2) + 2.82*thetad4*cos(theta3)*sin(theta3) + 0.014*thetad2*cos(theta4)*sin(theta5) + 2.82*thetad5*cos(theta3)*sin(theta3) + 0.014*thetad3*cos(theta4)*sin(theta5) + 2.82*thetad4*cos(theta4)*sin(theta4) + 2.82*thetad5*cos(theta4)*sin(theta4) + 0.2*thetad4*cos(theta1)*cos(theta2)^2 + 0.2*thetad4*cos(theta1)*cos(theta3)^2 + 0.2*thetad5*cos(theta1)*cos(theta2)^2 + 0.2*thetad4*cos(theta1)*cos(theta4)^2 + 0.2*thetad5*cos(theta1)*cos(theta3)^2 + 0.2*thetad5*cos(theta1)*cos(theta4)^2 + 1.4*thetad4*cos(theta2)^2*sin(theta1) + 1.4*thetad4*cos(theta3)^2*sin(theta1) + 1.4*thetad5*cos(theta2)^2*sin(theta1) + 1.4*thetad4*cos(theta4)^2*sin(theta1) + 1.4*thetad5*cos(theta3)^2*sin(theta1) + 1.4*thetad5*cos(theta4)^2*sin(theta1) - 0.4*thetad4*cos(theta1)*cos(theta2)^2*cos(theta3)^2 - 0.4*thetad4*cos(theta1)*cos(theta2)^2*cos(theta4)^2 - 0.4*thetad5*cos(theta1)*cos(theta2)^2*cos(theta3)^2 - 0.4*thetad4*cos(theta1)*cos(theta3)^2*cos(theta4)^2 - 0.4*thetad5*cos(theta1)*cos(theta2)^2*cos(theta4)^2 - 0.4*thetad5*cos(theta1)*cos(theta3)^2*cos(theta4)^2 - 2.8*thetad4*cos(theta2)^2*cos(theta3)^2*sin(theta1) - 2.8*thetad4*cos(theta2)^2*cos(theta4)^2*sin(theta1) - 2.8*thetad5*cos(theta2)^2*cos(theta3)^2*sin(theta1) - 2.8*thetad4*cos(theta3)^2*cos(theta4)^2*sin(theta1) - 2.8*thetad5*cos(theta2)^2*cos(theta4)^2*sin(theta1) - 2.8*thetad5*cos(theta3)^2*cos(theta4)^2*sin(theta1) + 0.22*thetad1*cos(theta2)*cos(theta3)*cos(theta4) + 0.22*thetad2*cos(theta2)*cos(theta3)*cos(theta4) + 0.22*thetad3*cos(theta2)*cos(theta3)*cos(theta4) + 0.07*thetad2*cos(theta3)*cos(theta4)*cos(theta5) + 0.0728*thetad1*cos(theta2)*cos(theta3)*sin(theta4) + 0.0728*thetad1*cos(theta2)*cos(theta4)*sin(theta3) + 0.0728*thetad1*cos(theta3)*cos(theta4)*sin(theta2) + 0.014*thetad2*cos(theta3)*cos(theta4)*sin(theta5) - 0.22*thetad1*cos(theta2)*sin(theta3)*sin(theta4) - 0.22*thetad1*cos(theta3)*sin(theta2)*sin(theta4) - 0.22*thetad1*cos(theta4)*sin(theta2)*sin(theta3) - 0.22*thetad2*cos(theta2)*sin(theta3)*sin(theta4) - 0.22*thetad2*cos(theta3)*sin(theta2)*sin(theta4) - 0.22*thetad2*cos(theta4)*sin(theta2)*sin(theta3) - 0.22*thetad3*cos(theta2)*sin(theta3)*sin(theta4) - 0.22*thetad3*cos(theta3)*sin(theta2)*sin(theta4) - 0.22*thetad3*cos(theta4)*sin(theta2)*sin(theta3) - 0.07*thetad2*cos(theta5)*sin(theta3)*sin(theta4) - 0.0728*thetad1*sin(theta2)*sin(theta3)*sin(theta4) - 0.014*thetad2*sin(theta3)*sin(theta4)*sin(theta5) - 3.14*thetad4*cos(theta1)^2*cos(theta2)*sin(theta2) - 3.14*thetad5*cos(theta1)^2*cos(theta2)*sin(theta2) - 5.64*thetad4*cos(theta2)*cos(theta3)^2*sin(theta2) - 3.14*thetad4*cos(theta1)^2*cos(theta3)*sin(theta3) - 5.64*thetad4*cos(theta2)*cos(theta4)^2*sin(theta2) - 5.64*thetad4*cos(theta2)^2*cos(theta3)*sin(theta3) - 5.64*thetad5*cos(theta2)*cos(theta3)^2*sin(theta2) - 3.14*thetad5*cos(theta1)^2*cos(theta3)*sin(theta3) - 3.14*thetad4*cos(theta1)^2*cos(theta4)*sin(theta4) - 5.64*thetad5*cos(theta2)*cos(theta4)^2*sin(theta2) - 5.64*thetad5*cos(theta2)^2*cos(theta3)*sin(theta3) - 5.64*thetad4*cos(theta3)*cos(theta4)^2*sin(theta3) - 5.64*thetad4*cos(theta2)^2*cos(theta4)*sin(theta4) - 3.14*thetad5*cos(theta1)^2*cos(theta4)*sin(theta4) - 5.64*thetad4*cos(theta3)^2*cos(theta4)*sin(theta4) - 5.64*thetad5*cos(theta3)*cos(theta4)^2*sin(theta3) - 5.64*thetad5*cos(theta2)^2*cos(theta4)*sin(theta4) - 5.64*thetad5*cos(theta3)^2*cos(theta4)*sin(theta4) + 6.28*thetad4*cos(theta1)^2*cos(theta2)*cos(theta3)^2*sin(theta2) + 6.28*thetad4*cos(theta1)^2*cos(theta2)*cos(theta4)^2*sin(theta2) + 6.28*thetad4*cos(theta1)^2*cos(theta2)^2*cos(theta3)*sin(theta3) + 6.28*thetad5*cos(theta1)^2*cos(theta2)*cos(theta3)^2*sin(theta2) + 6.28*thetad5*cos(theta1)^2*cos(theta2)*cos(theta4)^2*sin(theta2) + 6.28*thetad5*cos(theta1)^2*cos(theta2)^2*cos(theta3)*sin(theta3) + 11.28*thetad4*cos(theta2)*cos(theta3)^2*cos(theta4)^2*sin(theta2) + 6.28*thetad4*cos(theta1)^2*cos(theta3)*cos(theta4)^2*sin(theta3) + 6.28*thetad4*cos(theta1)^2*cos(theta2)^2*cos(theta4)*sin(theta4) + 6.28*thetad4*cos(theta1)^2*cos(theta3)^2*cos(theta4)*sin(theta4) + 11.28*thetad4*cos(theta2)^2*cos(theta3)*cos(theta4)^2*sin(theta3) + 11.28*thetad5*cos(theta2)*cos(theta3)^2*cos(theta4)^2*sin(theta2) + 6.28*thetad5*cos(theta1)^2*cos(theta3)*cos(theta4)^2*sin(theta3) + 6.28*thetad5*cos(theta1)^2*cos(theta2)^2*cos(theta4)*sin(theta4) + 11.28*thetad4*cos(theta2)^2*cos(theta3)^2*cos(theta4)*sin(theta4) + 6.28*thetad5*cos(theta1)^2*cos(theta3)^2*cos(theta4)*sin(theta4) + 11.28*thetad5*cos(theta2)^2*cos(theta3)*cos(theta4)^2*sin(theta3) + 11.28*thetad5*cos(theta2)^2*cos(theta3)^2*cos(theta4)*sin(theta4) + 0.0098*thetad1*cos(theta2)*cos(theta3)*cos(theta4)*cos(theta5) - 0.35*thetad1*cos(theta1)*cos(theta2)*cos(theta3)*sin(theta4) - 0.35*thetad1*cos(theta1)*cos(theta2)*cos(theta4)*sin(theta3) - 0.35*thetad1*cos(theta1)*cos(theta3)*cos(theta4)*sin(theta2) - 0.35*thetad2*cos(theta1)*cos(theta2)*cos(theta3)*sin(theta4) - 0.35*thetad2*cos(theta1)*cos(theta2)*cos(theta4)*sin(theta3) - 0.35*thetad2*cos(theta1)*cos(theta3)*cos(theta4)*sin(theta2) - 0.35*thetad3*cos(theta1)*cos(theta2)*cos(theta3)*sin(theta4) - 0.35*thetad3*cos(theta1)*cos(theta2)*cos(theta4)*sin(theta3) - 0.35*thetad3*cos(theta1)*cos(theta3)*cos(theta4)*sin(theta2) - 0.049*thetad1*cos(theta2)*cos(theta3)*cos(theta4)*sin(theta5) + 0.8*thetad4*cos(theta1)*cos(theta2)^2*cos(theta3)^2*cos(theta4)^2 + 0.8*thetad5*cos(theta1)*cos(theta2)^2*cos(theta3)^2*cos(theta4)^2 - 0.88*thetad4*cos(theta1)*cos(theta2)*sin(theta1)*sin(theta2) + 0.05*thetad1*cos(theta2)*cos(theta3)*sin(theta1)*sin(theta4) + 0.05*thetad1*cos(theta2)*cos(theta4)*sin(theta1)*sin(theta3) + 0.05*thetad1*cos(theta3)*cos(theta4)*sin(theta1)*sin(theta2) - 0.88*thetad5*cos(theta1)*cos(theta2)*sin(theta1)*sin(theta2) + 0.05*thetad2*cos(theta2)*cos(theta3)*sin(theta1)*sin(theta4) + 0.05*thetad2*cos(theta2)*cos(theta4)*sin(theta1)*sin(theta3) + 0.05*thetad2*cos(theta3)*cos(theta4)*sin(theta1)*sin(theta2) - 0.88*thetad4*cos(theta1)*cos(theta3)*sin(theta1)*sin(theta3) + 0.05*thetad3*cos(theta2)*cos(theta3)*sin(theta1)*sin(theta4) + 0.05*thetad3*cos(theta2)*cos(theta4)*sin(theta1)*sin(theta3) + 0.05*thetad3*cos(theta3)*cos(theta4)*sin(theta1)*sin(theta2) - 0.88*thetad5*cos(theta1)*cos(theta3)*sin(theta1)*sin(theta3) - 0.88*thetad4*cos(theta1)*cos(theta4)*sin(theta1)*sin(theta4) - 0.0098*thetad1*cos(theta2)*cos(theta5)*sin(theta3)*sin(theta4) - 0.0098*thetad1*cos(theta3)*cos(theta5)*sin(theta2)*sin(theta4) - 0.0098*thetad1*cos(theta4)*cos(theta5)*sin(theta2)*sin(theta3) - 0.88*thetad5*cos(theta1)*cos(theta4)*sin(theta1)*sin(theta4) + 5.6*thetad4*cos(theta2)^2*cos(theta3)^2*cos(theta4)^2*sin(theta1) + 5.6*thetad5*cos(theta2)^2*cos(theta3)^2*cos(theta4)^2*sin(theta1) + 0.35*thetad1*cos(theta1)*sin(theta2)*sin(theta3)*sin(theta4) + 0.35*thetad2*cos(theta1)*sin(theta2)*sin(theta3)*sin(theta4) + 0.35*thetad3*cos(theta1)*sin(theta2)*sin(theta3)*sin(theta4) + 0.049*thetad1*cos(theta2)*sin(theta3)*sin(theta4)*sin(theta5) + 0.049*thetad1*cos(theta3)*sin(theta2)*sin(theta4)*sin(theta5) + 0.049*thetad1*cos(theta4)*sin(theta2)*sin(theta3)*sin(theta5) - 0.05*thetad1*sin(theta1)*sin(theta2)*sin(theta3)*sin(theta4) - 0.05*thetad2*sin(theta1)*sin(theta2)*sin(theta3)*sin(theta4) - 0.05*thetad3*sin(theta1)*sin(theta2)*sin(theta3)*sin(theta4) - 0.44*thetad1*cos(theta1)^2*cos(theta2)*cos(theta3)*cos(theta4) - 0.44*thetad2*cos(theta1)^2*cos(theta2)*cos(theta3)*cos(theta4) - 0.44*thetad3*cos(theta1)^2*cos(theta2)*cos(theta3)*cos(theta4) + 0.44*thetad1*cos(theta1)^2*cos(theta2)*sin(theta3)*sin(theta4) + 0.44*thetad1*cos(theta1)^2*cos(theta3)*sin(theta2)*sin(theta4) + 0.44*thetad1*cos(theta1)^2*cos(theta4)*sin(theta2)*sin(theta3) + 0.44*thetad2*cos(theta1)^2*cos(theta2)*sin(theta3)*sin(theta4) + 0.44*thetad2*cos(theta1)^2*cos(theta3)*sin(theta2)*sin(theta4) + 0.44*thetad2*cos(theta1)^2*cos(theta4)*sin(theta2)*sin(theta3) + 0.44*thetad3*cos(theta1)^2*cos(theta2)*sin(theta3)*sin(theta4) + 0.44*thetad3*cos(theta1)^2*cos(theta3)*sin(theta2)*sin(theta4) + 0.44*thetad3*cos(theta1)^2*cos(theta4)*sin(theta2)*sin(theta3) + 1.57*thetad1*cos(theta1)*cos(theta2)*cos(theta3)*cos(theta4)*sin(theta1) + 1.57*thetad2*cos(theta1)*cos(theta2)*cos(theta3)*cos(theta4)*sin(theta1) + 1.57*thetad3*cos(theta1)*cos(theta2)*cos(theta3)*cos(theta4)*sin(theta1) + 0.4*thetad4*cos(theta1)*cos(theta2)*cos(theta3)*sin(theta2)*sin(theta3) + 0.4*thetad5*cos(theta1)*cos(theta2)*cos(theta3)*sin(theta2)*sin(theta3) + 0.4*thetad4*cos(theta1)*cos(theta2)*cos(theta4)*sin(theta2)*sin(theta4) + 0.4*thetad5*cos(theta1)*cos(theta2)*cos(theta4)*sin(theta2)*sin(theta4) + 0.4*thetad4*cos(theta1)*cos(theta3)*cos(theta4)*sin(theta3)*sin(theta4) + 0.4*thetad5*cos(theta1)*cos(theta3)*cos(theta4)*sin(theta3)*sin(theta4) - 12.56*thetad4*cos(theta1)^2*cos(theta2)*cos(theta3)^2*cos(theta4)^2*sin(theta2) - 12.56*thetad4*cos(theta1)^2*cos(theta2)^2*cos(theta3)*cos(theta4)^2*sin(theta3) - 12.56*thetad5*cos(theta1)^2*cos(theta2)*cos(theta3)^2*cos(theta4)^2*sin(theta2) - 12.56*thetad4*cos(theta1)^2*cos(theta2)^2*cos(theta3)^2*cos(theta4)*sin(theta4) - 12.56*thetad5*cos(theta1)^2*cos(theta2)^2*cos(theta3)*cos(theta4)^2*sin(theta3) - 12.56*thetad5*cos(theta1)^2*cos(theta2)^2*cos(theta3)^2*cos(theta4)*sin(theta4) - 1.57*thetad1*cos(theta1)*cos(theta2)*sin(theta1)*sin(theta3)*sin(theta4) - 1.57*thetad1*cos(theta1)*cos(theta3)*sin(theta1)*sin(theta2)*sin(theta4) - 1.57*thetad1*cos(theta1)*cos(theta4)*sin(theta1)*sin(theta2)*sin(theta3) - 1.57*thetad2*cos(theta1)*cos(theta2)*sin(theta1)*sin(theta3)*sin(theta4) - 1.57*thetad2*cos(theta1)*cos(theta3)*sin(theta1)*sin(theta2)*sin(theta4) - 1.57*thetad2*cos(theta1)*cos(theta4)*sin(theta1)*sin(theta2)*sin(theta3) - 1.57*thetad3*cos(theta1)*cos(theta2)*sin(theta1)*sin(theta3)*sin(theta4) - 1.57*thetad3*cos(theta1)*cos(theta3)*sin(theta1)*sin(theta2)*sin(theta4) - 1.57*thetad3*cos(theta1)*cos(theta4)*sin(theta1)*sin(theta2)*sin(theta3) + 2.8*thetad4*cos(theta2)*cos(theta3)*sin(theta1)*sin(theta2)*sin(theta3) + 2.8*thetad5*cos(theta2)*cos(theta3)*sin(theta1)*sin(theta2)*sin(theta3) + 2.8*thetad4*cos(theta2)*cos(theta4)*sin(theta1)*sin(theta2)*sin(theta4) + 2.8*thetad5*cos(theta2)*cos(theta4)*sin(theta1)*sin(theta2)*sin(theta4) + 2.8*thetad4*cos(theta3)*cos(theta4)*sin(theta1)*sin(theta3)*sin(theta4) + 2.8*thetad5*cos(theta3)*cos(theta4)*sin(theta1)*sin(theta3)*sin(theta4) + 1.76*thetad4*cos(theta1)*cos(theta2)*cos(theta3)^2*sin(theta1)*sin(theta2) + 1.76*thetad4*cos(theta1)*cos(theta2)*cos(theta4)^2*sin(theta1)*sin(theta2) + 1.76*thetad4*cos(theta1)*cos(theta2)^2*cos(theta3)*sin(theta1)*sin(theta3) + 1.76*thetad5*cos(theta1)*cos(theta2)*cos(theta3)^2*sin(theta1)*sin(theta2) + 1.76*thetad5*cos(theta1)*cos(theta2)*cos(theta4)^2*sin(theta1)*sin(theta2) + 1.76*thetad5*cos(theta1)*cos(theta2)^2*cos(theta3)*sin(theta1)*sin(theta3) + 1.76*thetad4*cos(theta1)*cos(theta3)*cos(theta4)^2*sin(theta1)*sin(theta3) + 1.76*thetad4*cos(theta1)*cos(theta2)^2*cos(theta4)*sin(theta1)*sin(theta4) + 1.76*thetad4*cos(theta1)*cos(theta3)^2*cos(theta4)*sin(theta1)*sin(theta4) + 1.76*thetad5*cos(theta1)*cos(theta3)*cos(theta4)^2*sin(theta1)*sin(theta3) + 1.76*thetad5*cos(theta1)*cos(theta2)^2*cos(theta4)*sin(theta1)*sin(theta4) + 1.76*thetad5*cos(theta1)*cos(theta3)^2*cos(theta4)*sin(theta1)*sin(theta4) - 11.28*thetad4*cos(theta2)*cos(theta3)*cos(theta4)*sin(theta2)*sin(theta3)*sin(theta4) - 11.28*thetad5*cos(theta2)*cos(theta3)*cos(theta4)*sin(theta2)*sin(theta3)*sin(theta4) - 0.8*thetad4*cos(theta1)*cos(theta2)*cos(theta3)*cos(theta4)^2*sin(theta2)*sin(theta3) - 0.8*thetad4*cos(theta1)*cos(theta2)*cos(theta3)^2*cos(theta4)*sin(theta2)*sin(theta4) - 0.8*thetad5*cos(theta1)*cos(theta2)*cos(theta3)*cos(theta4)^2*sin(theta2)*sin(theta3) - 0.8*thetad4*cos(theta1)*cos(theta2)^2*cos(theta3)*cos(theta4)*sin(theta3)*sin(theta4) - 0.8*thetad5*cos(theta1)*cos(theta2)*cos(theta3)^2*cos(theta4)*sin(theta2)*sin(theta4) - 0.8*thetad5*cos(theta1)*cos(theta2)^2*cos(theta3)*cos(theta4)*sin(theta3)*sin(theta4) - 5.6*thetad4*cos(theta2)*cos(theta3)*cos(theta4)^2*sin(theta1)*sin(theta2)*sin(theta3) - 5.6*thetad4*cos(theta2)*cos(theta3)^2*cos(theta4)*sin(theta1)*sin(theta2)*sin(theta4) - 5.6*thetad5*cos(theta2)*cos(theta3)*cos(theta4)^2*sin(theta1)*sin(theta2)*sin(theta3) - 5.6*thetad4*cos(theta2)^2*cos(theta3)*cos(theta4)*sin(theta1)*sin(theta3)*sin(theta4) - 5.6*thetad5*cos(theta2)*cos(theta3)^2*cos(theta4)*sin(theta1)*sin(theta2)*sin(theta4) - 5.6*thetad5*cos(theta2)^2*cos(theta3)*cos(theta4)*sin(theta1)*sin(theta3)*sin(theta4) - 3.52*thetad4*cos(theta1)*cos(theta2)*cos(theta3)^2*cos(theta4)^2*sin(theta1)*sin(theta2) - 3.52*thetad4*cos(theta1)*cos(theta2)^2*cos(theta3)*cos(theta4)^2*sin(theta1)*sin(theta3) - 3.52*thetad5*cos(theta1)*cos(theta2)*cos(theta3)^2*cos(theta4)^2*sin(theta1)*sin(theta2) - 3.52*thetad4*cos(theta1)*cos(theta2)^2*cos(theta3)^2*cos(theta4)*sin(theta1)*sin(theta4) - 3.52*thetad5*cos(theta1)*cos(theta2)^2*cos(theta3)*cos(theta4)^2*sin(theta1)*sin(theta3) - 3.52*thetad5*cos(theta1)*cos(theta2)^2*cos(theta3)^2*cos(theta4)*sin(theta1)*sin(theta4) + 12.56*thetad4*cos(theta1)^2*cos(theta2)*cos(theta3)*cos(theta4)*sin(theta2)*sin(theta3)*sin(theta4) + 12.56*thetad5*cos(theta1)^2*cos(theta2)*cos(theta3)*cos(theta4)*sin(theta2)*sin(theta3)*sin(theta4) + 3.52*thetad4*cos(theta1)*cos(theta2)*cos(theta3)*cos(theta4)*sin(theta1)*sin(theta2)*sin(theta3)*sin(theta4) + 3.52*thetad5*cos(theta1)*cos(theta2)*cos(theta3)*cos(theta4)*sin(theta1)*sin(theta2)*sin(theta3)*sin(theta4) ;
C(5,1) = 0.028*thetad1 - 0.028*thetad1*cos(theta2)^2 - 0.028*thetad1*cos(theta3)^2 - 0.028*thetad1*cos(theta4)^2 - 0.056*thetad1*cos(theta5)^2 + 0.056*thetad1*cos(theta2)^2*cos(theta3)^2 + 0.056*thetad1*cos(theta2)^2*cos(theta4)^2 + 0.056*thetad1*cos(theta2)^2*cos(theta5)^2 + 0.056*thetad1*cos(theta3)^2*cos(theta4)^2 + 0.056*thetad1*cos(theta3)^2*cos(theta5)^2 + 0.056*thetad1*cos(theta4)^2*cos(theta5)^2 + 0.14*thetad1*cos(theta4)*cos(theta5) + 0.07*thetad5*cos(theta2)*cos(theta5) - 0.014*thetad2*cos(theta5)*sin(theta2) + 0.028*thetad1*cos(theta4)*sin(theta5) + 0.1344*thetad1*cos(theta5)*sin(theta5) + 0.014*thetad5*cos(theta2)*sin(theta5) + 0.07*thetad2*sin(theta2)*sin(theta5) + 0.07*thetad5*cos(theta2)*cos(theta3)*cos(theta5) - 0.098*thetad1*cos(theta2)*cos(theta5)*sin(theta2) - 0.0672*thetad2*cos(theta2)*cos(theta3)*sin(theta4) - 0.0672*thetad2*cos(theta2)*cos(theta4)*sin(theta3) - 0.0672*thetad2*cos(theta3)*cos(theta4)*sin(theta2) - 0.098*thetad1*cos(theta3)*cos(theta5)*sin(theta3) - 0.014*thetad2*cos(theta2)*cos(theta5)*sin(theta3) - 0.014*thetad2*cos(theta3)*cos(theta5)*sin(theta2) - 0.0672*thetad3*cos(theta2)*cos(theta3)*sin(theta4) - 0.0672*thetad3*cos(theta2)*cos(theta4)*sin(theta3) - 0.0672*thetad3*cos(theta3)*cos(theta4)*sin(theta2) - 0.014*thetad3*cos(theta2)*cos(theta5)*sin(theta3) - 0.014*thetad3*cos(theta3)*cos(theta5)*sin(theta2) - 0.0672*thetad4*cos(theta2)*cos(theta3)*sin(theta4) - 0.0672*thetad4*cos(theta2)*cos(theta4)*sin(theta3) - 0.0672*thetad4*cos(theta3)*cos(theta4)*sin(theta2) - 0.098*thetad1*cos(theta4)*cos(theta5)*sin(theta4) + 0.014*thetad5*cos(theta2)*cos(theta3)*sin(theta5) - 0.112*thetad1*cos(theta2)^2*cos(theta3)^2*cos(theta4)^2 - 0.112*thetad1*cos(theta2)^2*cos(theta3)^2*cos(theta5)^2 - 0.112*thetad1*cos(theta2)^2*cos(theta4)^2*cos(theta5)^2 - 0.112*thetad1*cos(theta3)^2*cos(theta4)^2*cos(theta5)^2 - 0.0196*thetad1*cos(theta2)*sin(theta2)*sin(theta5) - 0.0196*thetad1*cos(theta3)*sin(theta3)*sin(theta5) + 0.07*thetad2*cos(theta2)*sin(theta3)*sin(theta5) + 0.07*thetad2*cos(theta3)*sin(theta2)*sin(theta5) + 0.07*thetad3*cos(theta2)*sin(theta3)*sin(theta5) + 0.07*thetad3*cos(theta3)*sin(theta2)*sin(theta5) - 0.0196*thetad1*cos(theta4)*sin(theta4)*sin(theta5) - 0.07*thetad5*cos(theta5)*sin(theta2)*sin(theta3) + 0.0672*thetad2*sin(theta2)*sin(theta3)*sin(theta4) + 0.0672*thetad3*sin(theta2)*sin(theta3)*sin(theta4) + 0.0672*thetad4*sin(theta2)*sin(theta3)*sin(theta4) - 0.014*thetad5*sin(theta2)*sin(theta3)*sin(theta5) - 0.14*thetad1*cos(theta2)^2*cos(theta4)*cos(theta5) - 0.14*thetad1*cos(theta3)^2*cos(theta4)*cos(theta5) - 0.028*thetad1*cos(theta2)^2*cos(theta4)*sin(theta5) - 0.1344*thetad1*cos(theta2)^2*cos(theta5)*sin(theta5) - 0.028*thetad1*cos(theta3)^2*cos(theta4)*sin(theta5) - 0.1344*thetad1*cos(theta3)^2*cos(theta5)*sin(theta5) - 0.1344*thetad1*cos(theta4)^2*cos(theta5)*sin(theta5) + 0.056*thetad1*cos(theta2)^2*cos(theta3)^2*cos(theta4)*sin(theta5) + 0.2688*thetad1*cos(theta2)^2*cos(theta3)^2*cos(theta5)*sin(theta5) + 0.2688*thetad1*cos(theta2)^2*cos(theta4)^2*cos(theta5)*sin(theta5) + 0.2688*thetad1*cos(theta3)^2*cos(theta4)^2*cos(theta5)*sin(theta5) - 0.0098*thetad2*cos(theta2)*cos(theta3)*cos(theta4)*cos(theta5) - 0.0098*thetad3*cos(theta2)*cos(theta3)*cos(theta4)*cos(theta5) - 0.0098*thetad4*cos(theta2)*cos(theta3)*cos(theta4)*cos(theta5) + 0.049*thetad2*cos(theta2)*cos(theta3)*cos(theta4)*sin(theta5) + 0.049*thetad3*cos(theta2)*cos(theta3)*cos(theta4)*sin(theta5) + 0.049*thetad4*cos(theta2)*cos(theta3)*cos(theta4)*sin(theta5) - 0.049*thetad5*cos(theta2)*cos(theta3)*cos(theta5)*sin(theta4) - 0.049*thetad5*cos(theta2)*cos(theta4)*cos(theta5)*sin(theta3) - 0.049*thetad5*cos(theta3)*cos(theta4)*cos(theta5)*sin(theta2) - 0.056*thetad1*cos(theta2)*cos(theta3)*sin(theta2)*sin(theta3) - 0.056*thetad1*cos(theta2)*cos(theta4)*sin(theta2)*sin(theta4) + 0.14*thetad1*cos(theta2)*cos(theta5)*sin(theta2)*sin(theta4) - 0.056*thetad1*cos(theta3)*cos(theta4)*sin(theta3)*sin(theta4) + 0.14*thetad1*cos(theta3)*cos(theta5)*sin(theta3)*sin(theta4) + 0.0098*thetad2*cos(theta2)*cos(theta5)*sin(theta3)*sin(theta4) + 0.0098*thetad2*cos(theta3)*cos(theta5)*sin(theta2)*sin(theta4) + 0.0098*thetad2*cos(theta4)*cos(theta5)*sin(theta2)*sin(theta3) + 0.0098*thetad3*cos(theta2)*cos(theta5)*sin(theta3)*sin(theta4) + 0.0098*thetad3*cos(theta3)*cos(theta5)*sin(theta2)*sin(theta4) + 0.0098*thetad3*cos(theta4)*cos(theta5)*sin(theta2)*sin(theta3) + 0.0098*thetad4*cos(theta2)*cos(theta5)*sin(theta3)*sin(theta4) + 0.0098*thetad4*cos(theta3)*cos(theta5)*sin(theta2)*sin(theta4) + 0.0098*thetad4*cos(theta4)*cos(theta5)*sin(theta2)*sin(theta3) - 0.0098*thetad5*cos(theta2)*cos(theta3)*sin(theta4)*sin(theta5) - 0.0098*thetad5*cos(theta2)*cos(theta4)*sin(theta3)*sin(theta5) - 0.0098*thetad5*cos(theta3)*cos(theta4)*sin(theta2)*sin(theta5) + 0.028*thetad1*cos(theta2)*sin(theta2)*sin(theta4)*sin(theta5) + 0.028*thetad1*cos(theta3)*sin(theta3)*sin(theta4)*sin(theta5) - 0.049*thetad2*cos(theta2)*sin(theta3)*sin(theta4)*sin(theta5) - 0.049*thetad2*cos(theta3)*sin(theta2)*sin(theta4)*sin(theta5) - 0.049*thetad2*cos(theta4)*sin(theta2)*sin(theta3)*sin(theta5) - 0.049*thetad3*cos(theta2)*sin(theta3)*sin(theta4)*sin(theta5) - 0.049*thetad3*cos(theta3)*sin(theta2)*sin(theta4)*sin(theta5) - 0.049*thetad3*cos(theta4)*sin(theta2)*sin(theta3)*sin(theta5) - 0.049*thetad4*cos(theta2)*sin(theta3)*sin(theta4)*sin(theta5) - 0.049*thetad4*cos(theta3)*sin(theta2)*sin(theta4)*sin(theta5) - 0.049*thetad4*cos(theta4)*sin(theta2)*sin(theta3)*sin(theta5) + 0.049*thetad5*cos(theta5)*sin(theta2)*sin(theta3)*sin(theta4) + 0.0098*thetad5*sin(theta2)*sin(theta3)*sin(theta4)*sin(theta5) + 0.14*thetad1*cos(theta2)^2*cos(theta3)*cos(theta4)*cos(theta5) + 0.196*thetad1*cos(theta2)*cos(theta3)^2*cos(theta5)*sin(theta2) + 0.196*thetad1*cos(theta2)*cos(theta4)^2*cos(theta5)*sin(theta2) + 0.196*thetad1*cos(theta2)^2*cos(theta3)*cos(theta5)*sin(theta3) + 0.028*thetad1*cos(theta2)^2*cos(theta3)*cos(theta4)*sin(theta5) + 0.196*thetad1*cos(theta3)*cos(theta4)^2*cos(theta5)*sin(theta3) + 0.196*thetad1*cos(theta2)^2*cos(theta4)*cos(theta5)*sin(theta4) + 0.1344*thetad2*cos(theta2)*cos(theta3)*cos(theta5)^2*sin(theta4) + 0.1344*thetad2*cos(theta2)*cos(theta4)*cos(theta5)^2*sin(theta3) + 0.1344*thetad2*cos(theta3)*cos(theta4)*cos(theta5)^2*sin(theta2) + 0.196*thetad1*cos(theta3)^2*cos(theta4)*cos(theta5)*sin(theta4) + 0.1344*thetad3*cos(theta2)*cos(theta3)*cos(theta5)^2*sin(theta4) + 0.1344*thetad3*cos(theta2)*cos(theta4)*cos(theta5)^2*sin(theta3) + 0.1344*thetad3*cos(theta3)*cos(theta4)*cos(theta5)^2*sin(theta2) + 0.1344*thetad4*cos(theta2)*cos(theta3)*cos(theta5)^2*sin(theta4) + 0.1344*thetad4*cos(theta2)*cos(theta4)*cos(theta5)^2*sin(theta3) + 0.1344*thetad4*cos(theta3)*cos(theta4)*cos(theta5)^2*sin(theta2) + 0.224*thetad1*cos(theta2)^2*cos(theta3)^2*cos(theta4)^2*cos(theta5)^2 + 0.0392*thetad1*cos(theta2)*cos(theta3)^2*sin(theta2)*sin(theta5) + 0.0392*thetad1*cos(theta2)*cos(theta4)^2*sin(theta2)*sin(theta5) + 0.0392*thetad1*cos(theta2)^2*cos(theta3)*sin(theta3)*sin(theta5) - 0.14*thetad1*cos(theta2)^2*cos(theta5)*sin(theta3)*sin(theta4) + 0.0392*thetad1*cos(theta3)*cos(theta4)^2*sin(theta3)*sin(theta5) + 0.0392*thetad1*cos(theta2)^2*cos(theta4)*sin(theta4)*sin(theta5) + 0.0392*thetad1*cos(theta3)^2*cos(theta4)*sin(theta4)*sin(theta5) - 0.028*thetad1*cos(theta2)^2*sin(theta3)*sin(theta4)*sin(theta5) - 0.1344*thetad2*cos(theta5)^2*sin(theta2)*sin(theta3)*sin(theta4) - 0.1344*thetad3*cos(theta5)^2*sin(theta2)*sin(theta3)*sin(theta4) - 0.1344*thetad4*cos(theta5)^2*sin(theta2)*sin(theta3)*sin(theta4) + 0.28*thetad1*cos(theta2)^2*cos(theta3)^2*cos(theta4)*cos(theta5) - 0.14*thetad1*cos(theta2)*cos(theta3)*cos(theta5)*sin(theta2)*sin(theta4) - 0.14*thetad1*cos(theta2)*cos(theta4)*cos(theta5)*sin(theta2)*sin(theta3) + 0.056*thetad2*cos(theta2)*cos(theta3)*cos(theta5)*sin(theta4)*sin(theta5) + 0.056*thetad2*cos(theta2)*cos(theta4)*cos(theta5)*sin(theta3)*sin(theta5) + 0.056*thetad2*cos(theta3)*cos(theta4)*cos(theta5)*sin(theta2)*sin(theta5) + 0.056*thetad3*cos(theta2)*cos(theta3)*cos(theta5)*sin(theta4)*sin(theta5) + 0.056*thetad3*cos(theta2)*cos(theta4)*cos(theta5)*sin(theta3)*sin(theta5) + 0.056*thetad3*cos(theta3)*cos(theta4)*cos(theta5)*sin(theta2)*sin(theta5) + 0.056*thetad4*cos(theta2)*cos(theta3)*cos(theta5)*sin(theta4)*sin(theta5) + 0.056*thetad4*cos(theta2)*cos(theta4)*cos(theta5)*sin(theta3)*sin(theta5) + 0.056*thetad4*cos(theta3)*cos(theta4)*cos(theta5)*sin(theta2)*sin(theta5) - 0.5376*thetad1*cos(theta2)^2*cos(theta3)^2*cos(theta4)^2*cos(theta5)*sin(theta5) - 0.028*thetad1*cos(theta2)*cos(theta3)*sin(theta2)*sin(theta4)*sin(theta5) - 0.028*thetad1*cos(theta2)*cos(theta4)*sin(theta2)*sin(theta3)*sin(theta5) - 0.056*thetad2*cos(theta5)*sin(theta2)*sin(theta3)*sin(theta4)*sin(theta5) - 0.056*thetad3*cos(theta5)*sin(theta2)*sin(theta3)*sin(theta4)*sin(theta5) - 0.056*thetad4*cos(theta5)*sin(theta2)*sin(theta3)*sin(theta4)*sin(theta5) + 0.112*thetad1*cos(theta2)*cos(theta3)*cos(theta4)^2*sin(theta2)*sin(theta3) + 0.112*thetad1*cos(theta2)*cos(theta3)*cos(theta5)^2*sin(theta2)*sin(theta3) + 0.112*thetad1*cos(theta2)*cos(theta3)^2*cos(theta4)*sin(theta2)*sin(theta4) - 0.28*thetad1*cos(theta2)*cos(theta3)^2*cos(theta5)*sin(theta2)*sin(theta4) + 0.112*thetad1*cos(theta2)^2*cos(theta3)*cos(theta4)*sin(theta3)*sin(theta4) + 0.112*thetad1*cos(theta2)*cos(theta4)*cos(theta5)^2*sin(theta2)*sin(theta4) - 0.28*thetad1*cos(theta2)^2*cos(theta3)*cos(theta5)*sin(theta3)*sin(theta4) + 0.112*thetad1*cos(theta3)*cos(theta4)*cos(theta5)^2*sin(theta3)*sin(theta4) - 0.056*thetad1*cos(theta2)*cos(theta3)^2*sin(theta2)*sin(theta4)*sin(theta5) - 0.056*thetad1*cos(theta2)^2*cos(theta3)*sin(theta3)*sin(theta4)*sin(theta5) - 0.392*thetad1*cos(theta2)*cos(theta3)^2*cos(theta4)^2*cos(theta5)*sin(theta2) - 0.392*thetad1*cos(theta2)^2*cos(theta3)*cos(theta4)^2*cos(theta5)*sin(theta3) - 0.392*thetad1*cos(theta2)^2*cos(theta3)^2*cos(theta4)*cos(theta5)*sin(theta4) - 0.0784*thetad1*cos(theta2)*cos(theta3)^2*cos(theta4)^2*sin(theta2)*sin(theta5) - 0.0784*thetad1*cos(theta2)^2*cos(theta3)*cos(theta4)^2*sin(theta3)*sin(theta5) - 0.0784*thetad1*cos(theta2)^2*cos(theta3)^2*cos(theta4)*sin(theta4)*sin(theta5) - 0.28*thetad1*cos(theta2)*cos(theta3)*cos(theta4)*cos(theta5)*sin(theta2)*sin(theta3) - 0.056*thetad1*cos(theta2)*cos(theta3)*cos(theta4)*sin(theta2)*sin(theta3)*sin(theta5) - 0.2688*thetad1*cos(theta2)*cos(theta3)*cos(theta5)*sin(theta2)*sin(theta3)*sin(theta5) - 0.2688*thetad1*cos(theta2)*cos(theta4)*cos(theta5)*sin(theta2)*sin(theta4)*sin(theta5) - 0.2688*thetad1*cos(theta3)*cos(theta4)*cos(theta5)*sin(theta3)*sin(theta4)*sin(theta5) - 0.224*thetad1*cos(theta2)*cos(theta3)*cos(theta4)^2*cos(theta5)^2*sin(theta2)*sin(theta3) - 0.224*thetad1*cos(theta2)*cos(theta3)^2*cos(theta4)*cos(theta5)^2*sin(theta2)*sin(theta4) - 0.224*thetad1*cos(theta2)^2*cos(theta3)*cos(theta4)*cos(theta5)^2*sin(theta3)*sin(theta4) + 0.5376*thetad1*cos(theta2)*cos(theta3)*cos(theta4)^2*cos(theta5)*sin(theta2)*sin(theta3)*sin(theta5) + 0.5376*thetad1*cos(theta2)*cos(theta3)^2*cos(theta4)*cos(theta5)*sin(theta2)*sin(theta4)*sin(theta5) + 0.5376*thetad1*cos(theta2)^2*cos(theta3)*cos(theta4)*cos(theta5)*sin(theta3)*sin(theta4)*sin(theta5) + 0.392*thetad1*cos(theta2)*cos(theta3)*cos(theta4)*cos(theta5)*sin(theta2)*sin(theta3)*sin(theta4) + 0.0784*thetad1*cos(theta2)*cos(theta3)*cos(theta4)*sin(theta2)*sin(theta3)*sin(theta4)*sin(theta5) ;
C(5,2) = 0.056*thetad2*cos(theta5)^2 - 0.028*thetad3 - 0.028*thetad4 - 0.028*thetad2 + 0.056*thetad3*cos(theta5)^2 + 0.056*thetad4*cos(theta5)^2 - 0.0098*thetad5*cos(theta5) + 0.049*thetad5*sin(theta5) + 0.14*thetad2*cos(theta4)*cos(theta5) + 0.14*thetad3*cos(theta4)*cos(theta5) + 0.07*thetad4*cos(theta4)*cos(theta5) - 0.014*thetad1*cos(theta5)*sin(theta2) + 0.028*thetad2*cos(theta4)*sin(theta5) - 0.1344*thetad2*cos(theta5)*sin(theta5) + 0.028*thetad3*cos(theta4)*sin(theta5) - 0.1344*thetad3*cos(theta5)*sin(theta5) + 0.014*thetad4*cos(theta4)*sin(theta5) - 0.1344*thetad4*cos(theta5)*sin(theta5) + 0.014*thetad5*cos(theta5)*sin(theta4) + 0.07*thetad1*sin(theta2)*sin(theta5) - 0.07*thetad5*sin(theta4)*sin(theta5) + 0.14*thetad2*cos(theta3)*cos(theta4)*cos(theta5) + 0.07*thetad3*cos(theta3)*cos(theta4)*cos(theta5) + 0.07*thetad4*cos(theta3)*cos(theta4)*cos(theta5) - 0.0672*thetad1*cos(theta2)*cos(theta3)*sin(theta4) - 0.0672*thetad1*cos(theta2)*cos(theta4)*sin(theta3) - 0.0672*thetad1*cos(theta3)*cos(theta4)*sin(theta2) - 0.014*thetad1*cos(theta2)*cos(theta5)*sin(theta3) - 0.014*thetad1*cos(theta3)*cos(theta5)*sin(theta2) + 0.028*thetad2*cos(theta3)*cos(theta4)*sin(theta5) + 0.014*thetad3*cos(theta3)*cos(theta4)*sin(theta5) + 0.014*thetad4*cos(theta3)*cos(theta4)*sin(theta5) + 0.014*thetad5*cos(theta3)*cos(theta5)*sin(theta4) + 0.014*thetad5*cos(theta4)*cos(theta5)*sin(theta3) + 0.07*thetad1*cos(theta2)*sin(theta3)*sin(theta5) + 0.07*thetad1*cos(theta3)*sin(theta2)*sin(theta5) - 0.14*thetad2*cos(theta5)*sin(theta3)*sin(theta4) - 0.07*thetad3*cos(theta5)*sin(theta3)*sin(theta4) - 0.07*thetad4*cos(theta5)*sin(theta3)*sin(theta4) - 0.07*thetad5*cos(theta3)*sin(theta4)*sin(theta5) - 0.07*thetad5*cos(theta4)*sin(theta3)*sin(theta5) + 0.0672*thetad1*sin(theta2)*sin(theta3)*sin(theta4) - 0.028*thetad2*sin(theta3)*sin(theta4)*sin(theta5) - 0.014*thetad3*sin(theta3)*sin(theta4)*sin(theta5) - 0.014*thetad4*sin(theta3)*sin(theta4)*sin(theta5) - 0.0098*thetad1*cos(theta2)*cos(theta3)*cos(theta4)*cos(theta5) + 0.049*thetad1*cos(theta2)*cos(theta3)*cos(theta4)*sin(theta5) + 0.0098*thetad1*cos(theta2)*cos(theta5)*sin(theta3)*sin(theta4) + 0.0098*thetad1*cos(theta3)*cos(theta5)*sin(theta2)*sin(theta4) + 0.0098*thetad1*cos(theta4)*cos(theta5)*sin(theta2)*sin(theta3) - 0.049*thetad1*cos(theta2)*sin(theta3)*sin(theta4)*sin(theta5) - 0.049*thetad1*cos(theta3)*sin(theta2)*sin(theta4)*sin(theta5) - 0.049*thetad1*cos(theta4)*sin(theta2)*sin(theta3)*sin(theta5) + 0.1344*thetad1*cos(theta2)*cos(theta3)*cos(theta5)^2*sin(theta4) + 0.1344*thetad1*cos(theta2)*cos(theta4)*cos(theta5)^2*sin(theta3) + 0.1344*thetad1*cos(theta3)*cos(theta4)*cos(theta5)^2*sin(theta2) - 0.1344*thetad1*cos(theta5)^2*sin(theta2)*sin(theta3)*sin(theta4) + 0.056*thetad1*cos(theta2)*cos(theta3)*cos(theta5)*sin(theta4)*sin(theta5) + 0.056*thetad1*cos(theta2)*cos(theta4)*cos(theta5)*sin(theta3)*sin(theta5) + 0.056*thetad1*cos(theta3)*cos(theta4)*cos(theta5)*sin(theta2)*sin(theta5) - 0.056*thetad1*cos(theta5)*sin(theta2)*sin(theta3)*sin(theta4)*sin(theta5) ;
